simulink model "Simulation_in_Simulink"  (R2021b)
settings: Solver=FixedStepAuto  StartTime=0.0  StopTime=10  FixedStep=0.02  RelTol=1e-3
(part 2 of 5)

== matlab function Simulation_in_Simulink/C*theta_dot ==
  data: theta input; C_theta_dot output; theta_dot input
function C_theta_dot = fcn(theta,theta_dot)

t1=theta(1);
t2=theta(2);
t3=theta(3);
t4=theta(4);
t5=theta(5);
t6=theta(6);

td1=theta_dot(1);
td2=theta_dot(2);
td3=theta_dot(3);
td4=theta_dot(4);
td5=theta_dot(5);
td6=theta_dot(6);

a2=0.6129;
a3=0.5716; 
d4=0.16389; 
d5=0.1157; 
d6=0.0922;

c11=td5*((49450651*sin(2*t2 + 2*t3 + 2*t4 - t5))/500000000000 - (1966511423*sin(2*t2 + 2*t3 + 2*t4 - 2*t5))/20000000000000 + (1966511423*sin(2*t2 + 2*t3 + 2*t4 + 2*t5))/20000000000000 - (1966511423*sin(2*t5))/10000000000000 + (49450651*sin(2*t2 + 2*t3 + 2*t4 + t5))/500000000000 + (957929*a2*cos(2*t2 + t3 + t4 - t5))/200000000 + (957929*a3*cos(2*t2 + 2*t3 + t4 + t5))/200000000 - (((817*sin(t6)*(cos(t5)*sin(t1) + cos(t2 + t3 + t4)*cos(t1)*sin(t5)))/2000000 - (37539*sin(t1)*sin(t5))/5000000 + (43*d6*(sin(t1)*sin(t5) - cos(t2 + t3 + t4)*cos(t1)*cos(t5)))/100 + (37539*cos(t2 + t3 + t4)*cos(t1)*cos(t5))/5000000)*(d6*(cos(t5)*sin(t1) + cos(t2 + t3 + t4)*cos(t1)*sin(t5)) - (873*cos(t5)*sin(t1))/50000 - (19*sin(t6)*(sin(t1)*sin(t5) - cos(t2 + t3 + t4)*cos(t1)*cos(t5)))/20000 + d4*sin(t1) - (873*cos(t2 + t3 + t4)*cos(t1)*sin(t5))/50000 + (19*sin(t2 + t3 + t4)*cos(t1)*cos(t6))/20000 + a3*cos(t2 + t3)*cos(t1) + a2*cos(t1)*cos(t2) - d5*sin(t2 + t3 + t4)*cos(t1)))/2 - (((19*sin(t6)*(cos(t5)*sin(t1) + cos(t2 + t3 + t4)*cos(t1)*sin(t5)))/20000 - (873*sin(t1)*sin(t5))/50000 + d6*(sin(t1)*sin(t5) - cos(t2 + t3 + t4)*cos(t1)*cos(t5)) + (873*cos(t2 + t3 + t4)*cos(t1)*cos(t5))/50000)*((43*d6*(cos(t5)*sin(t1) + cos(t2 + t3 + t4)*cos(t1)*sin(t5)))/100 - (37539*cos(t5)*sin(t1))/5000000 - (817*sin(t6)*(sin(t1)*sin(t5) - cos(t2 + t3 + t4)*cos(t1)*cos(t5)))/2000000 + (43*d4*sin(t1))/100 - (37539*cos(t2 + t3 + t4)*cos(t1)*sin(t5))/5000000 + (817*sin(t2 + t3 + t4)*cos(t1)*cos(t6))/2000000 + (43*a3*cos(t2 + t3)*cos(t1))/100 + (43*a2*cos(t1)*cos(t2))/100 - (43*d5*sin(t2 + t3 + t4)*cos(t1))/100))/2 + (957929*a2*cos(t3 + t4 - t5))/200000000 + (((817*sin(t6)*(cos(t1)*cos(t5) - cos(t2 + t3 + t4)*sin(t1)*sin(t5)))/2000000 - (37539*cos(t1)*sin(t5))/5000000 + (43*d6*(cos(t1)*sin(t5) + cos(t2 + t3 + t4)*cos(t5)*sin(t1)))/100 - (37539*cos(t2 + t3 + t4)*cos(t5)*sin(t1))/5000000)*((19*sin(t6)*(cos(t1)*sin(t5) + cos(t2 + t3 + t4)*cos(t5)*sin(t1)))/20000 + (873*cos(t1)*cos(t5))/50000 - d6*(cos(t1)*cos(t5) - cos(t2 + t3 + t4)*sin(t1)*sin(t5)) - d4*cos(t1) - (873*cos(t2 + t3 + t4)*sin(t1)*sin(t5))/50000 + (19*sin(t2 + t3 + t4)*cos(t6)*sin(t1))/20000 + a3*cos(t2 + t3)*sin(t1) + a2*cos(t2)*sin(t1) - d5*sin(t2 + t3 + t4)*sin(t1)))/2 + (((19*sin(t6)*(cos(t1)*cos(t5) - cos(t2 + t3 + t4)*sin(t1)*sin(t5)))/20000 - (873*cos(t1)*sin(t5))/50000 + d6*(cos(t1)*sin(t5) + cos(t2 + t3 + t4)*cos(t5)*sin(t1)) - (873*cos(t2 + t3 + t4)*cos(t5)*sin(t1))/50000)*((817*sin(t6)*(cos(t1)*sin(t5) + cos(t2 + t3 + t4)*cos(t5)*sin(t1)))/2000000 + (37539*cos(t1)*cos(t5))/5000000 - (43*d6*(cos(t1)*cos(t5) - cos(t2 + t3 + t4)*sin(t1)*sin(t5)))/100 - (43*d4*cos(t1))/100 - (37539*cos(t2 + t3 + t4)*sin(t1)*sin(t5))/5000000 + (817*sin(t2 + t3 + t4)*cos(t6)*sin(t1))/2000000 + (43*a3*cos(t2 + t3)*sin(t1))/100 + (43*a2*cos(t2)*sin(t1))/100 - (43*d5*sin(t2 + t3 + t4)*sin(t1))/100))/2 + (957929*a3*cos(t4 + t5))/200000000 + (957929*a3*cos(2*t2 + 2*t3 + t4 - t5))/200000000 - (957929*d5*sin(2*t2 + 2*t3 + 2*t4 + t5))/200000000 - (957929*d4*sin(t5))/50000000 + (957929*a2*cos(2*t2 + t3 + t4 + t5))/200000000 + (957929*a3*cos(t4 - t5))/200000000 + (957929*a2*cos(t3 + t4 + t5))/200000000 - (957929*d5*sin(2*t2 + 2*t3 + 2*t4 - t5))/200000000 + (sin(t2 + t3 + t4)^2*cos(t5)*sin(t5))/2500 - (11*sin(t2 + t3 + t4)*cos(t6)*sin(t5)*(cos(t2 + t3 + t4)*sin(t6) + sin(t2 + t3 + t4)*cos(t5)*cos(t6)))/100000 - (sin(t2 + t3 + t4)*cos(t6)*sin(t5)*((11*cos(t2 + t3 + t4)*sin(t6))/50000 + (11*sin(t2 + t3 + t4)*cos(t5)*cos(t6))/50000))/2 + (3*sin(t2 + t3 + t4)*sin(t5)*sin(t6)*(cos(t2 + t3 + t4)*cos(t6) - sin(t2 + t3 + t4)*cos(t5)*sin(t6)))/25000 + (sin(t2 + t3 + t4)*sin(t5)*sin(t6)*((3*cos(t2 + t3 + t4)*cos(t6))/12500 - (3*sin(t2 + t3 + t4)*cos(t5)*sin(t6))/12500))/2) - td3*((49450651*sin(2*t2 + 2*t3 + 2*t4 - t5))/250000000000 - (1966511423*sin(2*t2 + 2*t3 + 2*t4 - 2*t5))/20000000000000 - (1966511423*sin(2*t2 + 2*t3 + 2*t4 + 2*t5))/20000000000000 - (3534581023*sin(2*t2 + 2*t3 + 2*t4))/10000000000000 + (42783*sin(2*t2 + 2*t3))/62500 - (49450651*sin(2*t2 + 2*t3 + 2*t4 + t5))/250000000000 + (37373*d5*sin(2*t2 + 2*t3 + 2*t4))/2500000 + (957929*a2*cos(2*t2 + t3 + t4 - t5))/200000000 - (957929*a3*cos(2*t2 + 2*t3 + t4 + t5))/100000000 + (210469*a2*cos(2*t2 + t3 + t4))/100000000 + (957929*a2*cos(t3 + t4 - t5))/200000000 + (((43*a3*sin(t2 + t3)*sin(t1))/100 - (37539*sin(t2 + t3 + t4)*sin(t1)*sin(t5))/5000000 - (817*cos(t2 + t3 + t4)*cos(t6)*sin(t1))/2000000 + (43*d5*cos(t2 + t3 + t4)*sin(t1))/100 + (817*sin(t2 + t3 + t4)*cos(t5)*sin(t1)*sin(t6))/2000000 + (43*d6*sin(t2 + t3 + t4)*sin(t1)*sin(t5))/100)*((19*sin(t6)*(cos(t1)*sin(t5) + cos(t2 + t3 + t4)*cos(t5)*sin(t1)))/20000 + (873*cos(t1)*cos(t5))/50000 - d6*(cos(t1)*cos(t5) - cos(t2 + t3 + t4)*sin(t1)*sin(t5)) - d4*cos(t1) - (873*cos(t2 + t3 + t4)*sin(t1)*sin(t5))/50000 + (19*sin(t2 + t3 + t4)*cos(t6)*sin(t1))/20000 + a3*cos(t2 + t3)*sin(t1) + a2*cos(t2)*sin(t1) - d5*sin(t2 + t3 + t4)*sin(t1)))/2 + ((a3*sin(t2 + t3)*sin(t1) - (873*sin(t2 + t3 + t4)*sin(t1)*sin(t5))/50000 - (19*cos(t2 + t3 + t4)*cos(t6)*sin(t1))/20000 + d5*cos(t2 + t3 + t4)*sin(t1) + (19*sin(t2 + t3 + t4)*cos(t5)*sin(t1)*sin(t6))/20000 + d6*sin(t2 + t3 + t4)*sin(t1)*sin(t5))*((817*sin(t6)*(cos(t1)*sin(t5) + cos(t2 + t3 + t4)*cos(t5)*sin(t1)))/2000000 + (37539*cos(t1)*cos(t5))/5000000 - (43*d6*(cos(t1)*cos(t5) - cos(t2 + t3 + t4)*sin(t1)*sin(t5)))/100 - (43*d4*cos(t1))/100 - (37539*cos(t2 + t3 + t4)*sin(t1)*sin(t5))/5000000 + (817*sin(t2 + t3 + t4)*cos(t6)*sin(t1))/2000000 + (43*a3*cos(t2 + t3)*sin(t1))/100 + (43*a2*cos(t2)*sin(t1))/100 - (43*d5*sin(t2 + t3 + t4)*sin(t1))/100))/2 + ((sin(t2 + t3 + t4)*cos(t6) + cos(t2 + t3 + t4)*cos(t5)*sin(t6))*((3*cos(t2 + t3 + t4)*cos(t6))/12500 - (3*sin(t2 + t3 + t4)*cos(t5)*sin(t6))/12500))/2 + ((cos(t2 + t3 + t4)*cos(t6) - sin(t2 + t3 + t4)*cos(t5)*sin(t6))*((3*sin(t2 + t3 + t4)*cos(t6))/12500 + (3*cos(t2 + t3 + t4)*cos(t5)*sin(t6))/12500))/2 + ((cos(t2 + t3 + t4)*sin(t6) + sin(t2 + t3 + t4)*cos(t5)*cos(t6))*((11*sin(t2 + t3 + t4)*sin(t6))/50000 - (11*cos(t2 + t3 + t4)*cos(t5)*cos(t6))/50000))/2 + ((sin(t2 + t3 + t4)*sin(t6) - cos(t2 + t3 + t4)*cos(t5)*cos(t6))*((11*cos(t2 + t3 + t4)*sin(t6))/50000 + (11*sin(t2 + t3 + t4)*cos(t5)*cos(t6))/50000))/2 + (210469*a2*cos(t3 + t4))/100000000 - (1967*d5^2*sin(2*t2 + 2*t3 + 2*t4))/2000 + (957929*a3*cos(2*t2 + 2*t3 + t4 - t5))/100000000 + (957929*d5*sin(2*t2 + 2*t3 + 2*t4 + t5))/100000000 + (1967*a3^2*sin(2*t2 + 2*t3))/1000 + (210469*a3*cos(2*t2 + 2*t3 + t4))/50000000 + (2041*a2*sin(t3))/1250 - (957929*a2*cos(2*t2 + t3 + t4 + t5))/200000000 + (((43*a3*sin(t2 + t3)*cos(t1))/100 - (37539*sin(t2 + t3 + t4)*cos(t1)*sin(t5))/5000000 - (817*cos(t2 + t3 + t4)*cos(t1)*cos(t6))/2000000 + (43*d5*cos(t2 + t3 + t4)*cos(t1))/100 + (817*sin(t2 + t3 + t4)*cos(t1)*cos(t5)*sin(t6))/2000000 + (43*d6*sin(t2 + t3 + t4)*cos(t1)*sin(t5))/100)*(d6*(cos(t5)*sin(t1) + cos(t2 + t3 + t4)*cos(t1)*sin(t5)) - (873*cos(t5)*sin(t1))/50000 - (19*sin(t6)*(sin(t1)*sin(t5) - cos(t2 + t3 + t4)*cos(t1)*cos(t5)))/20000 + d4*sin(t1) - (873*cos(t2 + t3 + t4)*cos(t1)*sin(t5))/50000 + (19*sin(t2 + t3 + t4)*cos(t1)*cos(t6))/20000 + a3*cos(t2 + t3)*cos(t1) + a2*cos(t1)*cos(t2) - d5*sin(t2 + t3 + t4)*cos(t1)))/2 + ((a3*sin(t2 + t3)*cos(t1) - (873*sin(t2 + t3 + t4)*cos(t1)*sin(t5))/50000 - (19*cos(t2 + t3 + t4)*cos(t1)*cos(t6))/20000 + d5*cos(t2 + t3 + t4)*cos(t1) + (19*sin(t2 + t3 + t4)*cos(t1)*cos(t5)*sin(t6))/20000 + d6*sin(t2 + t3 + t4)*cos(t1)*sin(t5))*((43*d6*(cos(t5)*sin(t1) + cos(t2 + t3 + t4)*cos(t1)*sin(t5)))/100 - (37539*cos(t5)*sin(t1))/5000000 - (817*sin(t6)*(sin(t1)*sin(t5) - cos(t2 + t3 + t4)*cos(t1)*cos(t5)))/2000000 + (43*d4*sin(t1))/100 - (37539*cos(t2 + t3 + t4)*cos(t1)*sin(t5))/5000000 + (817*sin(t2 + t3 + t4)*cos(t1)*cos(t6))/2000000 + (43*a3*cos(t2 + t3)*cos(t1))/100 + (43*a2*cos(t1)*cos(t2))/100 - (43*d5*sin(t2 + t3 + t4)*cos(t1))/100))/2 + (2041*a2*sin(2*t2 + t3))/1250 - (957929*a2*cos(t3 + t4 + t5))/200000000 - (957929*d5*sin(2*t2 + 2*t3 + 2*t4 - t5))/100000000 + (1967*a3*d5*cos(2*t2 + 2*t3 + t4))/1000 + (1967*a2*a3*sin(t3))/1000 + (1967*a2*a3*sin(2*t2 + t3))/1000 + (1967*a2*d5*cos(2*t2 + t3 + t4))/2000 + (1967*a2*d5*cos(t3 + t4))/2000 - (cos(t2 + t3 + t4)*sin(t2 + t3 + t4)*sin(t5)^2)/2500) - td4*((49450651*sin(2*t2 + 2*t3 + 2*t4 - t5))/250000000000 - (1966511423*sin(2*t2 + 2*t3 + 2*t4 - 2*t5))/20000000000000 - (1966511423*sin(2*t2 + 2*t3 + 2*t4 + 2*t5))/20000000000000 - (3534581023*sin(2*t2 + 2*t3 + 2*t4))/10000000000000 - (49450651*sin(2*t2 + 2*t3 + 2*t4 + t5))/250000000000 + (37373*d5*sin(2*t2 + 2*t3 + 2*t4))/2500000 + (957929*a2*cos(2*t2 + t3 + t4 - t5))/200000000 - (957929*a3*cos(2*t2 + 2*t3 + t4 + t5))/200000000 + (210469*a2*cos(2*t2 + t3 + t4))/100000000 + (957929*a2*cos(t3 + t4 - t5))/200000000 + ((sin(t2 + t3 + t4)*cos(t6) + cos(t2 + t3 + t4)*cos(t5)*sin(t6))*((3*cos(t2 + t3 + t4)*cos(t6))/12500 - (3*sin(t2 + t3 + t4)*cos(t5)*sin(t6))/12500))/2 + ((cos(t2 + t3 + t4)*cos(t6) - sin(t2 + t3 + t4)*cos(t5)*sin(t6))*((3*sin(t2 + t3 + t4)*cos(t6))/12500 + (3*cos(t2 + t3 + t4)*cos(t5)*sin(t6))/12500))/2 + ((cos(t2 + t3 + t4)*sin(t6) + sin(t2 + t3 + t4)*cos(t5)*cos(t6))*((11*sin(t2 + t3 + t4)*sin(t6))/50000 - (11*cos(t2 + t3 + t4)*cos(t5)*cos(t6))/50000))/2 + ((sin(t2 + t3 + t4)*sin(t6) - cos(t2 + t3 + t4)*cos(t5)*cos(t6))*((11*cos(t2 + t3 + t4)*sin(t6))/50000 + (11*sin(t2 + t3 + t4)*cos(t5)*cos(t6))/50000))/2 + (((43*d5*cos(t2 + t3 + t4)*cos(t1))/100 - (37539*sin(t2 + t3 + t4)*cos(t1)*sin(t5))/5000000 - (817*cos(t2 + t3 + t4)*cos(t1)*cos(t6))/2000000 + (817*sin(t2 + t3 + t4)*cos(t1)*cos(t5)*sin(t6))/2000000 + (43*d6*sin(t2 + t3 + t4)*cos(t1)*sin(t5))/100)*(d6*(cos(t5)*sin(t1) + cos(t2 + t3 + t4)*cos(t1)*sin(t5)) - (873*cos(t5)*sin(t1))/50000 - (19*sin(t6)*(sin(t1)*sin(t5) - cos(t2 + t3 + t4)*cos(t1)*cos(t5)))/20000 + d4*sin(t1) - (873*cos(t2 + t3 + t4)*cos(t1)*sin(t5))/50000 + (19*sin(t2 + t3 + t4)*cos(t1)*cos(t6))/20000 + a3*cos(t2 + t3)*cos(t1) + a2*cos(t1)*cos(t2) - d5*sin(t2 + t3 + t4)*cos(t1)))/2 + ((d5*cos(t2 + t3 + t4)*cos(t1) - (873*sin(t2 + t3 + t4)*cos(t1)*sin(t5))/50000 - (19*cos(t2 + t3 + t4)*cos(t1)*cos(t6))/20000 + (19*sin(t2 + t3 + t4)*cos(t1)*cos(t5)*sin(t6))/20000 + d6*sin(t2 + t3 + t4)*cos(t1)*sin(t5))*((43*d6*(cos(t5)*sin(t1) + cos(t2 + t3 + t4)*cos(t1)*sin(t5)))/100 - (37539*cos(t5)*sin(t1))/5000000 - (817*sin(t6)*(sin(t1)*sin(t5) - cos(t2 + t3 + t4)*cos(t1)*cos(t5)))/2000000 + (43*d4*sin(t1))/100 - (37539*cos(t2 + t3 + t4)*cos(t1)*sin(t5))/5000000 + (817*sin(t2 + t3 + t4)*cos(t1)*cos(t6))/2000000 + (43*a3*cos(t2 + t3)*cos(t1))/100 + (43*a2*cos(t1)*cos(t2))/100 - (43*d5*sin(t2 + t3 + t4)*cos(t1))/100))/2 + (210469*a2*cos(t3 + t4))/100000000 - (957929*a3*cos(t4 + t5))/200000000 - (1967*d5^2*sin(2*t2 + 2*t3 + 2*t4))/2000 + (957929*a3*cos(2*t2 + 2*t3 + t4 - t5))/200000000 + (957929*d5*sin(2*t2 + 2*t3 + 2*t4 + t5))/100000000 + (210469*a3*cos(t4))/100000000 + (210469*a3*cos(2*t2 + 2*t3 + t4))/100000000 - (957929*a2*cos(2*t2 + t3 + t4 + t5))/200000000 + (957929*a3*cos(t4 - t5))/200000000 - (957929*a2*cos(t3 + t4 + t5))/200000000 - (957929*d5*sin(2*t2 + 2*t3 + 2*t4 - t5))/100000000 + (((43*d5*cos(t2 + t3 + t4)*sin(t1))/100 - (37539*sin(t2 + t3 + t4)*sin(t1)*sin(t5))/5000000 - (817*cos(t2 + t3 + t4)*cos(t6)*sin(t1))/2000000 + (817*sin(t2 + t3 + t4)*cos(t5)*sin(t1)*sin(t6))/2000000 + (43*d6*sin(t2 + t3 + t4)*sin(t1)*sin(t5))/100)*((19*sin(t6)*(cos(t1)*sin(t5) + cos(t2 + t3 + t4)*cos(t5)*sin(t1)))/20000 + (873*cos(t1)*cos(t5))/50000 - d6*(cos(t1)*cos(t5) - cos(t2 + t3 + t4)*sin(t1)*sin(t5)) - d4*cos(t1) - (873*cos(t2 + t3 + t4)*sin(t1)*sin(t5))/50000 + (19*sin(t2 + t3 + t4)*cos(t6)*sin(t1))/20000 + a3*cos(t2 + t3)*sin(t1) + a2*cos(t2)*sin(t1) - d5*sin(t2 + t3 + t4)*sin(t1)))/2 + ((d5*cos(t2 + t3 + t4)*sin(t1) - (873*sin(t2 + t3 + t4)*sin(t1)*sin(t5))/50000 - (19*cos(t2 + t3 + t4)*cos(t6)*sin(t1))/20000 + (19*sin(t2 + t3 + t4)*cos(t5)*sin(t1)*sin(t6))/20000 + d6*sin(t2 + t3 + t4)*sin(t1)*sin(t5))*((817*sin(t6)*(cos(t1)*sin(t5) + cos(t2 + t3 + t4)*cos(t5)*sin(t1)))/2000000 + (37539*cos(t1)*cos(t5))/5000000 - (43*d6*(cos(t1)*cos(t5) - cos(t2 + t3 + t4)*sin(t1)*sin(t5)))/100 - (43*d4*cos(t1))/100 - (37539*cos(t2 + t3 + t4)*sin(t1)*sin(t5))/5000000 + (817*sin(t2 + t3 + t4)*cos(t6)*sin(t1))/2000000 + (43*a3*cos(t2 + t3)*sin(t1))/100 + (43*a2*cos(t2)*sin(t1))/100 - (43*d5*sin(t2 + t3 + t4)*sin(t1))/100))/2 + (1967*a3*d5*cos(2*t2 + 2*t3 + t4))/2000 + (1967*a2*d5*cos(2*t2 + t3 + t4))/2000 + (1967*a2*d5*cos(t3 + t4))/2000 - (cos(t2 + t3 + t4)*sin(t2 + t3 + t4)*sin(t5)^2)/2500 + (1967*a3*d5*cos(t4))/2000) - td6*(((cos(t2 + t3 + t4)*sin(t6) + sin(t2 + t3 + t4)*cos(t5)*cos(t6))*((3*cos(t2 + t3 + t4)*cos(t6))/12500 - (3*sin(t2 + t3 + t4)*cos(t5)*sin(t6))/12500))/2 + ((cos(t2 + t3 + t4)*cos(t6) - sin(t2 + t3 + t4)*cos(t5)*sin(t6))*((3*cos(t2 + t3 + t4)*sin(t6))/12500 + (3*sin(t2 + t3 + t4)*cos(t5)*cos(t6))/12500))/2 - ((cos(t2 + t3 + t4)*sin(t6) + sin(t2 + t3 + t4)*cos(t5)*cos(t6))*((11*cos(t2 + t3 + t4)*cos(t6))/50000 - (11*sin(t2 + t3 + t4)*cos(t5)*sin(t6))/50000))/2 - ((cos(t2 + t3 + t4)*cos(t6) - sin(t2 + t3 + t4)*cos(t5)*sin(t6))*((11*cos(t2 + t3 + t4)*sin(t6))/50000 + (11*sin(t2 + t3 + t4)*cos(t5)*cos(t6))/50000))/2 + (((817*cos(t6)*(sin(t1)*sin(t5) - cos(t2 + t3 + t4)*cos(t1)*cos(t5)))/2000000 + (817*sin(t2 + t3 + t4)*cos(t1)*sin(t6))/2000000)*(d6*(cos(t5)*sin(t1) + cos(t2 + t3 + t4)*cos(t1)*sin(t5)) - (873*cos(t5)*sin(t1))/50000 - (19*sin(t6)*(sin(t1)*sin(t5) - cos(t2 + t3 + t4)*cos(t1)*cos(t5)))/20000 + d4*sin(t1) - (873*cos(t2 + t3 + t4)*cos(t1)*sin(t5))/50000 + (19*sin(t2 + t3 + t4)*cos(t1)*cos(t6))/20000 + a3*cos(t2 + t3)*cos(t1) + a2*cos(t1)*cos(t2) - d5*sin(t2 + t3 + t4)*cos(t1)))/2 + (((19*cos(t6)*(sin(t1)*sin(t5) - cos(t2 + t3 + t4)*cos(t1)*cos(t5)))/20000 + (19*sin(t2 + t3 + t4)*cos(t1)*sin(t6))/20000)*((43*d6*(cos(t5)*sin(t1) + cos(t2 + t3 + t4)*cos(t1)*sin(t5)))/100 - (37539*cos(t5)*sin(t1))/5000000 - (817*sin(t6)*(sin(t1)*sin(t5) - cos(t2 + t3 + t4)*cos(t1)*cos(t5)))/2000000 + (43*d4*sin(t1))/100 - (37539*cos(t2 + t3 + t4)*cos(t1)*sin(t5))/5000000 + (817*sin(t2 + t3 + t4)*cos(t1)*cos(t6))/2000000 + (43*a3*cos(t2 + t3)*cos(t1))/100 + (43*a2*cos(t1)*cos(t2))/100 - (43*d5*sin(t2 + t3 + t4)*cos(t1))/100))/2 - (((817*cos(t6)*(cos(t1)*sin(t5) + cos(t2 + t3 + t4)*cos(t5)*sin(t1)))/2000000 - (817*sin(t2 + t3 + t4)*sin(t1)*sin(t6))/2000000)*((19*sin(t6)*(cos(t1)*sin(t5) + cos(t2 + t3 + t4)*cos(t5)*sin(t1)))/20000 + (873*cos(t1)*cos(t5))/50000 - d6*(cos(t1)*cos(t5) - cos(t2 + t3 + t4)*sin(t1)*sin(t5)) - d4*cos(t1) - (873*cos(t2 + t3 + t4)*sin(t1)*sin(t5))/50000 + (19*sin(t2 + t3 + t4)*cos(t6)*sin(t1))/20000 + a3*cos(t2 + t3)*sin(t1) + a2*cos(t2)*sin(t1) - d5*sin(t2 + t3 + t4)*sin(t1)))/2 - (((19*cos(t6)*(cos(t1)*sin(t5) + cos(t2 + t3 + t4)*cos(t5)*sin(t1)))/20000 - (19*sin(t2 + t3 + t4)*sin(t1)*sin(t6))/20000)*((817*sin(t6)*(cos(t1)*sin(t5) + cos(t2 + t3 + t4)*cos(t5)*sin(t1)))/2000000 + (37539*cos(t1)*cos(t5))/5000000 - (43*d6*(cos(t1)*cos(t5) - cos(t2 + t3 + t4)*sin(t1)*sin(t5)))/100 - (43*d4*cos(t1))/100 - (37539*cos(t2 + t3 + t4)*sin(t1)*sin(t5))/5000000 + (817*sin(t2 + t3 + t4)*cos(t6)*sin(t1))/2000000 + (43*a3*cos(t2 + t3)*sin(t1))/100 + (43*a2*cos(t2)*sin(t1))/100 - (43*d5*sin(t2 + t3 + t4)*sin(t1))/100))/2) - td2*((49450651*sin(2*t2 + 2*t3 + 2*t4 - t5))/250000000000 - (1966511423*sin(2*t2 + 2*t3 + 2*t4 - 2*t5))/20000000000000 - (1966511423*sin(2*t2 + 2*t3 + 2*t4 + 2*t5))/20000000000000 + (53*sin(2*t2))/40 - (3534581023*sin(2*t2 + 2*t3 + 2*t4))/10000000000000 + (42783*sin(2*t2 + 2*t3))/62500 - (49450651*sin(2*t2 + 2*t3 + 2*t4 + t5))/250000000000 + (37373*d5*sin(2*t2 + 2*t3 + 2*t4))/2500000 + (957929*a2*cos(2*t2 + t3 + t4 - t5))/100000000 - (957929*a3*cos(2*t2 + 2*t3 + t4 + t5))/100000000 + (((43*a3*sin(t2 + t3)*cos(t1))/100 - (37539*sin(t2 + t3 + t4)*cos(t1)*sin(t5))/5000000 - (817*cos(t2 + t3 + t4)*cos(t1)*cos(t6))/2000000 + (43*a2*cos(t1)*sin(t2))/100 + (43*d5*cos(t2 + t3 + t4)*cos(t1))/100 + (817*sin(t2 + t3 + t4)*cos(t1)*cos(t5)*sin(t6))/2000000 + (43*d6*sin(t2 + t3 + t4)*cos(t1)*sin(t5))/100)*(d6*(cos(t5)*sin(t1) + cos(t2 + t3 + t4)*cos(t1)*sin(t5)) - (873*cos(t5)*sin(t1))/50000 - (19*sin(t6)*(sin(t1)*sin(t5) - cos(t2 + t3 + t4)*cos(t1)*cos(t5)))/20000 + d4*sin(t1) - (873*cos(t2 + t3 + t4)*cos(t1)*sin(t5))/50000 + (19*sin(t2 + t3 + t4)*cos(t1)*cos(t6))/20000 + a3*cos(t2 + t3)*cos(t1) + a2*cos(t1)*cos(t2) - d5*sin(t2 + t3 + t4)*cos(t1)))/2 + ((a3*sin(t2 + t3)*cos(t1) - (873*sin(t2 + t3 + t4)*cos(t1)*sin(t5))/50000 - (19*cos(t2 + t3 + t4)*cos(t1)*cos(t6))/20000 + a2*cos(t1)*sin(t2) + d5*cos(t2 + t3 + t4)*cos(t1) + (19*sin(t2 + t3 + t4)*cos(t1)*cos(t5)*sin(t6))/20000 + d6*sin(t2 + t3 + t4)*cos(t1)*sin(t5))*((43*d6*(cos(t5)*sin(t1) + cos(t2 + t3 + t4)*cos(t1)*sin(t5)))/100 - (37539*cos(t5)*sin(t1))/5000000 - (817*sin(t6)*(sin(t1)*sin(t5) - cos(t2 + t3 + t4)*cos(t1)*cos(t5)))/2000000 + (43*d4*sin(t1))/100 - (37539*cos(t2 + t3 + t4)*cos(t1)*sin(t5))/5000000 + (817*sin(t2 + t3 + t4)*cos(t1)*cos(t6))/2000000 + (43*a3*cos(t2 + t3)*cos(t1))/100 + (43*a2*cos(t1)*cos(t2))/100 - (43*d5*sin(t2 + t3 + t4)*cos(t1))/100))/2 + (210469*a2*cos(2*t2 + t3 + t4))/50000000 + ((sin(t2 + t3 + t4)*cos(t6) + cos(t2 + t3 + t4)*cos(t5)*sin(t6))*((3*cos(t2 + t3 + t4)*cos(t6))/12500 - (3*sin(t2 + t3 + t4)*cos(t5)*sin(t6))/12500))/2 + ((cos(t2 + t3 + t4)*cos(t6) - sin(t2 + t3 + t4)*cos(t5)*sin(t6))*((3*sin(t2 + t3 + t4)*cos(t6))/12500 + (3*cos(t2 + t3 + t4)*cos(t5)*sin(t6))/12500))/2 + ((cos(t2 + t3 + t4)*sin(t6) + sin(t2 + t3 + t4)*cos(t5)*cos(t6))*((11*sin(t2 + t3 + t4)*sin(t6))/50000 - (11*cos(t2 + t3 + t4)*cos(t5)*cos(t6))/50000))/2 + ((sin(t2 + t3 + t4)*sin(t6) - cos(t2 + t3 + t4)*cos(t5)*cos(t6))*((11*cos(t2 + t3 + t4)*sin(t6))/50000 + (11*sin(t2 + t3 + t4)*cos(t5)*cos(t6))/50000))/2 + (8247*a2^2*sin(2*t2))/1000 - (1967*d5^2*sin(2*t2 + 2*t3 + 2*t4))/2000 + (957929*a3*cos(2*t2 + 2*t3 + t4 - t5))/100000000 + (957929*d5*sin(2*t2 + 2*t3 + 2*t4 + t5))/100000000 + (1967*a3^2*sin(2*t2 + 2*t3))/1000 + (210469*a3*cos(2*t2 + 2*t3 + t4))/50000000 - (957929*a2*cos(2*t2 + t3 + t4 + t5))/100000000 + (((43*a3*sin(t2 + t3)*sin(t1))/100 - (37539*sin(t2 + t3 + t4)*sin(t1)*sin(t5))/5000000 - (817*cos(t2 + t3 + t4)*cos(t6)*sin(t1))/2000000 + (43*a2*sin(t1)*sin(t2))/100 + (43*d5*cos(t2 + t3 + t4)*sin(t1))/100 + (817*sin(t2 + t3 + t4)*cos(t5)*sin(t1)*sin(t6))/2000000 + (43*d6*sin(t2 + t3 + t4)*sin(t1)*sin(t5))/100)*((19*sin(t6)*(cos(t1)*sin(t5) + cos(t2 + t3 + t4)*cos(t5)*sin(t1)))/20000 + (873*cos(t1)*cos(t5))/50000 - d6*(cos(t1)*cos(t5) - cos(t2 + t3 + t4)*sin(t1)*sin(t5)) - d4*cos(t1) - (873*cos(t2 + t3 + t4)*sin(t1)*sin(t5))/50000 + (19*sin(t2 + t3 + t4)*cos(t6)*sin(t1))/20000 + a3*cos(t2 + t3)*sin(t1) + a2*cos(t2)*sin(t1) - d5*sin(t2 + t3 + t4)*sin(t1)))/2 + ((a3*sin(t2 + t3)*sin(t1) - (873*sin(t2 + t3 + t4)*sin(t1)*sin(t5))/50000 - (19*cos(t2 + t3 + t4)*cos(t6)*sin(t1))/20000 + a2*sin(t1)*sin(t2) + d5*cos(t2 + t3 + t4)*sin(t1) + (19*sin(t2 + t3 + t4)*cos(t5)*sin(t1)*sin(t6))/20000 + d6*sin(t2 + t3 + t4)*sin(t1)*sin(t5))*((817*sin(t6)*(cos(t1)*sin(t5) + cos(t2 + t3 + t4)*cos(t5)*sin(t1)))/2000000 + (37539*cos(t1)*cos(t5))/5000000 - (43*d6*(cos(t1)*cos(t5) - cos(t2 + t3 + t4)*sin(t1)*sin(t5)))/100 - (43*d4*cos(t1))/100 - (37539*cos(t2 + t3 + t4)*sin(t1)*sin(t5))/5000000 + (817*sin(t2 + t3 + t4)*cos(t6)*sin(t1))/2000000 + (43*a3*cos(t2 + t3)*sin(t1))/100 + (43*a2*cos(t2)*sin(t1))/100 - (43*d5*sin(t2 + t3 + t4)*sin(t1))/100))/2 + (2041*a2*sin(2*t2 + t3))/625 - (957929*d5*sin(2*t2 + 2*t3 + 2*t4 - t5))/100000000 + (1967*a3*d5*cos(2*t2 + 2*t3 + t4))/1000 + (1967*a2*a3*sin(2*t2 + t3))/500 + (1967*a2*d5*cos(2*t2 + t3 + t4))/1000 - (cos(t2 + t3 + t4)*sin(t2 + t3 + t4)*sin(t5)^2)/2500);

c12=td4*((7474967197*sin(t2 + t3 + t4 - 2*t5))/40000000000000 - (49450651*sin(t2 + t3 + t4 - t5))/250000000000 - (7474967197*sin(t2 + t3 + t4 + 2*t5))/40000000000000 + (713241*sin(t2 + t3 + t4 + t5 + t6))/400000000000 - (49450651*sin(t2 + t3 + t4))/125000000000 + (713241*sin(t2 + t3 + t4 + t5 - t6))/400000000000 + (713241*sin(t2 + t3 + t4 - t5 + t6))/400000000000 - (784477*sin(t2 + t3 + t4 + t5 - 2*t6))/320000000000 + (784477*sin(t2 + t3 + t4 + t5 + 2*t6))/320000000000 + (713241*sin(t2 + t3 + t4 - 2*t5 + t6))/400000000000 + (713241*sin(t2 + t3 + t4 + 2*t5 + t6))/400000000000 - (49450651*sin(t2 + t3 + t4 + t5))/250000000000 + (713241*sin(t2 + t3 + t4 - t5 - t6))/400000000000 + (784477*sin(t2 + t3 + t4 - t5 - 2*t6))/320000000000 - (784477*sin(t2 + t3 + t4 - t5 + 2*t6))/320000000000 - (713241*sin(t2 + t3 + t4 - 2*t5 - t6))/400000000000 - (713241*sin(t2 + t3 + t4 + 2*t5 - t6))/400000000000 - (784477*sin(t2 + t3 + t4 - 2*t5 - 2*t6))/640000000000 - (784477*sin(t2 + t3 + t4 - 2*t5 + 2*t6))/640000000000 + (784477*sin(t2 + t3 + t4 + 2*t5 - 2*t6))/640000000000 + (784477*sin(t2 + t3 + t4 + 2*t5 + 2*t6))/640000000000 + (43*d6^2*sin(t2 + t3 + t4 - 2*t5))/400 - (43*d6^2*sin(t2 + t3 + t4 + 2*t5))/400 + (817*d4*sin(t2 + t3 + t4 + t5 - t6))/8000000 - (817*d4*sin(t2 + t3 + t4 - t5 + t6))/8000000 - (817*d5*sin(t2 + t3 + t4 + t5 - t6))/8000000 - (817*d5*sin(t2 + t3 + t4 - t5 + t6))/8000000 - (817*d6*sin(t2 + t3 + t4 + t5 - t6))/8000000 - (817*d6*sin(t2 + t3 + t4 - t5 + t6))/8000000 - (817*d6*sin(t2 + t3 + t4 - 2*t5 + t6))/8000000 - (817*d6*sin(t2 + t3 + t4 + 2*t5 + t6))/8000000 - (582539*d4*sin(t2 + t3 + t4 + t5))/100000000 - (817*d4*sin(t2 + t3 + t4 + t6))/4000000 + (582539*d5*sin(t2 + t3 + t4 + t5))/100000000 + (817*d4*sin(t2 + t3 + t4 - t5 - t6))/8000000 + (817*d5*sin(t2 + t3 + t4 - t5 - t6))/8000000 - (817*d6*sin(t2 + t3 + t4 - t5 - t6))/8000000 + (817*d6*sin(t2 + t3 + t4 - 2*t5 - t6))/8000000 + (817*d6*sin(t2 + t3 + t4 + 2*t5 - t6))/8000000 + (582539*d4*sin(t2 + t3 + t4 - t5))/100000000 - (817*d4*sin(t2 + t3 + t4 - t6))/4000000 + (582539*d5*sin(t2 + t3 + t4 - t5))/100000000 - (37539*d6*sin(t2 + t3 + t4 - 2*t5))/10000000 + (37539*d6*sin(t2 + t3 + t4 + 2*t5))/10000000 - (817*d4*sin(t2 + t3 + t4 + t5 + t6))/8000000 + (817*d5*sin(t2 + t3 + t4 + t5 + t6))/8000000 - (817*d6*sin(t2 + t3 + t4 + t5 + t6))/8000000 + (210469*d4*sin(t2 + t3 + t4))/50000000 + (43*d4*d6*sin(t2 + t3 + t4 - t5))/200 + (43*d5*d6*sin(t2 + t3 + t4 - t5))/200 + (2397*d4*d5*sin(t2 + t3 + t4))/1000 - (43*d4*d6*sin(t2 + t3 + t4 + t5))/200 + (43*d5*d6*sin(t2 + t3 + t4 + t5))/200) - td1*((49450651*sin(2*t2 + 2*t3 + 2*t4 - t5))/250000000000 - (1966511423*sin(2*t2 + 2*t3 + 2*t4 - 2*t5))/20000000000000 - (1966511423*sin(2*t2 + 2*t3 + 2*t4 + 2*t5))/20000000000000 + (53*sin(2*t2))/40 - (3534581023*sin(2*t2 + 2*t3 + 2*t4))/10000000000000 + (42783*sin(2*t2 + 2*t3))/62500 - (49450651*sin(2*t2 + 2*t3 + 2*t4 + t5))/250000000000 + (37373*d5*sin(2*t2 + 2*t3 + 2*t4))/2500000 + (957929*a2*cos(2*t2 + t3 + t4 - t5))/100000000 - (957929*a3*cos(2*t2 + 2*t3 + t4 + t5))/100000000 + (((43*a3*sin(t2 + t3)*cos(t1))/100 - (37539*sin(t2 + t3 + t4)*cos(t1)*sin(t5))/5000000 - (817*cos(t2 + t3 + t4)*cos(t1)*cos(t6))/2000000 + (43*a2*cos(t1)*sin(t2))/100 + (43*d5*cos(t2 + t3 + t4)*cos(t1))/100 + (817*sin(t2 + t3 + t4)*cos(t1)*cos(t5)*sin(t6))/2000000 + (43*d6*sin(t2 + t3 + t4)*cos(t1)*sin(t5))/100)*(d6*(cos(t5)*sin(t1) + cos(t2 + t3 + t4)*cos(t1)*sin(t5)) - (873*cos(t5)*sin(t1))/50000 - (19*sin(t6)*(sin(t1)*sin(t5) - cos(t2 + t3 + t4)*cos(t1)*cos(t5)))/20000 + d4*sin(t1) - (873*cos(t2 + t3 + t4)*cos(t1)*sin(t5))/50000 + (19*sin(t2 + t3 + t4)*cos(t1)*cos(t6))/20000 + a3*cos(t2 + t3)*cos(t1) + a2*cos(t1)*cos(t2) - d5*sin(t2 + t3 + t4)*cos(t1)))/2 + ((a3*sin(t2 + t3)*cos(t1) - (873*sin(t2 + t3 + t4)*cos(t1)*sin(t5))/50000 - (19*cos(t2 + t3 + t4)*cos(t1)*cos(t6))/20000 + a2*cos(t1)*sin(t2) + d5*cos(t2 + t3 + t4)*cos(t1) + (19*sin(t2 + t3 + t4)*cos(t1)*cos(t5)*sin(t6))/20000 + d6*sin(t2 + t3 + t4)*cos(t1)*sin(t5))*((43*d6*(cos(t5)*sin(t1) + cos(t2 + t3 + t4)*cos(t1)*sin(t5)))/100 - (37539*cos(t5)*sin(t1))/5000000 - (817*sin(t6)*(sin(t1)*sin(t5) - cos(t2 + t3 + t4)*cos(t1)*cos(t5)))/2000000 + (43*d4*sin(t1))/100 - (37539*cos(t2 + t3 + t4)*cos(t1)*sin(t5))/5000000 + (817*sin(t2 + t3 + t4)*cos(t1)*cos(t6))/2000000 + (43*a3*cos(t2 + t3)*cos(t1))/100 + (43*a2*cos(t1)*cos(t2))/100 - (43*d5*sin(t2 + t3 + t4)*cos(t1))/100))/2 + (210469*a2*cos(2*t2 + t3 + t4))/50000000 + ((sin(t2 + t3 + t4)*cos(t6) + cos(t2 + t3 + t4)*cos(t5)*sin(t6))*((3*cos(t2 + t3 + t4)*cos(t6))/12500 - (3*sin(t2 + t3 + t4)*cos(t5)*sin(t6))/12500))/2 + ((cos(t2 + t3 + t4)*cos(t6) - sin(t2 + t3 + t4)*cos(t5)*sin(t6))*((3*sin(t2 + t3 + t4)*cos(t6))/12500 + (3*cos(t2 + t3 + t4)*cos(t5)*sin(t6))/12500))/2 + ((cos(t2 + t3 + t4)*sin(t6) + sin(t2 + t3 + t4)*cos(t5)*cos(t6))*((11*sin(t2 + t3 + t4)*sin(t6))/50000 - (11*cos(t2 + t3 + t4)*cos(t5)*cos(t6))/50000))/2 + ((sin(t2 + t3 + t4)*sin(t6) - cos(t2 + t3 + t4)*cos(t5)*cos(t6))*((11*cos(t2 + t3 + t4)*sin(t6))/50000 + (11*sin(t2 + t3 + t4)*cos(t5)*cos(t6))/50000))/2 + (8247*a2^2*sin(2*t2))/1000 - (1967*d5^2*sin(2*t2 + 2*t3 + 2*t4))/2000 + (957929*a3*cos(2*t2 + 2*t3 + t4 - t5))/100000000 + (957929*d5*sin(2*t2 + 2*t3 + 2*t4 + t5))/100000000 + (1967*a3^2*sin(2*t2 + 2*t3))/1000 + (210469*a3*cos(2*t2 + 2*t3 + t4))/50000000 - (957929*a2*cos(2*t2 + t3 + t4 + t5))/100000000 + (((43*a3*sin(t2 + t3)*sin(t1))/100 - (37539*sin(t2 + t3 + t4)*sin(t1)*sin(t5))/5000000 - (817*cos(t2 + t3 + t4)*cos(t6)*sin(t1))/2000000 + (43*a2*sin(t1)*sin(t2))/100 + (43*d5*cos(t2 + t3 + t4)*sin(t1))/100 + (817*sin(t2 + t3 + t4)*cos(t5)*sin(t1)*sin(t6))/2000000 + (43*d6*sin(t2 + t3 + t4)*sin(t1)*sin(t5))/100)*((19*sin(t6)*(cos(t1)*sin(t5) + cos(t2 + t3 + t4)*cos(t5)*sin(t1)))/20000 + (873*cos(t1)*cos(t5))/50000 - d6*(cos(t1)*cos(t5) - cos(t2 + t3 + t4)*sin(t1)*sin(t5)) - d4*cos(t1) - (873*cos(t2 + t3 + t4)*sin(t1)*sin(t5))/50000 + (19*sin(t2 + t3 + t4)*cos(t6)*sin(t1))/20000 + a3*cos(t2 + t3)*sin(t1) + a2*cos(t2)*sin(t1) - d5*sin(t2 + t3 + t4)*sin(t1)))/2 + ((a3*sin(t2 + t3)*sin(t1) - (873*sin(t2 + t3 + t4)*sin(t1)*sin(t5))/50000 - (19*cos(t2 + t3 + t4)*cos(t6)*sin(t1))/20000 + a2*sin(t1)*sin(t2) + d5*cos(t2 + t3 + t4)*sin(t1) + (19*sin(t2 + t3 + t4)*cos(t5)*sin(t1)*sin(t6))/20000 + d6*sin(t2 + t3 + t4)*sin(t1)*sin(t5))*((817*sin(t6)*(cos(t1)*sin(t5) + cos(t2 + t3 + t4)*cos(t5)*sin(t1)))/2000000 + (37539*cos(t1)*cos(t5))/5000000 - (43*d6*(cos(t1)*cos(t5) - cos(t2 + t3 + t4)*sin(t1)*sin(t5)))/100 - (43*d4*cos(t1))/100 - (37539*cos(t2 + t3 + t4)*sin(t1)*sin(t5))/5000000 + (817*sin(t2 + t3 + t4)*cos(t6)*sin(t1))/2000000 + (43*a3*cos(t2 + t3)*sin(t1))/100 + (43*a2*cos(t2)*sin(t1))/100 - (43*d5*sin(t2 + t3 + t4)*sin(t1))/100))/2 + (2041*a2*sin(2*t2 + t3))/625 - (957929*d5*sin(2*t2 + 2*t3 + 2*t4 - t5))/100000000 + (1967*a3*d5*cos(2*t2 + 2*t3 + t4))/1000 + (1967*a2*a3*sin(2*t2 + t3))/500 + (1967*a2*d5*cos(2*t2 + t3 + t4))/1000 - (cos(t2 + t3 + t4)*sin(t2 + t3 + t4)*sin(t5)^2)/2500) - td2*((49450651*sin(t2 + t3 + t4 - t5))/250000000000 - (7474967197*sin(t2 + t3 + t4 - 2*t5))/40000000000000 + (7474967197*sin(t2 + t3 + t4 + 2*t5))/40000000000000 - (713241*sin(t2 + t3 + t4 + t5 + t6))/400000000000 + (49450651*sin(t2 + t3 + t4))/125000000000 - (713241*sin(t2 + t3 + t4 + t5 - t6))/400000000000 - (713241*sin(t2 + t3 + t4 - t5 + t6))/400000000000 + (784477*sin(t2 + t3 + t4 + t5 - 2*t6))/320000000000 - (784477*sin(t2 + t3 + t4 + t5 + 2*t6))/320000000000 - (713241*sin(t2 + t3 + t4 - 2*t5 + t6))/400000000000 - (713241*sin(t2 + t3 + t4 + 2*t5 + t6))/400000000000 + (49450651*sin(t2 + t3 + t4 + t5))/250000000000 + (2041*cos(t2 + t3))/12500 - (713241*sin(t2 + t3 + t4 - t5 - t6))/400000000000 - (784477*sin(t2 + t3 + t4 - t5 - 2*t6))/320000000000 + (784477*sin(t2 + t3 + t4 - t5 + 2*t6))/320000000000 + (713241*sin(t2 + t3 + t4 - 2*t5 - t6))/400000000000 + (713241*sin(t2 + t3 + t4 + 2*t5 - t6))/400000000000 + (784477*sin(t2 + t3 + t4 - 2*t5 - 2*t6))/640000000000 + (784477*sin(t2 + t3 + t4 - 2*t5 + 2*t6))/640000000000 - (784477*sin(t2 + t3 + t4 + 2*t5 - 2*t6))/640000000000 - (784477*sin(t2 + t3 + t4 + 2*t5 + 2*t6))/640000000000 + (1237*cos(t2))/1250 + (817*a3*cos(t2 + t3 - t5 - t6))/8000000 - (43*d6^2*sin(t2 + t3 + t4 - 2*t5))/400 + (43*d6^2*sin(t2 + t3 + t4 + 2*t5))/400 - (817*d4*sin(t2 + t3 + t4 + t5 - t6))/8000000 + (817*d4*sin(t2 + t3 + t4 - t5 + t6))/8000000 + (817*d5*sin(t2 + t3 + t4 + t5 - t6))/8000000 + (817*d5*sin(t2 + t3 + t4 - t5 + t6))/8000000 + (817*d6*sin(t2 + t3 + t4 + t5 - t6))/8000000 + (817*d6*sin(t2 + t3 + t4 - t5 + t6))/8000000 + (817*d6*sin(t2 + t3 + t4 - 2*t5 + t6))/8000000 + (817*d6*sin(t2 + t3 + t4 + 2*t5 + t6))/8000000 + (582539*a3*cos(t2 + t3 - t5))/100000000 - (817*a2*cos(t2 + t5 - t6))/8000000 - (817*a2*cos(t2 - t5 + t6))/8000000 + (817*a2*cos(t5 - t2 + t6))/8000000 + (817*a3*cos(t2 + t3 + t5 + t6))/8000000 + (582539*d4*sin(t2 + t3 + t4 + t5))/100000000 + (817*d4*sin(t2 + t3 + t4 + t6))/4000000 - (582539*d5*sin(t2 + t3 + t4 + t5))/100000000 - (37373*a3*cos(t2 + t3))/2500000 + (582539*a2*cos(t2 + t5))/100000000 + (1532627*a2*cos(t2))/2500000 - (817*d4*sin(t2 + t3 + t4 - t5 - t6))/8000000 - (817*d5*sin(t2 + t3 + t4 - t5 - t6))/8000000 + (817*d6*sin(t2 + t3 + t4 - t5 - t6))/8000000 - (817*d6*sin(t2 + t3 + t4 - 2*t5 - t6))/8000000 - (817*d6*sin(t2 + t3 + t4 + 2*t5 - t6))/8000000 - (817*a3*cos(t2 + t3 + t5 - t6))/8000000 - (817*a3*cos(t2 + t3 - t5 + t6))/8000000 - (582539*d4*sin(t2 + t3 + t4 - t5))/100000000 + (817*d4*sin(t2 + t3 + t4 - t6))/4000000 - (582539*d5*sin(t2 + t3 + t4 - t5))/100000000 + (37539*d6*sin(t2 + t3 + t4 - 2*t5))/10000000 - (37539*d6*sin(t2 + t3 + t4 + 2*t5))/10000000 + (582539*a2*cos(t2 - t5))/100000000 + (817*d4*sin(t2 + t3 + t4 + t5 + t6))/8000000 - (817*d5*sin(t2 + t3 + t4 + t5 + t6))/8000000 + (817*d6*sin(t2 + t3 + t4 + t5 + t6))/8000000 + (582539*a3*cos(t2 + t3 + t5))/100000000 + (817*a2*cos(t2 + t5 + t6))/8000000 - (210469*d4*sin(t2 + t3 + t4))/50000000 - (43*d4*d6*sin(t2 + t3 + t4 - t5))/200 - (43*d5*d6*sin(t2 + t3 + t4 - t5))/200 + (43*a2*d6*cos(t2 - t5))/200 + (43*a3*d6*cos(t2 + t3 + t5))/200 - (2397*d4*d5*sin(t2 + t3 + t4))/1000 + (43*a3*d6*cos(t2 + t3 - t5))/200 + (43*d4*d6*sin(t2 + t3 + t4 + t5))/200 - (43*d5*d6*sin(t2 + t3 + t4 + t5))/200 + (1091*a3*d4*cos(t2 + t3))/250 + (43*a2*d6*cos(t2 + t5))/200 + (1091*a2*d4*cos(t2))/250) - td6*((713241*sin(t2 + t3 + t4 + t5 - t6))/800000000000 - (713241*sin(t2 + t3 + t4 + t5 + t6))/800000000000 - (713241*sin(t2 + t3 + t4 - t5 + t6))/800000000000 - (784477*sin(t2 + t3 + t4 + t5 - 2*t6))/320000000000 - (784477*sin(t2 + t3 + t4 + t5 + 2*t6))/320000000000 - (713241*sin(t2 + t3 + t4 - 2*t5 + t6))/800000000000 - (713241*sin(t2 + t3 + t4 + 2*t5 + t6))/800000000000 + (713241*sin(t2 + t3 + t4 - t5 - t6))/800000000000 + (784477*sin(t2 + t3 + t4 - t5 - 2*t6))/320000000000 + (784477*sin(t2 + t3 + t4 - t5 + 2*t6))/320000000000 - (713241*sin(t2 + t3 + t4 - 2*t5 - t6))/800000000000 - (713241*sin(t2 + t3 + t4 + 2*t5 - t6))/800000000000 - (784477*sin(t2 + t3 + t4 - 2*t5 - 2*t6))/640000000000 + (784477*sin(t2 + t3 + t4 - 2*t5 + 2*t6))/640000000000 + (784477*sin(t2 + t3 + t4 + 2*t5 - 2*t6))/640000000000 - (784477*sin(t2 + t3 + t4 + 2*t5 + 2*t6))/640000000000 - (817*a3*cos(t2 + t3 - t5 - t6))/16000000 + (817*d4*sin(t2 + t3 + t4 + t5 - t6))/16000000 + (817*d4*sin(t2 + t3 + t4 - t5 + t6))/16000000 - (817*d5*sin(t2 + t3 + t4 + t5 - t6))/16000000 + (817*d5*sin(t2 + t3 + t4 - t5 + t6))/16000000 - (817*d6*sin(t2 + t3 + t4 + t5 - t6))/16000000 + (817*d6*sin(t2 + t3 + t4 - t5 + t6))/16000000 + (817*d6*sin(t2 + t3 + t4 - 2*t5 + t6))/16000000 + (817*d6*sin(t2 + t3 + t4 + 2*t5 + t6))/16000000 + (817*a2*cos(t2 + t5 - t6))/16000000 - (817*a2*cos(t2 - t5 + t6))/16000000 - (817*a2*cos(t5 - t2 + t6))/16000000 + (817*a3*cos(t2 + t3 + t5 + t6))/16000000 + (817*d4*sin(t2 + t3 + t4 + t6))/8000000 + (817*d4*sin(t2 + t3 + t4 - t5 - t6))/16000000 + (817*d5*sin(t2 + t3 + t4 - t5 - t6))/16000000 - (817*d6*sin(t2 + t3 + t4 - t5 - t6))/16000000 + (817*d6*sin(t2 + t3 + t4 - 2*t5 - t6))/16000000 + (817*d6*sin(t2 + t3 + t4 + 2*t5 - t6))/16000000 + (817*a3*cos(t2 + t3 + t5 - t6))/16000000 - (817*a3*cos(t2 + t3 - t5 + t6))/16000000 - (817*d4*sin(t2 + t3 + t4 - t6))/8000000 + (817*d4*sin(t2 + t3 + t4 + t5 + t6))/16000000 - (817*d5*sin(t2 + t3 + t4 + t5 + t6))/16000000 + (817*d6*sin(t2 + t3 + t4 + t5 + t6))/16000000 + (817*a2*cos(t2 + t5 + t6))/16000000 + (817*a2*cos(t6)*sin(t2)*sin(t5))/4000000 - (16015523*cos(t2)*cos(t3)*cos(t4)*sin(t5))/80000000000 - (713241*cos(t2)*cos(t3)*cos(t6)*sin(t4))/200000000000 - (713241*cos(t2)*cos(t4)*cos(t6)*sin(t3))/200000000000 - (713241*cos(t3)*cos(t4)*cos(t6)*sin(t2))/200000000000 + (16015523*cos(t2)*sin(t3)*sin(t4)*sin(t5))/80000000000 + (16015523*cos(t3)*sin(t2)*sin(t4)*sin(t5))/80000000000 + (16015523*cos(t4)*sin(t2)*sin(t3)*sin(t5))/80000000000 + (713241*cos(t6)*sin(t2)*sin(t3)*sin(t4))/200000000000 + (817*d4*cos(t2)*cos(t3)*cos(t4)*sin(t6))/4000000 + (817*d6*cos(t2)*cos(t3)*cos(t6)*sin(t4))/4000000 + (817*d6*cos(t2)*cos(t4)*cos(t6)*sin(t3))/4000000 + (817*d6*cos(t3)*cos(t4)*cos(t6)*sin(t2))/4000000 + (817*a3*cos(t2)*cos(t6)*sin(t3)*sin(t5))/4000000 + (817*a3*cos(t3)*cos(t6)*sin(t2)*sin(t5))/4000000 - (817*d4*cos(t2)*sin(t3)*sin(t4)*sin(t6))/4000000 - (817*d4*cos(t3)*sin(t2)*sin(t4)*sin(t6))/4000000 - (817*d4*cos(t4)*sin(t2)*sin(t3)*sin(t6))/4000000 - (817*d6*cos(t6)*sin(t2)*sin(t3)*sin(t4))/4000000 - (713241*cos(t2)*cos(t3)*cos(t4)*cos(t5)*sin(t6))/200000000000 + (713241*cos(t2)*cos(t5)*sin(t3)*sin(t4)*sin(t6))/200000000000 + (713241*cos(t3)*cos(t5)*sin(t2)*sin(t4)*sin(t6))/200000000000 + (713241*cos(t4)*cos(t5)*sin(t2)*sin(t3)*sin(t6))/200000000000 + (817*d4*cos(t2)*cos(t3)*cos(t5)*cos(t6)*sin(t4))/4000000 + (817*d4*cos(t2)*cos(t4)*cos(t5)*cos(t6)*sin(t3))/4000000 + (817*d4*cos(t3)*cos(t4)*cos(t5)*cos(t6)*sin(t2))/4000000 + (817*d5*cos(t2)*cos(t3)*cos(t4)*cos(t6)*sin(t5))/4000000 + (817*d6*cos(t2)*cos(t3)*cos(t4)*cos(t5)*sin(t6))/4000000 - (817*d4*cos(t5)*cos(t6)*sin(t2)*sin(t3)*sin(t4))/4000000 - (817*d5*cos(t2)*cos(t6)*sin(t3)*sin(t4)*sin(t5))/4000000 - (817*d5*cos(t3)*cos(t6)*sin(t2)*sin(t4)*sin(t5))/4000000 - (817*d5*cos(t4)*cos(t6)*sin(t2)*sin(t3)*sin(t5))/4000000 - (817*d6*cos(t2)*cos(t5)*sin(t3)*sin(t4)*sin(t6))/4000000 - (817*d6*cos(t3)*cos(t5)*sin(t2)*sin(t4)*sin(t6))/4000000 - (817*d6*cos(t4)*cos(t5)*sin(t2)*sin(t3)*sin(t6))/4000000) - td3*((49450651*sin(t2 + t3 + t4 - t5))/250000000000 - (7474967197*sin(t2 + t3 + t4 - 2*t5))/40000000000000 + (7474967197*sin(t2 + t3 + t4 + 2*t5))/40000000000000 - (713241*sin(t2 + t3 + t4 + t5 + t6))/400000000000 + (49450651*sin(t2 + t3 + t4))/125000000000 - (713241*sin(t2 + t3 + t4 + t5 - t6))/400000000000 - (713241*sin(t2 + t3 + t4 - t5 + t6))/400000000000 + (784477*sin(t2 + t3 + t4 + t5 - 2*t6))/320000000000 - (784477*sin(t2 + t3 + t4 + t5 + 2*t6))/320000000000 - (713241*sin(t2 + t3 + t4 - 2*t5 + t6))/400000000000 - (713241*sin(t2 + t3 + t4 + 2*t5 + t6))/400000000000 + (49450651*sin(t2 + t3 + t4 + t5))/250000000000 + (2041*cos(t2 + t3))/12500 - (713241*sin(t2 + t3 + t4 - t5 - t6))/400000000000 - (784477*sin(t2 + t3 + t4 - t5 - 2*t6))/320000000000 + (784477*sin(t2 + t3 + t4 - t5 + 2*t6))/320000000000 + (713241*sin(t2 + t3 + t4 - 2*t5 - t6))/400000000000 + (713241*sin(t2 + t3 + t4 + 2*t5 - t6))/400000000000 + (784477*sin(t2 + t3 + t4 - 2*t5 - 2*t6))/640000000000 + (784477*sin(t2 + t3 + t4 - 2*t5 + 2*t6))/640000000000 - (784477*sin(t2 + t3 + t4 + 2*t5 - 2*t6))/640000000000 - (784477*sin(t2 + t3 + t4 + 2*t5 + 2*t6))/640000000000 + (817*a3*cos(t2 + t3 - t5 - t6))/8000000 - (43*d6^2*sin(t2 + t3 + t4 - 2*t5))/400 + (43*d6^2*sin(t2 + t3 + t4 + 2*t5))/400 - (817*d4*sin(t2 + t3 + t4 + t5 - t6))/8000000 + (817*d4*sin(t2 + t3 + t4 - t5 + t6))/8000000 + (817*d5*sin(t2 + t3 + t4 + t5 - t6))/8000000 + (817*d5*sin(t2 + t3 + t4 - t5 + t6))/8000000 + (817*d6*sin(t2 + t3 + t4 + t5 - t6))/8000000 + (817*d6*sin(t2 + t3 + t4 - t5 + t6))/8000000 + (817*d6*sin(t2 + t3 + t4 - 2*t5 + t6))/8000000 + (817*d6*sin(t2 + t3 + t4 + 2*t5 + t6))/8000000 + (582539*a3*cos(t2 + t3 - t5))/100000000 + (817*a3*cos(t2 + t3 + t5 + t6))/8000000 + (582539*d4*sin(t2 + t3 + t4 + t5))/100000000 + (817*d4*sin(t2 + t3 + t4 + t6))/4000000 - (582539*d5*sin(t2 + t3 + t4 + t5))/100000000 - (37373*a3*cos(t2 + t3))/2500000 - (817*d4*sin(t2 + t3 + t4 - t5 - t6))/8000000 - (817*d5*sin(t2 + t3 + t4 - t5 - t6))/8000000 + (817*d6*sin(t2 + t3 + t4 - t5 - t6))/8000000 - (817*d6*sin(t2 + t3 + t4 - 2*t5 - t6))/8000000 - (817*d6*sin(t2 + t3 + t4 + 2*t5 - t6))/8000000 - (817*a3*cos(t2 + t3 + t5 - t6))/8000000 - (817*a3*cos(t2 + t3 - t5 + t6))/8000000 - (582539*d4*sin(t2 + t3 + t4 - t5))/100000000 + (817*d4*sin(t2 + t3 + t4 - t6))/4000000 - (582539*d5*sin(t2 + t3 + t4 - t5))/100000000 + (37539*d6*sin(t2 + t3 + t4 - 2*t5))/10000000 - (37539*d6*sin(t2 + t3 + t4 + 2*t5))/10000000 + (817*d4*sin(t2 + t3 + t4 + t5 + t6))/8000000 - (817*d5*sin(t2 + t3 + t4 + t5 + t6))/8000000 + (817*d6*sin(t2 + t3 + t4 + t5 + t6))/8000000 + (582539*a3*cos(t2 + t3 + t5))/100000000 - (210469*d4*sin(t2 + t3 + t4))/50000000 - (43*d4*d6*sin(t2 + t3 + t4 - t5))/200 - (43*d5*d6*sin(t2 + t3 + t4 - t5))/200 + (43*a3*d6*cos(t2 + t3 + t5))/200 - (2397*d4*d5*sin(t2 + t3 + t4))/1000 + (43*a3*d6*cos(t2 + t3 - t5))/200 + (43*d4*d6*sin(t2 + t3 + t4 + t5))/200 - (43*d5*d6*sin(t2 + t3 + t4 + t5))/200 + (1091*a3*d4*cos(t2 + t3))/250) - td5*((7474967197*sin(t2 + t3 + t4 - 2*t5))/40000000000000 + (7474967197*sin(t2 + t3 + t4 + 2*t5))/40000000000000 + (784477*sin(t2 + t3 + t4 - 2*t6))/320000000000 + (784477*sin(t2 + t3 + t4 + 2*t6))/320000000000 + (33478847947*sin(t2 + t3 + t4))/20000000000000 + (713241*sin(t2 + t3 + t4 - 2*t5 + t6))/400000000000 - (713241*sin(t2 + t3 + t4 + 2*t5 + t6))/400000000000 - (713241*sin(t2 + t3 + t4 - 2*t5 - t6))/400000000000 + (713241*sin(t2 + t3 + t4 + 2*t5 - t6))/400000000000 - (784477*sin(t2 + t3 + t4 - 2*t5 - 2*t6))/640000000000 - (784477*sin(t2 + t3 + t4 - 2*t5 + 2*t6))/640000000000 - (784477*sin(t2 + t3 + t4 + 2*t5 - 2*t6))/640000000000 - (784477*sin(t2 + t3 + t4 + 2*t5 + 2*t6))/640000000000 + (43*d6^2*sin(t2 + t3 + t4 - 2*t5))/400 + (43*d6^2*sin(t2 + t3 + t4 + 2*t5))/400 - (817*d4*sin(t2 + t3 + t4 + t5 - t6))/8000000 - (817*d4*sin(t2 + t3 + t4 - t5 + t6))/8000000 - (817*d6*sin(t2 + t3 + t4 - 2*t5 + t6))/8000000 + (817*d6*sin(t2 + t3 + t4 + 2*t5 + t6))/8000000 + (43*d6^2*sin(t2 + t3 + t4))/200 + (582539*d4*sin(t2 + t3 + t4 + t5))/100000000 + (817*d4*sin(t2 + t3 + t4 - t5 - t6))/8000000 + (817*d6*sin(t2 + t3 + t4 - 2*t5 - t6))/8000000 - (817*d6*sin(t2 + t3 + t4 + 2*t5 - t6))/8000000 + (582539*d4*sin(t2 + t3 + t4 - t5))/100000000 - (37539*d6*sin(t2 + t3 + t4 - 2*t5))/10000000 - (37539*d6*sin(t2 + t3 + t4 + 2*t5))/10000000 + (817*d4*sin(t2 + t3 + t4 + t5 + t6))/8000000 - (37539*d6*sin(t2 + t3 + t4))/5000000 + (43*d4*d6*sin(t2 + t3 + t4 - t5))/200 + (43*d4*d6*sin(t2 + t3 + t4 + t5))/200);

c13=td4*((7474967197*sin(t2 + t3 + t4 - 2*t5))/40000000000000 - (49450651*sin(t2 + t3 + t4 - t5))/250000000000 - (7474967197*sin(t2 + t3 + t4 + 2*t5))/40000000000000 + (713241*sin(t2 + t3 + t4 + t5 + t6))/400000000000 - (49450651*sin(t2 + t3 + t4))/125000000000 + (713241*sin(t2 + t3 + t4 + t5 - t6))/400000000000 + (713241*sin(t2 + t3 + t4 - t5 + t6))/400000000000 - (784477*sin(t2 + t3 + t4 + t5 - 2*t6))/320000000000 + (784477*sin(t2 + t3 + t4 + t5 + 2*t6))/320000000000 + (713241*sin(t2 + t3 + t4 - 2*t5 + t6))/400000000000 + (713241*sin(t2 + t3 + t4 + 2*t5 + t6))/400000000000 - (49450651*sin(t2 + t3 + t4 + t5))/250000000000 + (713241*sin(t2 + t3 + t4 - t5 - t6))/400000000000 + (784477*sin(t2 + t3 + t4 - t5 - 2*t6))/320000000000 - (784477*sin(t2 + t3 + t4 - t5 + 2*t6))/320000000000 - (713241*sin(t2 + t3 + t4 - 2*t5 - t6))/400000000000 - (713241*sin(t2 + t3 + t4 + 2*t5 - t6))/400000000000 - (784477*sin(t2 + t3 + t4 - 2*t5 - 2*t6))/640000000000 - (784477*sin(t2 + t3 + t4 - 2*t5 + 2*t6))/640000000000 + (784477*sin(t2 + t3 + t4 + 2*t5 - 2*t6))/640000000000 + (784477*sin(t2 + t3 + t4 + 2*t5 + 2*t6))/640000000000 + (43*d6^2*sin(t2 + t3 + t4 - 2*t5))/400 - (43*d6^2*sin(t2 + t3 + t4 + 2*t5))/400 + (817*d4*sin(t2 + t3 + t4 + t5 - t6))/8000000 - (817*d4*sin(t2 + t3 + t4 - t5 + t6))/8000000 - (817*d5*sin(t2 + t3 + t4 + t5 - t6))/8000000 - (817*d5*sin(t2 + t3 + t4 - t5 + t6))/8000000 - (817*d6*sin(t2 + t3 + t4 + t5 - t6))/8000000 - (817*d6*sin(t2 + t3 + t4 - t5 + t6))/8000000 - (817*d6*sin(t2 + t3 + t4 - 2*t5 + t6))/8000000 - (817*d6*sin(t2 + t3 + t4 + 2*t5 + t6))/8000000 - (582539*d4*sin(t2 + t3 + t4 + t5))/100000000 - (817*d4*sin(t2 + t3 + t4 + t6))/4000000 + (582539*d5*sin(t2 + t3 + t4 + t5))/100000000 + (817*d4*sin(t2 + t3 + t4 - t5 - t6))/8000000 + (817*d5*sin(t2 + t3 + t4 - t5 - t6))/8000000 - (817*d6*sin(t2 + t3 + t4 - t5 - t6))/8000000 + (817*d6*sin(t2 + t3 + t4 - 2*t5 - t6))/8000000 + (817*d6*sin(t2 + t3 + t4 + 2*t5 - t6))/8000000 + (582539*d4*sin(t2 + t3 + t4 - t5))/100000000 - (817*d4*sin(t2 + t3 + t4 - t6))/4000000 + (582539*d5*sin(t2 + t3 + t4 - t5))/100000000 - (37539*d6*sin(t2 + t3 + t4 - 2*t5))/10000000 + (37539*d6*sin(t2 + t3 + t4 + 2*t5))/10000000 - (817*d4*sin(t2 + t3 + t4 + t5 + t6))/8000000 + (817*d5*sin(t2 + t3 + t4 + t5 + t6))/8000000 - (817*d6*sin(t2 + t3 + t4 + t5 + t6))/8000000 + (210469*d4*sin(t2 + t3 + t4))/50000000 + (43*d4*d6*sin(t2 + t3 + t4 - t5))/200 + (43*d5*d6*sin(t2 + t3 + t4 - t5))/200 + (2397*d4*d5*sin(t2 + t3 + t4))/1000 - (43*d4*d6*sin(t2 + t3 + t4 + t5))/200 + (43*d5*d6*sin(t2 + t3 + t4 + t5))/200) - td3*((49450651*sin(t2 + t3 + t4 - t5))/250000000000 - (7474967197*sin(t2 + t3 + t4 - 2*t5))/40000000000000 + (7474967197*sin(t2 + t3 + t4 + 2*t5))/40000000000000 - (713241*sin(t2 + t3 + t4 + t5 + t6))/400000000000 + (49450651*sin(t2 + t3 + t4))/125000000000 - (713241*sin(t2 + t3 + t4 + t5 - t6))/400000000000 - (713241*sin(t2 + t3 + t4 - t5 + t6))/400000000000 + (784477*sin(t2 + t3 + t4 + t5 - 2*t6))/320000000000 - (784477*sin(t2 + t3 + t4 + t5 + 2*t6))/320000000000 - (713241*sin(t2 + t3 + t4 - 2*t5 + t6))/400000000000 - (713241*sin(t2 + t3 + t4 + 2*t5 + t6))/400000000000 + (49450651*sin(t2 + t3 + t4 + t5))/250000000000 + (2041*cos(t2 + t3))/12500 - (713241*sin(t2 + t3 + t4 - t5 - t6))/400000000000 - (784477*sin(t2 + t3 + t4 - t5 - 2*t6))/320000000000 + (784477*sin(t2 + t3 + t4 - t5 + 2*t6))/320000000000 + (713241*sin(t2 + t3 + t4 - 2*t5 - t6))/400000000000 + (713241*sin(t2 + t3 + t4 + 2*t5 - t6))/400000000000 + (784477*sin(t2 + t3 + t4 - 2*t5 - 2*t6))/640000000000 + (784477*sin(t2 + t3 + t4 - 2*t5 + 2*t6))/640000000000 - (784477*sin(t2 + t3 + t4 + 2*t5 - 2*t6))/640000000000 - (784477*sin(t2 + t3 + t4 + 2*t5 + 2*t6))/640000000000 + (817*a3*cos(t2 + t3 - t5 - t6))/8000000 - (43*d6^2*sin(t2 + t3 + t4 - 2*t5))/400 + (43*d6^2*sin(t2 + t3 + t4 + 2*t5))/400 - (817*d4*sin(t2 + t3 + t4 + t5 - t6))/8000000 + (817*d4*sin(t2 + t3 + t4 - t5 + t6))/8000000 + (817*d5*sin(t2 + t3 + t4 + t5 - t6))/8000000 + (817*d5*sin(t2 + t3 + t4 - t5 + t6))/8000000 + (817*d6*sin(t2 + t3 + t4 + t5 - t6))/8000000 + (817*d6*sin(t2 + t3 + t4 - t5 + t6))/8000000 + (817*d6*sin(t2 + t3 + t4 - 2*t5 + t6))/8000000 + (817*d6*sin(t2 + t3 + t4 + 2*t5 + t6))/8000000 + (582539*a3*cos(t2 + t3 - t5))/100000000 + (817*a3*cos(t2 + t3 + t5 + t6))/8000000 + (582539*d4*sin(t2 + t3 + t4 + t5))/100000000 + (817*d4*sin(t2 + t3 + t4 + t6))/4000000 - (582539*d5*sin(t2 + t3 + t4 + t5))/100000000 - (37373*a3*cos(t2 + t3))/2500000 - (817*d4*sin(t2 + t3 + t4 - t5 - t6))/8000000 - (817*d5*sin(t2 + t3 + t4 - t5 - t6))/8000000 + (817*d6*sin(t2 + t3 + t4 - t5 - t6))/8000000 - (817*d6*sin(t2 + t3 + t4 - 2*t5 - t6))/8000000 - (817*d6*sin(t2 + t3 + t4 + 2*t5 - t6))/8000000 - (817*a3*cos(t2 + t3 + t5 - t6))/8000000 - (817*a3*cos(t2 + t3 - t5 + t6))/8000000 - (582539*d4*sin(t2 + t3 + t4 - t5))/100000000 + (817*d4*sin(t2 + t3 + t4 - t6))/4000000 - (582539*d5*sin(t2 + t3 + t4 - t5))/100000000 + (37539*d6*sin(t2 + t3 + t4 - 2*t5))/10000000 - (37539*d6*sin(t2 + t3 + t4 + 2*t5))/10000000 + (817*d4*sin(t2 + t3 + t4 + t5 + t6))/8000000 - (817*d5*sin(t2 + t3 + t4 + t5 + t6))/8000000 + (817*d6*sin(t2 + t3 + t4 + t5 + t6))/8000000 + (582539*a3*cos(t2 + t3 + t5))/100000000 - (210469*d4*sin(t2 + t3 + t4))/50000000 - (43*d4*d6*sin(t2 + t3 + t4 - t5))/200 - (43*d5*d6*sin(t2 + t3 + t4 - t5))/200 + (43*a3*d6*cos(t2 + t3 + t5))/200 - (2397*d4*d5*sin(t2 + t3 + t4))/1000 + (43*a3*d6*cos(t2 + t3 - t5))/200 + (43*d4*d6*sin(t2 + t3 + t4 + t5))/200 - (43*d5*d6*sin(t2 + t3 + t4 + t5))/200 + (1091*a3*d4*cos(t2 + t3))/250) - td1*((49450651*sin(2*t2 + 2*t3 + 2*t4 - t5))/250000000000 - (1966511423*sin(2*t2 + 2*t3 + 2*t4 - 2*t5))/20000000000000 - (1966511423*sin(2*t2 + 2*t3 + 2*t4 + 2*t5))/20000000000000 - (3534581023*sin(2*t2 + 2*t3 + 2*t4))/10000000000000 + (42783*sin(2*t2 + 2*t3))/62500 - (49450651*sin(2*t2 + 2*t3 + 2*t4 + t5))/250000000000 + (37373*d5*sin(2*t2 + 2*t3 + 2*t4))/2500000 + (957929*a2*cos(2*t2 + t3 + t4 - t5))/200000000 - (957929*a3*cos(2*t2 + 2*t3 + t4 + t5))/100000000 + (210469*a2*cos(2*t2 + t3 + t4))/100000000 + (957929*a2*cos(t3 + t4 - t5))/200000000 + (((43*a3*sin(t2 + t3)*sin(t1))/100 - (37539*sin(t2 + t3 + t4)*sin(t1)*sin(t5))/5000000 - (817*cos(t2 + t3 + t4)*cos(t6)*sin(t1))/2000000 + (43*d5*cos(t2 + t3 + t4)*sin(t1))/100 + (817*sin(t2 + t3 + t4)*cos(t5)*sin(t1)*sin(t6))/2000000 + (43*d6*sin(t2 + t3 + t4)*sin(t1)*sin(t5))/100)*((19*sin(t6)*(cos(t1)*sin(t5) + cos(t2 + t3 + t4)*cos(t5)*sin(t1)))/20000 + (873*cos(t1)*cos(t5))/50000 - d6*(cos(t1)*cos(t5) - cos(t2 + t3 + t4)*sin(t1)*sin(t5)) - d4*cos(t1) - (873*cos(t2 + t3 + t4)*sin(t1)*sin(t5))/50000 + (19*sin(t2 + t3 + t4)*cos(t6)*sin(t1))/20000 + a3*cos(t2 + t3)*sin(t1) + a2*cos(t2)*sin(t1) - d5*sin(t2 + t3 + t4)*sin(t1)))/2 + ((a3*sin(t2 + t3)*sin(t1) - (873*sin(t2 + t3 + t4)*sin(t1)*sin(t5))/50000 - (19*cos(t2 + t3 + t4)*cos(t6)*sin(t1))/20000 + d5*cos(t2 + t3 + t4)*sin(t1) + (19*sin(t2 + t3 + t4)*cos(t5)*sin(t1)*sin(t6))/20000 + d6*sin(t2 + t3 + t4)*sin(t1)*sin(t5))*((817*sin(t6)*(cos(t1)*sin(t5) + cos(t2 + t3 + t4)*cos(t5)*sin(t1)))/2000000 + (37539*cos(t1)*cos(t5))/5000000 - (43*d6*(cos(t1)*cos(t5) - cos(t2 + t3 + t4)*sin(t1)*sin(t5)))/100 - (43*d4*cos(t1))/100 - (37539*cos(t2 + t3 + t4)*sin(t1)*sin(t5))/5000000 + (817*sin(t2 + t3 + t4)*cos(t6)*sin(t1))/2000000 + (43*a3*cos(t2 + t3)*sin(t1))/100 + (43*a2*cos(t2)*sin(t1))/100 - (43*d5*sin(t2 + t3 + t4)*sin(t1))/100))/2 + ((sin(t2 + t3 + t4)*cos(t6) + cos(t2 + t3 + t4)*cos(t5)*sin(t6))*((3*cos(t2 + t3 + t4)*cos(t6))/12500 - (3*sin(t2 + t3 + t4)*cos(t5)*sin(t6))/12500))/2 + ((cos(t2 + t3 + t4)*cos(t6) - sin(t2 + t3 + t4)*cos(t5)*sin(t6))*((3*sin(t2 + t3 + t4)*cos(t6))/12500 + (3*cos(t2 + t3 + t4)*cos(t5)*sin(t6))/12500))/2 + ((cos(t2 + t3 + t4)*sin(t6) + sin(t2 + t3 + t4)*cos(t5)*cos(t6))*((11*sin(t2 + t3 + t4)*sin(t6))/50000 - (11*cos(t2 + t3 + t4)*cos(t5)*cos(t6))/50000))/2 + ((sin(t2 + t3 + t4)*sin(t6) - cos(t2 + t3 + t4)*cos(t5)*cos(t6))*((11*cos(t2 + t3 + t4)*sin(t6))/50000 + (11*sin(t2 + t3 + t4)*cos(t5)*cos(t6))/50000))/2 + (210469*a2*cos(t3 + t4))/100000000 - (1967*d5^2*sin(2*t2 + 2*t3 + 2*t4))/2000 + (957929*a3*cos(2*t2 + 2*t3 + t4 - t5))/100000000 + (957929*d5*sin(2*t2 + 2*t3 + 2*t4 + t5))/100000000 + (1967*a3^2*sin(2*t2 + 2*t3))/1000 + (210469*a3*cos(2*t2 + 2*t3 + t4))/50000000 + (2041*a2*sin(t3))/1250 - (957929*a2*cos(2*t2 + t3 + t4 + t5))/200000000 + (((43*a3*sin(t2 + t3)*cos(t1))/100 - (37539*sin(t2 + t3 + t4)*cos(t1)*sin(t5))/5000000 - (817*cos(t2 + t3 + t4)*cos(t1)*cos(t6))/2000000 + (43*d5*cos(t2 + t3 + t4)*cos(t1))/100 + (817*sin(t2 + t3 + t4)*cos(t1)*cos(t5)*sin(t6))/2000000 + (43*d6*sin(t2 + t3 + t4)*cos(t1)*sin(t5))/100)*(d6*(cos(t5)*sin(t1) + cos(t2 + t3 + t4)*cos(t1)*sin(t5)) - (873*cos(t5)*sin(t1))/50000 - (19*sin(t6)*(sin(t1)*sin(t5) - cos(t2 + t3 + t4)*cos(t1)*cos(t5)))/20000 + d4*sin(t1) - (873*cos(t2 + t3 + t4)*cos(t1)*sin(t5))/50000 + (19*sin(t2 + t3 + t4)*cos(t1)*cos(t6))/20000 + a3*cos(t2 + t3)*cos(t1) + a2*cos(t1)*cos(t2) - d5*sin(t2 + t3 + t4)*cos(t1)))/2 + ((a3*sin(t2 + t3)*cos(t1) - (873*sin(t2 + t3 + t4)*cos(t1)*sin(t5))/50000 - (19*cos(t2 + t3 + t4)*cos(t1)*cos(t6))/20000 + d5*cos(t2 + t3 + t4)*cos(t1) + (19*sin(t2 + t3 + t4)*cos(t1)*cos(t5)*sin(t6))/20000 + d6*sin(t2 + t3 + t4)*cos(t1)*sin(t5))*((43*d6*(cos(t5)*sin(t1) + cos(t2 + t3 + t4)*cos(t1)*sin(t5)))/100 - (37539*cos(t5)*sin(t1))/5000000 - (817*sin(t6)*(sin(t1)*sin(t5) - cos(t2 + t3 + t4)*cos(t1)*cos(t5)))/2000000 + (43*d4*sin(t1))/100 - (37539*cos(t2 + t3 + t4)*cos(t1)*sin(t5))/5000000 + (817*sin(t2 + t3 + t4)*cos(t1)*cos(t6))/2000000 + (43*a3*cos(t2 + t3)*cos(t1))/100 + (43*a2*cos(t1)*cos(t2))/100 - (43*d5*sin(t2 + t3 + t4)*cos(t1))/100))/2 + (2041*a2*sin(2*t2 + t3))/1250 - (957929*a2*cos(t3 + t4 + t5))/200000000 - (957929*d5*sin(2*t2 + 2*t3 + 2*t4 - t5))/100000000 + (1967*a3*d5*cos(2*t2 + 2*t3 + t4))/1000 + (1967*a2*a3*sin(t3))/1000 + (1967*a2*a3*sin(2*t2 + t3))/1000 + (1967*a2*d5*cos(2*t2 + t3 + t4))/2000 + (1967*a2*d5*cos(t3 + t4))/2000 - (cos(t2 + t3 + t4)*sin(t2 + t3 + t4)*sin(t5)^2)/2500) - td6*((713241*sin(t2 + t3 + t4 + t5 - t6))/800000000000 - (713241*sin(t2 + t3 + t4 + t5 + t6))/800000000000 - (713241*sin(t2 + t3 + t4 - t5 + t6))/800000000000 - (784477*sin(t2 + t3 + t4 + t5 - 2*t6))/320000000000 - (784477*sin(t2 + t3 + t4 + t5 + 2*t6))/320000000000 - (713241*sin(t2 + t3 + t4 - 2*t5 + t6))/800000000000 - (713241*sin(t2 + t3 + t4 + 2*t5 + t6))/800000000000 + (713241*sin(t2 + t3 + t4 - t5 - t6))/800000000000 + (784477*sin(t2 + t3 + t4 - t5 - 2*t6))/320000000000 + (784477*sin(t2 + t3 + t4 - t5 + 2*t6))/320000000000 - (713241*sin(t2 + t3 + t4 - 2*t5 - t6))/800000000000 - (713241*sin(t2 + t3 + t4 + 2*t5 - t6))/800000000000 - (784477*sin(t2 + t3 + t4 - 2*t5 - 2*t6))/640000000000 + (784477*sin(t2 + t3 + t4 - 2*t5 + 2*t6))/640000000000 + (784477*sin(t2 + t3 + t4 + 2*t5 - 2*t6))/640000000000 - (784477*sin(t2 + t3 + t4 + 2*t5 + 2*t6))/640000000000 - (817*a3*cos(t2 + t3 - t5 - t6))/16000000 + (817*d4*sin(t2 + t3 + t4 + t5 - t6))/16000000 + (817*d4*sin(t2 + t3 + t4 - t5 + t6))/16000000 - (817*d5*sin(t2 + t3 + t4 + t5 - t6))/16000000 + (817*d5*sin(t2 + t3 + t4 - t5 + t6))/16000000 - (817*d6*sin(t2 + t3 + t4 + t5 - t6))/16000000 + (817*d6*sin(t2 + t3 + t4 - t5 + t6))/16000000 + (817*d6*sin(t2 + t3 + t4 - 2*t5 + t6))/16000000 + (817*d6*sin(t2 + t3 + t4 + 2*t5 + t6))/16000000 + (817*a3*cos(t2 + t3 + t5 + t6))/16000000 + (817*d4*sin(t2 + t3 + t4 + t6))/8000000 + (817*d4*sin(t2 + t3 + t4 - t5 - t6))/16000000 + (817*d5*sin(t2 + t3 + t4 - t5 - t6))/16000000 - (817*d6*sin(t2 + t3 + t4 - t5 - t6))/16000000 + (817*d6*sin(t2 + t3 + t4 - 2*t5 - t6))/16000000 + (817*d6*sin(t2 + t3 + t4 + 2*t5 - t6))/16000000 + (817*a3*cos(t2 + t3 + t5 - t6))/16000000 - (817*a3*cos(t2 + t3 - t5 + t6))/16000000 - (817*d4*sin(t2 + t3 + t4 - t6))/8000000 + (817*d4*sin(t2 + t3 + t4 + t5 + t6))/16000000 - (817*d5*sin(t2 + t3 + t4 + t5 + t6))/16000000 + (817*d6*sin(t2 + t3 + t4 + t5 + t6))/16000000 - (16015523*cos(t2)*cos(t3)*cos(t4)*sin(t5))/80000000000 - (713241*cos(t2)*cos(t3)*cos(t6)*sin(t4))/200000000000 - (713241*cos(t2)*cos(t4)*cos(t6)*sin(t3))/200000000000 - (713241*cos(t3)*cos(t4)*cos(t6)*sin(t2))/200000000000 + (16015523*cos(t2)*sin(t3)*sin(t4)*sin(t5))/80000000000 + (16015523*cos(t3)*sin(t2)*sin(t4)*sin(t5))/80000000000 + (16015523*cos(t4)*sin(t2)*sin(t3)*sin(t5))/80000000000 + (713241*cos(t6)*sin(t2)*sin(t3)*sin(t4))/200000000000 + (817*d4*cos(t2)*cos(t3)*cos(t4)*sin(t6))/4000000 + (817*d6*cos(t2)*cos(t3)*cos(t6)*sin(t4))/4000000 + (817*d6*cos(t2)*cos(t4)*cos(t6)*sin(t3))/4000000 + (817*d6*cos(t3)*cos(t4)*cos(t6)*sin(t2))/4000000 + (817*a3*cos(t2)*cos(t6)*sin(t3)*sin(t5))/4000000 + (817*a3*cos(t3)*cos(t6)*sin(t2)*sin(t5))/4000000 - (817*d4*cos(t2)*sin(t3)*sin(t4)*sin(t6))/4000000 - (817*d4*cos(t3)*sin(t2)*sin(t4)*sin(t6))/4000000 - (817*d4*cos(t4)*sin(t2)*sin(t3)*sin(t6))/4000000 - (817*d6*cos(t6)*sin(t2)*sin(t3)*sin(t4))/4000000 - (713241*cos(t2)*cos(t3)*cos(t4)*cos(t5)*sin(t6))/200000000000 + (713241*cos(t2)*cos(t5)*sin(t3)*sin(t4)*sin(t6))/200000000000 + (713241*cos(t3)*cos(t5)*sin(t2)*sin(t4)*sin(t6))/200000000000 + (713241*cos(t4)*cos(t5)*sin(t2)*sin(t3)*sin(t6))/200000000000 + (817*d4*cos(t2)*cos(t3)*cos(t5)*cos(t6)*sin(t4))/4000000 + (817*d4*cos(t2)*cos(t4)*cos(t5)*cos(t6)*sin(t3))/4000000 + (817*d4*cos(t3)*cos(t4)*cos(t5)*cos(t6)*sin(t2))/4000000 + (817*d5*cos(t2)*cos(t3)*cos(t4)*cos(t6)*sin(t5))/4000000 + (817*d6*cos(t2)*cos(t3)*cos(t4)*cos(t5)*sin(t6))/4000000 - (817*d4*cos(t5)*cos(t6)*sin(t2)*sin(t3)*sin(t4))/4000000 - (817*d5*cos(t2)*cos(t6)*sin(t3)*sin(t4)*sin(t5))/4000000 - (817*d5*cos(t3)*cos(t6)*sin(t2)*sin(t4)*sin(t5))/4000000 - (817*d5*cos(t4)*cos(t6)*sin(t2)*sin(t3)*sin(t5))/4000000 - (817*d6*cos(t2)*cos(t5)*sin(t3)*sin(t4)*sin(t6))/4000000 - (817*d6*cos(t3)*cos(t5)*sin(t2)*sin(t4)*sin(t6))/4000000 - (817*d6*cos(t4)*cos(t5)*sin(t2)*sin(t3)*sin(t6))/4000000) - td2*((49450651*sin(t2 + t3 + t4 - t5))/250000000000 - (7474967197*sin(t2 + t3 + t4 - 2*t5))/40000000000000 + (7474967197*sin(t2 + t3 + t4 + 2*t5))/40000000000000 - (713241*sin(t2 + t3 + t4 + t5 + t6))/400000000000 + (49450651*sin(t2 + t3 + t4))/125000000000 - (713241*sin(t2 + t3 + t4 + t5 - t6))/400000000000 - (713241*sin(t2 + t3 + t4 - t5 + t6))/400000000000 + (784477*sin(t2 + t3 + t4 + t5 - 2*t6))/320000000000 - (784477*sin(t2 + t3 + t4 + t5 + 2*t6))/320000000000 - (713241*sin(t2 + t3 + t4 - 2*t5 + t6))/400000000000 - (713241*sin(t2 + t3 + t4 + 2*t5 + t6))/400000000000 + (49450651*sin(t2 + t3 + t4 + t5))/250000000000 + (2041*cos(t2 + t3))/12500 - (713241*sin(t2 + t3 + t4 - t5 - t6))/400000000000 - (784477*sin(t2 + t3 + t4 - t5 - 2*t6))/320000000000 + (784477*sin(t2 + t3 + t4 - t5 + 2*t6))/320000000000 + (713241*sin(t2 + t3 + t4 - 2*t5 - t6))/400000000000 + (713241*sin(t2 + t3 + t4 + 2*t5 - t6))/400000000000 + (784477*sin(t2 + t3 + t4 - 2*t5 - 2*t6))/640000000000 + (784477*sin(t2 + t3 + t4 - 2*t5 + 2*t6))/640000000000 - (784477*sin(t2 + t3 + t4 + 2*t5 - 2*t6))/640000000000 - (784477*sin(t2 + t3 + t4 + 2*t5 + 2*t6))/640000000000 + (817*a3*cos(t2 + t3 - t5 - t6))/8000000 - (43*d6^2*sin(t2 + t3 + t4 - 2*t5))/400 + (43*d6^2*sin(t2 + t3 + t4 + 2*t5))/400 - (817*d4*sin(t2 + t3 + t4 + t5 - t6))/8000000 + (817*d4*sin(t2 + t3 + t4 - t5 + t6))/8000000 + (817*d5*sin(t2 + t3 + t4 + t5 - t6))/8000000 + (817*d5*sin(t2 + t3 + t4 - t5 + t6))/8000000 + (817*d6*sin(t2 + t3 + t4 + t5 - t6))/8000000 + (817*d6*sin(t2 + t3 + t4 - t5 + t6))/8000000 + (817*d6*sin(t2 + t3 + t4 - 2*t5 + t6))/8000000 + (817*d6*sin(t2 + t3 + t4 + 2*t5 + t6))/8000000 + (582539*a3*cos(t2 + t3 - t5))/100000000 + (817*a3*cos(t2 + t3 + t5 + t6))/8000000 + (582539*d4*sin(t2 + t3 + t4 + t5))/100000000 + (817*d4*sin(t2 + t3 + t4 + t6))/4000000 - (582539*d5*sin(t2 + t3 + t4 + t5))/100000000 - (37373*a3*cos(t2 + t3))/2500000 - (817*d4*sin(t2 + t3 + t4 - t5 - t6))/8000000 - (817*d5*sin(t2 + t3 + t4 - t5 - t6))/8000000 + (817*d6*sin(t2 + t3 + t4 - t5 - t6))/8000000 - (817*d6*sin(t2 + t3 + t4 - 2*t5 - t6))/8000000 - (817*d6*sin(t2 + t3 + t4 + 2*t5 - t6))/8000000 - (817*a3*cos(t2 + t3 + t5 - t6))/8000000 - (817*a3*cos(t2 + t3 - t5 + t6))/8000000 - (582539*d4*sin(t2 + t3 + t4 - t5))/100000000 + (817*d4*sin(t2 + t3 + t4 - t6))/4000000 - (582539*d5*sin(t2 + t3 + t4 - t5))/100000000 + (37539*d6*sin(t2 + t3 + t4 - 2*t5))/10000000 - (37539*d6*sin(t2 + t3 + t4 + 2*t5))/10000000 + (817*d4*sin(t2 + t3 + t4 + t5 + t6))/8000000 - (817*d5*sin(t2 + t3 + t4 + t5 + t6))/8000000 + (817*d6*sin(t2 + t3 + t4 + t5 + t6))/8000000 + (582539*a3*cos(t2 + t3 + t5))/100000000 - (210469*d4*sin(t2 + t3 + t4))/50000000 - (43*d4*d6*sin(t2 + t3 + t4 - t5))/200 - (43*d5*d6*sin(t2 + t3 + t4 - t5))/200 + (43*a3*d6*cos(t2 + t3 + t5))/200 - (2397*d4*d5*sin(t2 + t3 + t4))/1000 + (43*a3*d6*cos(t2 + t3 - t5))/200 + (43*d4*d6*sin(t2 + t3 + t4 + t5))/200 - (43*d5*d6*sin(t2 + t3 + t4 + t5))/200 + (1091*a3*d4*cos(t2 + t3))/250) - td5*((7474967197*sin(t2 + t3 + t4 - 2*t5))/40000000000000 + (7474967197*sin(t2 + t3 + t4 + 2*t5))/40000000000000 + (784477*sin(t2 + t3 + t4 - 2*t6))/320000000000 + (784477*sin(t2 + t3 + t4 + 2*t6))/320000000000 + (33478847947*sin(t2 + t3 + t4))/20000000000000 + (713241*sin(t2 + t3 + t4 - 2*t5 + t6))/400000000000 - (713241*sin(t2 + t3 + t4 + 2*t5 + t6))/400000000000 - (713241*sin(t2 + t3 + t4 - 2*t5 - t6))/400000000000 + (713241*sin(t2 + t3 + t4 + 2*t5 - t6))/400000000000 - (784477*sin(t2 + t3 + t4 - 2*t5 - 2*t6))/640000000000 - (784477*sin(t2 + t3 + t4 - 2*t5 + 2*t6))/640000000000 - (784477*sin(t2 + t3 + t4 + 2*t5 - 2*t6))/640000000000 - (784477*sin(t2 + t3 + t4 + 2*t5 + 2*t6))/640000000000 + (43*d6^2*sin(t2 + t3 + t4 - 2*t5))/400 + (43*d6^2*sin(t2 + t3 + t4 + 2*t5))/400 - (817*d4*sin(t2 + t3 + t4 + t5 - t6))/8000000 - (817*d4*sin(t2 + t3 + t4 - t5 + t6))/8000000 - (817*d6*sin(t2 + t3 + t4 - 2*t5 + t6))/8000000 + (817*d6*sin(t2 + t3 + t4 + 2*t5 + t6))/8000000 + (43*d6^2*sin(t2 + t3 + t4))/200 + (582539*d4*sin(t2 + t3 + t4 + t5))/100000000 + (817*d4*sin(t2 + t3 + t4 - t5 - t6))/8000000 + (817*d6*sin(t2 + t3 + t4 - 2*t5 - t6))/8000000 - (817*d6*sin(t2 + t3 + t4 + 2*t5 - t6))/8000000 + (582539*d4*sin(t2 + t3 + t4 - t5))/100000000 - (37539*d6*sin(t2 + t3 + t4 - 2*t5))/10000000 - (37539*d6*sin(t2 + t3 + t4 + 2*t5))/10000000 + (817*d4*sin(t2 + t3 + t4 + t5 + t6))/8000000 - (37539*d6*sin(t2 + t3 + t4))/5000000 + (43*d4*d6*sin(t2 + t3 + t4 - t5))/200 + (43*d4*d6*sin(t2 + t3 + t4 + t5))/200);

c14=td2*((7474967197*sin(t2 + t3 + t4 - 2*t5))/40000000000000 - (49450651*sin(t2 + t3 + t4 - t5))/250000000000 - (7474967197*sin(t2 + t3 + t4 + 2*t5))/40000000000000 + (713241*sin(t2 + t3 + t4 + t5 + t6))/400000000000 - (49450651*sin(t2 + t3 + t4))/125000000000 + (713241*sin(t2 + t3 + t4 + t5 - t6))/400000000000 + (713241*sin(t2 + t3 + t4 - t5 + t6))/400000000000 - (784477*sin(t2 + t3 + t4 + t5 - 2*t6))/320000000000 + (784477*sin(t2 + t3 + t4 + t5 + 2*t6))/320000000000 + (713241*sin(t2 + t3 + t4 - 2*t5 + t6))/400000000000 + (713241*sin(t2 + t3 + t4 + 2*t5 + t6))/400000000000 - (49450651*sin(t2 + t3 + t4 + t5))/250000000000 + (713241*sin(t2 + t3 + t4 - t5 - t6))/400000000000 + (784477*sin(t2 + t3 + t4 - t5 - 2*t6))/320000000000 - (784477*sin(t2 + t3 + t4 - t5 + 2*t6))/320000000000 - (713241*sin(t2 + t3 + t4 - 2*t5 - t6))/400000000000 - (713241*sin(t2 + t3 + t4 + 2*t5 - t6))/400000000000 - (784477*sin(t2 + t3 + t4 - 2*t5 - 2*t6))/640000000000 - (784477*sin(t2 + t3 + t4 - 2*t5 + 2*t6))/640000000000 + (784477*sin(t2 + t3 + t4 + 2*t5 - 2*t6))/640000000000 + (784477*sin(t2 + t3 + t4 + 2*t5 + 2*t6))/640000000000 + (43*d6^2*sin(t2 + t3 + t4 - 2*t5))/400 - (43*d6^2*sin(t2 + t3 + t4 + 2*t5))/400 + (817*d4*sin(t2 + t3 + t4 + t5 - t6))/8000000 - (817*d4*sin(t2 + t3 + t4 - t5 + t6))/8000000 - (817*d5*sin(t2 + t3 + t4 + t5 - t6))/8000000 - (817*d5*sin(t2 + t3 + t4 - t5 + t6))/8000000 - (817*d6*sin(t2 + t3 + t4 + t5 - t6))/8000000 - (817*d6*sin(t2 + t3 + t4 - t5 + t6))/8000000 - (817*d6*sin(t2 + t3 + t4 - 2*t5 + t6))/8000000 - (817*d6*sin(t2 + t3 + t4 + 2*t5 + t6))/8000000 - (582539*d4*sin(t2 + t3 + t4 + t5))/100000000 - (817*d4*sin(t2 + t3 + t4 + t6))/4000000 + (582539*d5*sin(t2 + t3 + t4 + t5))/100000000 + (817*d4*sin(t2 + t3 + t4 - t5 - t6))/8000000 + (817*d5*sin(t2 + t3 + t4 - t5 - t6))/8000000 - (817*d6*sin(t2 + t3 + t4 - t5 - t6))/8000000 + (817*d6*sin(t2 + t3 + t4 - 2*t5 - t6))/8000000 + (817*d6*sin(t2 + t3 + t4 + 2*t5 - t6))/8000000 + (582539*d4*sin(t2 + t3 + t4 - t5))/100000000 - (817*d4*sin(t2 + t3 + t4 - t6))/4000000 + (582539*d5*sin(t2 + t3 + t4 - t5))/100000000 - (37539*d6*sin(t2 + t3 + t4 - 2*t5))/10000000 + (37539*d6*sin(t2 + t3 + t4 + 2*t5))/10000000 - (817*d4*sin(t2 + t3 + t4 + t5 + t6))/8000000 + (817*d5*sin(t2 + t3 + t4 + t5 + t6))/8000000 - (817*d6*sin(t2 + t3 + t4 + t5 + t6))/8000000 + (210469*d4*sin(t2 + t3 + t4))/50000000 + (43*d4*d6*sin(t2 + t3 + t4 - t5))/200 + (43*d5*d6*sin(t2 + t3 + t4 - t5))/200 + (2397*d4*d5*sin(t2 + t3 + t4))/1000 - (43*d4*d6*sin(t2 + t3 + t4 + t5))/200 + (43*d5*d6*sin(t2 + t3 + t4 + t5))/200) - td1*((49450651*sin(2*t2 + 2*t3 + 2*t4 - t5))/250000000000 - (1966511423*sin(2*t2 + 2*t3 + 2*t4 - 2*t5))/20000000000000 - (1966511423*sin(2*t2 + 2*t3 + 2*t4 + 2*t5))/20000000000000 - (3534581023*sin(2*t2 + 2*t3 + 2*t4))/10000000000000 - (49450651*sin(2*t2 + 2*t3 + 2*t4 + t5))/250000000000 + (37373*d5*sin(2*t2 + 2*t3 + 2*t4))/2500000 + (957929*a2*cos(2*t2 + t3 + t4 - t5))/200000000 - (957929*a3*cos(2*t2 + 2*t3 + t4 + t5))/200000000 + (210469*a2*cos(2*t2 + t3 + t4))/100000000 + (957929*a2*cos(t3 + t4 - t5))/200000000 + ((sin(t2 + t3 + t4)*cos(t6) + cos(t2 + t3 + t4)*cos(t5)*sin(t6))*((3*cos(t2 + t3 + t4)*cos(t6))/12500 - (3*sin(t2 + t3 + t4)*cos(t5)*sin(t6))/12500))/2 + ((cos(t2 + t3 + t4)*cos(t6) - sin(t2 + t3 + t4)*cos(t5)*sin(t6))*((3*sin(t2 + t3 + t4)*cos(t6))/12500 + (3*cos(t2 + t3 + t4)*cos(t5)*sin(t6))/12500))/2 + ((cos(t2 + t3 + t4)*sin(t6) + sin(t2 + t3 + t4)*cos(t5)*cos(t6))*((11*sin(t2 + t3 + t4)*sin(t6))/50000 - (11*cos(t2 + t3 + t4)*cos(t5)*cos(t6))/50000))/2 + ((sin(t2 + t3 + t4)*sin(t6) - cos(t2 + t3 + t4)*cos(t5)*cos(t6))*((11*cos(t2 + t3 + t4)*sin(t6))/50000 + (11*sin(t2 + t3 + t4)*cos(t5)*cos(t6))/50000))/2 + (((43*d5*cos(t2 + t3 + t4)*cos(t1))/100 - (37539*sin(t2 + t3 + t4)*cos(t1)*sin(t5))/5000000 - (817*cos(t2 + t3 + t4)*cos(t1)*cos(t6))/2000000 + (817*sin(t2 + t3 + t4)*cos(t1)*cos(t5)*sin(t6))/2000000 + (43*d6*sin(t2 + t3 + t4)*cos(t1)*sin(t5))/100)*(d6*(cos(t5)*sin(t1) + cos(t2 + t3 + t4)*cos(t1)*sin(t5)) - (873*cos(t5)*sin(t1))/50000 - (19*sin(t6)*(sin(t1)*sin(t5) - cos(t2 + t3 + t4)*cos(t1)*cos(t5)))/20000 + d4*sin(t1) - (873*cos(t2 + t3 + t4)*cos(t1)*sin(t5))/50000 + (19*sin(t2 + t3 + t4)*cos(t1)*cos(t6))/20000 + a3*cos(t2 + t3)*cos(t1) + a2*cos(t1)*cos(t2) - d5*sin(t2 + t3 + t4)*cos(t1)))/2 + ((d5*cos(t2 + t3 + t4)*cos(t1) - (873*sin(t2 + t3 + t4)*cos(t1)*sin(t5))/50000 - (19*cos(t2 + t3 + t4)*cos(t1)*cos(t6))/20000 + (19*sin(t2 + t3 + t4)*cos(t1)*cos(t5)*sin(t6))/20000 + d6*sin(t2 + t3 + t4)*cos(t1)*sin(t5))*((43*d6*(cos(t5)*sin(t1) + cos(t2 + t3 + t4)*cos(t1)*sin(t5)))/100 - (37539*cos(t5)*sin(t1))/5000000 - (817*sin(t6)*(sin(t1)*sin(t5) - cos(t2 + t3 + t4)*cos(t1)*cos(t5)))/2000000 + (43*d4*sin(t1))/100 - (37539*cos(t2 + t3 + t4)*cos(t1)*sin(t5))/5000000 + (817*sin(t2 + t3 + t4)*cos(t1)*cos(t6))/2000000 + (43*a3*cos(t2 + t3)*cos(t1))/100 + (43*a2*cos(t1)*cos(t2))/100 - (43*d5*sin(t2 + t3 + t4)*cos(t1))/100))/2 + (210469*a2*cos(t3 + t4))/100000000 - (957929*a3*cos(t4 + t5))/200000000 - (1967*d5^2*sin(2*t2 + 2*t3 + 2*t4))/2000 + (957929*a3*cos(2*t2 + 2*t3 + t4 - t5))/200000000 + (957929*d5*sin(2*t2 + 2*t3 + 2*t4 + t5))/100000000 + (210469*a3*cos(t4))/100000000 + (210469*a3*cos(2*t2 + 2*t3 + t4))/100000000 - (957929*a2*cos(2*t2 + t3 + t4 + t5))/200000000 + (957929*a3*cos(t4 - t5))/200000000 - (957929*a2*cos(t3 + t4 + t5))/200000000 - (957929*d5*sin(2*t2 + 2*t3 + 2*t4 - t5))/100000000 + (((43*d5*cos(t2 + t3 + t4)*sin(t1))/100 - (37539*sin(t2 + t3 + t4)*sin(t1)*sin(t5))/5000000 - (817*cos(t2 + t3 + t4)*cos(t6)*sin(t1))/2000000 + (817*sin(t2 + t3 + t4)*cos(t5)*sin(t1)*sin(t6))/2000000 + (43*d6*sin(t2 + t3 + t4)*sin(t1)*sin(t5))/100)*((19*sin(t6)*(cos(t1)*sin(t5) + cos(t2 + t3 + t4)*cos(t5)*sin(t1)))/20000 + (873*cos(t1)*cos(t5))/50000 - d6*(cos(t1)*cos(t5) - cos(t2 + t3 + t4)*sin(t1)*sin(t5)) - d4*cos(t1) - (873*cos(t2 + t3 + t4)*sin(t1)*sin(t5))/50000 + (19*sin(t2 + t3 + t4)*cos(t6)*sin(t1))/20000 + a3*cos(t2 + t3)*sin(t1) + a2*cos(t2)*sin(t1) - d5*sin(t2 + t3 + t4)*sin(t1)))/2 + ((d5*cos(t2 + t3 + t4)*sin(t1) - (873*sin(t2 + t3 + t4)*sin(t1)*sin(t5))/50000 - (19*cos(t2 + t3 + t4)*cos(t6)*sin(t1))/20000 + (19*sin(t2 + t3 + t4)*cos(t5)*sin(t1)*sin(t6))/20000 + d6*sin(t2 + t3 + t4)*sin(t1)*sin(t5))*((817*sin(t6)*(cos(t1)*sin(t5) + cos(t2 + t3 + t4)*cos(t5)*sin(t1)))/2000000 + (37539*cos(t1)*cos(t5))/5000000 - (43*d6*(cos(t1)*cos(t5) - cos(t2 + t3 + t4)*sin(t1)*sin(t5)))/100 - (43*d4*cos(t1))/100 - (37539*cos(t2 + t3 + t4)*sin(t1)*sin(t5))/5000000 + (817*sin(t2 + t3 + t4)*cos(t6)*sin(t1))/2000000 + (43*a3*cos(t2 + t3)*sin(t1))/100 + (43*a2*cos(t2)*sin(t1))/100 - (43*d5*sin(t2 + t3 + t4)*sin(t1))/100))/2 + (1967*a3*d5*cos(2*t2 + 2*t3 + t4))/2000 + (1967*a2*d5*cos(2*t2 + t3 + t4))/2000 + (1967*a2*d5*cos(t3 + t4))/2000 - (cos(t2 + t3 + t4)*sin(t2 + t3 + t4)*sin(t5)^2)/2500 + (1967*a3*d5*cos(t4))/2000) - td6*((713241*sin(t2 + t3 + t4 + t5 - t6))/800000000000 - (713241*sin(t2 + t3 + t4 + t5 + t6))/800000000000 - (713241*sin(t2 + t3 + t4 - t5 + t6))/800000000000 - (784477*sin(t2 + t3 + t4 + t5 - 2*t6))/320000000000 - (784477*sin(t2 + t3 + t4 + t5 + 2*t6))/320000000000 - (713241*sin(t2 + t3 + t4 - 2*t5 + t6))/800000000000 - (713241*sin(t2 + t3 + t4 + 2*t5 + t6))/800000000000 + (713241*sin(t2 + t3 + t4 - t5 - t6))/800000000000 + (784477*sin(t2 + t3 + t4 - t5 - 2*t6))/320000000000 + (784477*sin(t2 + t3 + t4 - t5 + 2*t6))/320000000000 - (713241*sin(t2 + t3 + t4 - 2*t5 - t6))/800000000000 - (713241*sin(t2 + t3 + t4 + 2*t5 - t6))/800000000000 - (784477*sin(t2 + t3 + t4 - 2*t5 - 2*t6))/640000000000 + (784477*sin(t2 + t3 + t4 - 2*t5 + 2*t6))/640000000000 + (784477*sin(t2 + t3 + t4 + 2*t5 - 2*t6))/640000000000 - (784477*sin(t2 + t3 + t4 + 2*t5 + 2*t6))/640000000000 + (817*d4*sin(t2 + t3 + t4 + t5 - t6))/16000000 + (817*d4*sin(t2 + t3 + t4 - t5 + t6))/16000000 - (817*d5*sin(t2 + t3 + t4 + t5 - t6))/16000000 + (817*d5*sin(t2 + t3 + t4 - t5 + t6))/16000000 - (817*d6*sin(t2 + t3 + t4 + t5 - t6))/16000000 + (817*d6*sin(t2 + t3 + t4 - t5 + t6))/16000000 + (817*d6*sin(t2 + t3 + t4 - 2*t5 + t6))/16000000 + (817*d6*sin(t2 + t3 + t4 + 2*t5 + t6))/16000000 + (817*d4*sin(t2 + t3 + t4 + t6))/8000000 + (817*d4*sin(t2 + t3 + t4 - t5 - t6))/16000000 + (817*d5*sin(t2 + t3 + t4 - t5 - t6))/16000000 - (817*d6*sin(t2 + t3 + t4 - t5 - t6))/16000000 + (817*d6*sin(t2 + t3 + t4 - 2*t5 - t6))/16000000 + (817*d6*sin(t2 + t3 + t4 + 2*t5 - t6))/16000000 - (817*d4*sin(t2 + t3 + t4 - t6))/8000000 + (817*d4*sin(t2 + t3 + t4 + t5 + t6))/16000000 - (817*d5*sin(t2 + t3 + t4 + t5 + t6))/16000000 + (817*d6*sin(t2 + t3 + t4 + t5 + t6))/16000000 - (16015523*cos(t2)*cos(t3)*cos(t4)*sin(t5))/80000000000 - (713241*cos(t2)*cos(t3)*cos(t6)*sin(t4))/200000000000 - (713241*cos(t2)*cos(t4)*cos(t6)*sin(t3))/200000000000 - (713241*cos(t3)*cos(t4)*cos(t6)*sin(t2))/200000000000 + (16015523*cos(t2)*sin(t3)*sin(t4)*sin(t5))/80000000000 + (16015523*cos(t3)*sin(t2)*sin(t4)*sin(t5))/80000000000 + (16015523*cos(t4)*sin(t2)*sin(t3)*sin(t5))/80000000000 + (713241*cos(t6)*sin(t2)*sin(t3)*sin(t4))/200000000000 + (817*d4*cos(t2)*cos(t3)*cos(t4)*sin(t6))/4000000 + (817*d6*cos(t2)*cos(t3)*cos(t6)*sin(t4))/4000000 + (817*d6*cos(t2)*cos(t4)*cos(t6)*sin(t3))/4000000 + (817*d6*cos(t3)*cos(t4)*cos(t6)*sin(t2))/4000000 - (817*d4*cos(t2)*sin(t3)*sin(t4)*sin(t6))/4000000 - (817*d4*cos(t3)*sin(t2)*sin(t4)*sin(t6))/4000000 - (817*d4*cos(t4)*sin(t2)*sin(t3)*sin(t6))/4000000 - (817*d6*cos(t6)*sin(t2)*sin(t3)*sin(t4))/4000000 - (713241*cos(t2)*cos(t3)*cos(t4)*cos(t5)*sin(t6))/200000000000 + (713241*cos(t2)*cos(t5)*sin(t3)*sin(t4)*sin(t6))/200000000000 + (713241*cos(t3)*cos(t5)*sin(t2)*sin(t4)*sin(t6))/200000000000 + (713241*cos(t4)*cos(t5)*sin(t2)*sin(t3)*sin(t6))/200000000000 + (817*d4*cos(t2)*cos(t3)*cos(t5)*cos(t6)*sin(t4))/4000000 + (817*d4*cos(t2)*cos(t4)*cos(t5)*cos(t6)*sin(t3))/4000000 + (817*d4*cos(t3)*cos(t4)*cos(t5)*cos(t6)*sin(t2))/4000000 + (817*d5*cos(t2)*cos(t3)*cos(t4)*cos(t6)*sin(t5))/4000000 + (817*d6*cos(t2)*cos(t3)*cos(t4)*cos(t5)*sin(t6))/4000000 - (817*d4*cos(t5)*cos(t6)*sin(t2)*sin(t3)*sin(t4))/4000000 - (817*d5*cos(t2)*cos(t6)*sin(t3)*sin(t4)*sin(t5))/4000000 - (817*d5*cos(t3)*cos(t6)*sin(t2)*sin(t4)*sin(t5))/4000000 - (817*d5*cos(t4)*cos(t6)*sin(t2)*sin(t3)*sin(t5))/4000000 - (817*d6*cos(t2)*cos(t5)*sin(t3)*sin(t4)*sin(t6))/4000000 - (817*d6*cos(t3)*cos(t5)*sin(t2)*sin(t4)*sin(t6))/4000000 - (817*d6*cos(t4)*cos(t5)*sin(t2)*sin(t3)*sin(t6))/4000000) + td3*((7474967197*sin(t2 + t3 + t4 - 2*t5))/40000000000000 - (49450651*sin(t2 + t3 + t4 - t5))/250000000000 - (7474967197*sin(t2 + t3 + t4 + 2*t5))/40000000000000 + (713241*sin(t2 + t3 + t4 + t5 + t6))/400000000000 - (49450651*sin(t2 + t3 + t4))/125000000000 + (713241*sin(t2 + t3 + t4 + t5 - t6))/400000000000 + (713241*sin(t2 + t3 + t4 - t5 + t6))/400000000000 - (784477*sin(t2 + t3 + t4 + t5 - 2*t6))/320000000000 + (784477*sin(t2 + t3 + t4 + t5 + 2*t6))/320000000000 + (713241*sin(t2 + t3 + t4 - 2*t5 + t6))/400000000000 + (713241*sin(t2 + t3 + t4 + 2*t5 + t6))/400000000000 - (49450651*sin(t2 + t3 + t4 + t5))/250000000000 + (713241*sin(t2 + t3 + t4 - t5 - t6))/400000000000 + (784477*sin(t2 + t3 + t4 - t5 - 2*t6))/320000000000 - (784477*sin(t2 + t3 + t4 - t5 + 2*t6))/320000000000 - (713241*sin(t2 + t3 + t4 - 2*t5 - t6))/400000000000 - (713241*sin(t2 + t3 + t4 + 2*t5 - t6))/400000000000 - (784477*sin(t2 + t3 + t4 - 2*t5 - 2*t6))/640000000000 - (784477*sin(t2 + t3 + t4 - 2*t5 + 2*t6))/640000000000 + (784477*sin(t2 + t3 + t4 + 2*t5 - 2*t6))/640000000000 + (784477*sin(t2 + t3 + t4 + 2*t5 + 2*t6))/640000000000 + (43*d6^2*sin(t2 + t3 + t4 - 2*t5))/400 - (43*d6^2*sin(t2 + t3 + t4 + 2*t5))/400 + (817*d4*sin(t2 + t3 + t4 + t5 - t6))/8000000 - (817*d4*sin(t2 + t3 + t4 - t5 + t6))/8000000 - (817*d5*sin(t2 + t3 + t4 + t5 - t6))/8000000 - (817*d5*sin(t2 + t3 + t4 - t5 + t6))/8000000 - (817*d6*sin(t2 + t3 + t4 + t5 - t6))/8000000 - (817*d6*sin(t2 + t3 + t4 - t5 + t6))/8000000 - (817*d6*sin(t2 + t3 + t4 - 2*t5 + t6))/8000000 - (817*d6*sin(t2 + t3 + t4 + 2*t5 + t6))/8000000 - (582539*d4*sin(t2 + t3 + t4 + t5))/100000000 - (817*d4*sin(t2 + t3 + t4 + t6))/4000000 + (582539*d5*sin(t2 + t3 + t4 + t5))/100000000 + (817*d4*sin(t2 + t3 + t4 - t5 - t6))/8000000 + (817*d5*sin(t2 + t3 + t4 - t5 - t6))/8000000 - (817*d6*sin(t2 + t3 + t4 - t5 - t6))/8000000 + (817*d6*sin(t2 + t3 + t4 - 2*t5 - t6))/8000000 + (817*d6*sin(t2 + t3 + t4 + 2*t5 - t6))/8000000 + (582539*d4*sin(t2 + t3 + t4 - t5))/100000000 - (817*d4*sin(t2 + t3 + t4 - t6))/4000000 + (582539*d5*sin(t2 + t3 + t4 - t5))/100000000 - (37539*d6*sin(t2 + t3 + t4 - 2*t5))/10000000 + (37539*d6*sin(t2 + t3 + t4 + 2*t5))/10000000 - (817*d4*sin(t2 + t3 + t4 + t5 + t6))/8000000 + (817*d5*sin(t2 + t3 + t4 + t5 + t6))/8000000 - (817*d6*sin(t2 + t3 + t4 + t5 + t6))/8000000 + (210469*d4*sin(t2 + t3 + t4))/50000000 + (43*d4*d6*sin(t2 + t3 + t4 - t5))/200 + (43*d5*d6*sin(t2 + t3 + t4 - t5))/200 + (2397*d4*d5*sin(t2 + t3 + t4))/1000 - (43*d4*d6*sin(t2 + t3 + t4 + t5))/200 + (43*d5*d6*sin(t2 + t3 + t4 + t5))/200) + td4*((7474967197*sin(t2 + t3 + t4 - 2*t5))/40000000000000 - (49450651*sin(t2 + t3 + t4 - t5))/250000000000 - (7474967197*sin(t2 + t3 + t4 + 2*t5))/40000000000000 + (713241*sin(t2 + t3 + t4 + t5 + t6))/400000000000 - (49450651*sin(t2 + t3 + t4))/125000000000 + (713241*sin(t2 + t3 + t4 + t5 - t6))/400000000000 + (713241*sin(t2 + t3 + t4 - t5 + t6))/400000000000 - (784477*sin(t2 + t3 + t4 + t5 - 2*t6))/320000000000 + (784477*sin(t2 + t3 + t4 + t5 + 2*t6))/320000000000 + (713241*sin(t2 + t3 + t4 - 2*t5 + t6))/400000000000 + (713241*sin(t2 + t3 + t4 + 2*t5 + t6))/400000000000 - (49450651*sin(t2 + t3 + t4 + t5))/250000000000 + (713241*sin(t2 + t3 + t4 - t5 - t6))/400000000000 + (784477*sin(t2 + t3 + t4 - t5 - 2*t6))/320000000000 - (784477*sin(t2 + t3 + t4 - t5 + 2*t6))/320000000000 - (713241*sin(t2 + t3 + t4 - 2*t5 - t6))/400000000000 - (713241*sin(t2 + t3 + t4 + 2*t5 - t6))/400000000000 - (784477*sin(t2 + t3 + t4 - 2*t5 - 2*t6))/640000000000 - (784477*sin(t2 + t3 + t4 - 2*t5 + 2*t6))/640000000000 + (784477*sin(t2 + t3 + t4 + 2*t5 - 2*t6))/640000000000 + (784477*sin(t2 + t3 + t4 + 2*t5 + 2*t6))/640000000000 + (43*d6^2*sin(t2 + t3 + t4 - 2*t5))/400 - (43*d6^2*sin(t2 + t3 + t4 + 2*t5))/400 + (817*d4*sin(t2 + t3 + t4 + t5 - t6))/8000000 - (817*d4*sin(t2 + t3 + t4 - t5 + t6))/8000000 - (817*d5*sin(t2 + t3 + t4 + t5 - t6))/8000000 - (817*d5*sin(t2 + t3 + t4 - t5 + t6))/8000000 - (817*d6*sin(t2 + t3 + t4 + t5 - t6))/8000000 - (817*d6*sin(t2 + t3 + t4 - t5 + t6))/8000000 - (817*d6*sin(t2 + t3 + t4 - 2*t5 + t6))/8000000 - (817*d6*sin(t2 + t3 + t4 + 2*t5 + t6))/8000000 - (582539*d4*sin(t2 + t3 + t4 + t5))/100000000 - (817*d4*sin(t2 + t3 + t4 + t6))/4000000 + (582539*d5*sin(t2 + t3 + t4 + t5))/100000000 + (817*d4*sin(t2 + t3 + t4 - t5 - t6))/8000000 + (817*d5*sin(t2 + t3 + t4 - t5 - t6))/8000000 - (817*d6*sin(t2 + t3 + t4 - t5 - t6))/8000000 + (817*d6*sin(t2 + t3 + t4 - 2*t5 - t6))/8000000 + (817*d6*sin(t2 + t3 + t4 + 2*t5 - t6))/8000000 + (582539*d4*sin(t2 + t3 + t4 - t5))/100000000 - (817*d4*sin(t2 + t3 + t4 - t6))/4000000 + (582539*d5*sin(t2 + t3 + t4 - t5))/100000000 - (37539*d6*sin(t2 + t3 + t4 - 2*t5))/10000000 + (37539*d6*sin(t2 + t3 + t4 + 2*t5))/10000000 - (817*d4*sin(t2 + t3 + t4 + t5 + t6))/8000000 + (817*d5*sin(t2 + t3 + t4 + t5 + t6))/8000000 - (817*d6*sin(t2 + t3 + t4 + t5 + t6))/8000000 + (210469*d4*sin(t2 + t3 + t4))/50000000 + (43*d4*d6*sin(t2 + t3 + t4 - t5))/200 + (43*d5*d6*sin(t2 + t3 + t4 - t5))/200 + (2397*d4*d5*sin(t2 + t3 + t4))/1000 - (43*d4*d6*sin(t2 + t3 + t4 + t5))/200 + (43*d5*d6*sin(t2 + t3 + t4 + t5))/200) - td5*((7474967197*sin(t2 + t3 + t4 - 2*t5))/40000000000000 + (7474967197*sin(t2 + t3 + t4 + 2*t5))/40000000000000 + (784477*sin(t2 + t3 + t4 - 2*t6))/320000000000 + (784477*sin(t2 + t3 + t4 + 2*t6))/320000000000 + (33478847947*sin(t2 + t3 + t4))/20000000000000 + (713241*sin(t2 + t3 + t4 - 2*t5 + t6))/400000000000 - (713241*sin(t2 + t3 + t4 + 2*t5 + t6))/400000000000 - (713241*sin(t2 + t3 + t4 - 2*t5 - t6))/400000000000 + (713241*sin(t2 + t3 + t4 + 2*t5 - t6))/400000000000 - (784477*sin(t2 + t3 + t4 - 2*t5 - 2*t6))/640000000000 - (784477*sin(t2 + t3 + t4 - 2*t5 + 2*t6))/640000000000 - (784477*sin(t2 + t3 + t4 + 2*t5 - 2*t6))/640000000000 - (784477*sin(t2 + t3 + t4 + 2*t5 + 2*t6))/640000000000 + (43*d6^2*sin(t2 + t3 + t4 - 2*t5))/400 + (43*d6^2*sin(t2 + t3 + t4 + 2*t5))/400 - (817*d4*sin(t2 + t3 + t4 + t5 - t6))/8000000 - (817*d4*sin(t2 + t3 + t4 - t5 + t6))/8000000 - (817*d6*sin(t2 + t3 + t4 - 2*t5 + t6))/8000000 + (817*d6*sin(t2 + t3 + t4 + 2*t5 + t6))/8000000 + (43*d6^2*sin(t2 + t3 + t4))/200 + (582539*d4*sin(t2 + t3 + t4 + t5))/100000000 + (817*d4*sin(t2 + t3 + t4 - t5 - t6))/8000000 + (817*d6*sin(t2 + t3 + t4 - 2*t5 - t6))/8000000 - (817*d6*sin(t2 + t3 + t4 + 2*t5 - t6))/8000000 + (582539*d4*sin(t2 + t3 + t4 - t5))/100000000 - (37539*d6*sin(t2 + t3 + t4 - 2*t5))/10000000 - (37539*d6*sin(t2 + t3 + t4 + 2*t5))/10000000 + (817*d4*sin(t2 + t3 + t4 + t5 + t6))/8000000 - (37539*d6*sin(t2 + t3 + t4))/5000000 + (43*d4*d6*sin(t2 + t3 + t4 - t5))/200 + (43*d4*d6*sin(t2 + t3 + t4 + t5))/200);

c15=td6*((784477*sin(t2 + t3 + t4 - 2*t6))/160000000000 - (784477*sin(t2 + t3 + t4 + 2*t6))/160000000000 - (713241*sin(t2 + t3 + t4 + t5 + t6))/800000000000 + (713241*sin(t2 + t3 + t4 + t5 - t6))/800000000000 + (713241*sin(t2 + t3 + t4 - t5 + t6))/800000000000 - (784477*sin(t2 + t3 + t4 + t5 - 2*t6))/320000000000 - (784477*sin(t2 + t3 + t4 + t5 + 2*t6))/320000000000 - (713241*sin(t2 + t3 + t4 - t5 - t6))/800000000000 - (784477*sin(t2 + t3 + t4 - t5 - 2*t6))/320000000000 - (784477*sin(t2 + t3 + t4 - t5 + 2*t6))/320000000000 + (817*a3*cos(t2 + t3 - t5 - t6))/16000000 - (817*d4*sin(t2 + t3 + t4 + t5 - t6))/16000000 + (817*d4*sin(t2 + t3 + t4 - t5 + t6))/16000000 - (817*d5*sin(t2 + t3 + t4 + t5 - t6))/16000000 - (817*d5*sin(t2 + t3 + t4 - t5 + t6))/16000000 - (817*d6*sin(t2 + t3 + t4 + t5 - t6))/16000000 - (817*d6*sin(t2 + t3 + t4 - t5 + t6))/16000000 + (817*a2*cos(t2 + t5 - t6))/16000000 + (817*a2*cos(t2 - t5 + t6))/16000000 + (817*a2*cos(t5 - t2 + t6))/16000000 + (817*a3*cos(t2 + t3 + t5 + t6))/16000000 + (817*d4*sin(t2 + t3 + t4 - t5 - t6))/16000000 - (817*d5*sin(t2 + t3 + t4 - t5 - t6))/16000000 + (817*d6*sin(t2 + t3 + t4 - t5 - t6))/16000000 + (817*a3*cos(t2 + t3 + t5 - t6))/16000000 + (817*a3*cos(t2 + t3 - t5 + t6))/16000000 - (817*d4*sin(t2 + t3 + t4 + t5 + t6))/16000000 - (817*d5*sin(t2 + t3 + t4 + t5 + t6))/16000000 + (817*d6*sin(t2 + t3 + t4 + t5 + t6))/16000000 + (817*a2*cos(t2 + t5 + t6))/16000000 + (817*a2*cos(t2)*cos(t5)*cos(t6))/4000000 + (16015523*cos(t2)*cos(t3)*cos(t5)*sin(t4))/80000000000 + (16015523*cos(t2)*cos(t4)*cos(t5)*sin(t3))/80000000000 + (16015523*cos(t3)*cos(t4)*cos(t5)*sin(t2))/80000000000 - (16015523*cos(t5)*sin(t2)*sin(t3)*sin(t4))/80000000000 + (817*a3*cos(t2)*cos(t3)*cos(t5)*cos(t6))/4000000 - (817*a3*cos(t5)*cos(t6)*sin(t2)*sin(t3))/4000000 - (713241*cos(t2)*cos(t3)*sin(t4)*sin(t5)*sin(t6))/200000000000 - (713241*cos(t2)*cos(t4)*sin(t3)*sin(t5)*sin(t6))/200000000000 - (713241*cos(t3)*cos(t4)*sin(t2)*sin(t5)*sin(t6))/200000000000 + (713241*sin(t2)*sin(t3)*sin(t4)*sin(t5)*sin(t6))/200000000000 - (817*d4*cos(t2)*cos(t3)*cos(t4)*cos(t6)*sin(t5))/4000000 - (817*d5*cos(t2)*cos(t3)*cos(t5)*cos(t6)*sin(t4))/4000000 - (817*d5*cos(t2)*cos(t4)*cos(t5)*cos(t6)*sin(t3))/4000000 - (817*d5*cos(t3)*cos(t4)*cos(t5)*cos(t6)*sin(t2))/4000000 + (817*d4*cos(t2)*cos(t6)*sin(t3)*sin(t4)*sin(t5))/4000000 + (817*d4*cos(t3)*cos(t6)*sin(t2)*sin(t4)*sin(t5))/4000000 + (817*d4*cos(t4)*cos(t6)*sin(t2)*sin(t3)*sin(t5))/4000000 + (817*d5*cos(t5)*cos(t6)*sin(t2)*sin(t3)*sin(t4))/4000000 + (817*d6*cos(t2)*cos(t3)*sin(t4)*sin(t5)*sin(t6))/4000000 + (817*d6*cos(t2)*cos(t4)*sin(t3)*sin(t5)*sin(t6))/4000000 + (817*d6*cos(t3)*cos(t4)*sin(t2)*sin(t5)*sin(t6))/4000000 - (817*d6*sin(t2)*sin(t3)*sin(t4)*sin(t5)*sin(t6))/4000000) + td1*((49450651*sin(2*t2 + 2*t3 + 2*t4 - t5))/500000000000 - (1966511423*sin(2*t2 + 2*t3 + 2*t4 - 2*t5))/20000000000000 + (1966511423*sin(2*t2 + 2*t3 + 2*t4 + 2*t5))/20000000000000 - (1966511423*sin(2*t5))/10000000000000 + (49450651*sin(2*t2 + 2*t3 + 2*t4 + t5))/500000000000 + (957929*a2*cos(2*t2 + t3 + t4 - t5))/200000000 + (957929*a3*cos(2*t2 + 2*t3 + t4 + t5))/200000000 - (((817*sin(t6)*(cos(t5)*sin(t1) + cos(t2 + t3 + t4)*cos(t1)*sin(t5)))/2000000 - (37539*sin(t1)*sin(t5))/5000000 + (43*d6*(sin(t1)*sin(t5) - cos(t2 + t3 + t4)*cos(t1)*cos(t5)))/100 + (37539*cos(t2 + t3 + t4)*cos(t1)*cos(t5))/5000000)*(d6*(cos(t5)*sin(t1) + cos(t2 + t3 + t4)*cos(t1)*sin(t5)) - (873*cos(t5)*sin(t1))/50000 - (19*sin(t6)*(sin(t1)*sin(t5) - cos(t2 + t3 + t4)*cos(t1)*cos(t5)))/20000 + d4*sin(t1) - (873*cos(t2 + t3 + t4)*cos(t1)*sin(t5))/50000 + (19*sin(t2 + t3 + t4)*cos(t1)*cos(t6))/20000 + a3*cos(t2 + t3)*cos(t1) + a2*cos(t1)*cos(t2) - d5*sin(t2 + t3 + t4)*cos(t1)))/2 - (((19*sin(t6)*(cos(t5)*sin(t1) + cos(t2 + t3 + t4)*cos(t1)*sin(t5)))/20000 - (873*sin(t1)*sin(t5))/50000 + d6*(sin(t1)*sin(t5) - cos(t2 + t3 + t4)*cos(t1)*cos(t5)) + (873*cos(t2 + t3 + t4)*cos(t1)*cos(t5))/50000)*((43*d6*(cos(t5)*sin(t1) + cos(t2 + t3 + t4)*cos(t1)*sin(t5)))/100 - (37539*cos(t5)*sin(t1))/5000000 - (817*sin(t6)*(sin(t1)*sin(t5) - cos(t2 + t3 + t4)*cos(t1)*cos(t5)))/2000000 + (43*d4*sin(t1))/100 - (37539*cos(t2 + t3 + t4)*cos(t1)*sin(t5))/5000000 + (817*sin(t2 + t3 + t4)*cos(t1)*cos(t6))/2000000 + (43*a3*cos(t2 + t3)*cos(t1))/100 + (43*a2*cos(t1)*cos(t2))/100 - (43*d5*sin(t2 + t3 + t4)*cos(t1))/100))/2 + (957929*a2*cos(t3 + t4 - t5))/200000000 + (((817*sin(t6)*(cos(t1)*cos(t5) - cos(t2 + t3 + t4)*sin(t1)*sin(t5)))/2000000 - (37539*cos(t1)*sin(t5))/5000000 + (43*d6*(cos(t1)*sin(t5) + cos(t2 + t3 + t4)*cos(t5)*sin(t1)))/100 - (37539*cos(t2 + t3 + t4)*cos(t5)*sin(t1))/5000000)*((19*sin(t6)*(cos(t1)*sin(t5) + cos(t2 + t3 + t4)*cos(t5)*sin(t1)))/20000 + (873*cos(t1)*cos(t5))/50000 - d6*(cos(t1)*cos(t5) - cos(t2 + t3 + t4)*sin(t1)*sin(t5)) - d4*cos(t1) - (873*cos(t2 + t3 + t4)*sin(t1)*sin(t5))/50000 + (19*sin(t2 + t3 + t4)*cos(t6)*sin(t1))/20000 + a3*cos(t2 + t3)*sin(t1) + a2*cos(t2)*sin(t1) - d5*sin(t2 + t3 + t4)*sin(t1)))/2 + (((19*sin(t6)*(cos(t1)*cos(t5) - cos(t2 + t3 + t4)*sin(t1)*sin(t5)))/20000 - (873*cos(t1)*sin(t5))/50000 + d6*(cos(t1)*sin(t5) + cos(t2 + t3 + t4)*cos(t5)*sin(t1)) - (873*cos(t2 + t3 + t4)*cos(t5)*sin(t1))/50000)*((817*sin(t6)*(cos(t1)*sin(t5) + cos(t2 + t3 + t4)*cos(t5)*sin(t1)))/2000000 + (37539*cos(t1)*cos(t5))/5000000 - (43*d6*(cos(t1)*cos(t5) - cos(t2 + t3 + t4)*sin(t1)*sin(t5)))/100 - (43*d4*cos(t1))/100 - (37539*cos(t2 + t3 + t4)*sin(t1)*sin(t5))/5000000 + (817*sin(t2 + t3 + t4)*cos(t6)*sin(t1))/2000000 + (43*a3*cos(t2 + t3)*sin(t1))/100 + (43*a2*cos(t2)*sin(t1))/100 - (43*d5*sin(t2 + t3 + t4)*sin(t1))/100))/2 + (957929*a3*cos(t4 + t5))/200000000 + (957929*a3*cos(2*t2 + 2*t3 + t4 - t5))/200000000 - (957929*d5*sin(2*t2 + 2*t3 + 2*t4 + t5))/200000000 - (957929*d4*sin(t5))/50000000 + (957929*a2*cos(2*t2 + t3 + t4 + t5))/200000000 + (957929*a3*cos(t4 - t5))/200000000 + (957929*a2*cos(t3 + t4 + t5))/200000000 - (957929*d5*sin(2*t2 + 2*t3 + 2*t4 - t5))/200000000 + (sin(t2 + t3 + t4)^2*cos(t5)*sin(t5))/2500 - (11*sin(t2 + t3 + t4)*cos(t6)*sin(t5)*(cos(t2 + t3 + t4)*sin(t6) + sin(t2 + t3 + t4)*cos(t5)*cos(t6)))/100000 - (sin(t2 + t3 + t4)*cos(t6)*sin(t5)*((11*cos(t2 + t3 + t4)*sin(t6))/50000 + (11*sin(t2 + t3 + t4)*cos(t5)*cos(t6))/50000))/2 + (3*sin(t2 + t3 + t4)*sin(t5)*sin(t6)*(cos(t2 + t3 + t4)*cos(t6) - sin(t2 + t3 + t4)*cos(t5)*sin(t6)))/25000 + (sin(t2 + t3 + t4)*sin(t5)*sin(t6)*((3*cos(t2 + t3 + t4)*cos(t6))/12500 - (3*sin(t2 + t3 + t4)*cos(t5)*sin(t6))/12500))/2) + td5*((49450651*sin(t2 + t3 + t4 - t5))/250000000000 - (713241*sin(t2 + t3 + t4 + t5 + t6))/400000000000 - (713241*sin(t2 + t3 + t4 + t5 - t6))/400000000000 - (713241*sin(t2 + t3 + t4 - t5 + t6))/400000000000 + (784477*sin(t2 + t3 + t4 + t5 - 2*t6))/320000000000 - (784477*sin(t2 + t3 + t4 + t5 + 2*t6))/320000000000 + (49450651*sin(t2 + t3 + t4 + t5))/250000000000 - (713241*sin(t2 + t3 + t4 - t5 - t6))/400000000000 - (784477*sin(t2 + t3 + t4 - t5 - 2*t6))/320000000000 + (784477*sin(t2 + t3 + t4 - t5 + 2*t6))/320000000000 + (817*a3*cos(t2 + t3 - t5 - t6))/8000000 + (817*d4*sin(t2 + t3 + t4 + t5 - t6))/8000000 - (817*d4*sin(t2 + t3 + t4 - t5 + t6))/8000000 + (817*d5*sin(t2 + t3 + t4 + t5 - t6))/8000000 + (817*d5*sin(t2 + t3 + t4 - t5 + t6))/8000000 + (817*d6*sin(t2 + t3 + t4 + t5 - t6))/8000000 + (817*d6*sin(t2 + t3 + t4 - t5 + t6))/8000000 + (582539*a3*cos(t2 + t3 - t5))/100000000 - (817*a2*cos(t2 + t5 - t6))/8000000 - (817*a2*cos(t2 - t5 + t6))/8000000 + (817*a2*cos(t5 - t2 + t6))/8000000 + (817*a3*cos(t2 + t3 + t5 + t6))/8000000 - (582539*d4*sin(t2 + t3 + t4 + t5))/100000000 - (582539*d5*sin(t2 + t3 + t4 + t5))/100000000 + (582539*a2*cos(t2 + t5))/100000000 + (817*d4*sin(t2 + t3 + t4 - t5 - t6))/8000000 - (817*d5*sin(t2 + t3 + t4 - t5 - t6))/8000000 + (817*d6*sin(t2 + t3 + t4 - t5 - t6))/8000000 - (817*a3*cos(t2 + t3 + t5 - t6))/8000000 - (817*a3*cos(t2 + t3 - t5 + t6))/8000000 + (582539*d4*sin(t2 + t3 + t4 - t5))/100000000 - (582539*d5*sin(t2 + t3 + t4 - t5))/100000000 + (582539*a2*cos(t2 - t5))/100000000 - (817*d4*sin(t2 + t3 + t4 + t5 + t6))/8000000 - (817*d5*sin(t2 + t3 + t4 + t5 + t6))/8000000 + (817*d6*sin(t2 + t3 + t4 + t5 + t6))/8000000 + (582539*a3*cos(t2 + t3 + t5))/100000000 + (817*a2*cos(t2 + t5 + t6))/8000000 + (43*d4*d6*sin(t2 + t3 + t4 - t5))/200 - (43*d5*d6*sin(t2 + t3 + t4 - t5))/200 + (43*a2*d6*cos(t2 - t5))/200 + (43*a3*d6*cos(t2 + t3 + t5))/200 + (43*a3*d6*cos(t2 + t3 - t5))/200 - (43*d4*d6*sin(t2 + t3 + t4 + t5))/200 - (43*d5*d6*sin(t2 + t3 + t4 + t5))/200 + (43*a2*d6*cos(t2 + t5))/200) - td2*((7474967197*sin(t2 + t3 + t4 - 2*t5))/40000000000000 + (7474967197*sin(t2 + t3 + t4 + 2*t5))/40000000000000 + (784477*sin(t2 + t3 + t4 - 2*t6))/320000000000 + (784477*sin(t2 + t3 + t4 + 2*t6))/320000000000 + (33478847947*sin(t2 + t3 + t4))/20000000000000 + (713241*sin(t2 + t3 + t4 - 2*t5 + t6))/400000000000 - (713241*sin(t2 + t3 + t4 + 2*t5 + t6))/400000000000 - (713241*sin(t2 + t3 + t4 - 2*t5 - t6))/400000000000 + (713241*sin(t2 + t3 + t4 + 2*t5 - t6))/400000000000 - (784477*sin(t2 + t3 + t4 - 2*t5 - 2*t6))/640000000000 - (784477*sin(t2 + t3 + t4 - 2*t5 + 2*t6))/640000000000 - (784477*sin(t2 + t3 + t4 + 2*t5 - 2*t6))/640000000000 - (784477*sin(t2 + t3 + t4 + 2*t5 + 2*t6))/640000000000 + (43*d6^2*sin(t2 + t3 + t4 - 2*t5))/400 + (43*d6^2*sin(t2 + t3 + t4 + 2*t5))/400 - (817*d4*sin(t2 + t3 + t4 + t5 - t6))/8000000 - (817*d4*sin(t2 + t3 + t4 - t5 + t6))/8000000 - (817*d6*sin(t2 + t3 + t4 - 2*t5 + t6))/8000000 + (817*d6*sin(t2 + t3 + t4 + 2*t5 + t6))/8000000 + (43*d6^2*sin(t2 + t3 + t4))/200 + (582539*d4*sin(t2 + t3 + t4 + t5))/100000000 + (817*d4*sin(t2 + t3 + t4 - t5 - t6))/8000000 + (817*d6*sin(t2 + t3 + t4 - 2*t5 - t6))/8000000 - (817*d6*sin(t2 + t3 + t4 + 2*t5 - t6))/8000000 + (582539*d4*sin(t2 + t3 + t4 - t5))/100000000 - (37539*d6*sin(t2 + t3 + t4 - 2*t5))/10000000 - (37539*d6*sin(t2 + t3 + t4 + 2*t5))/10000000 + (817*d4*sin(t2 + t3 + t4 + t5 + t6))/8000000 - (37539*d6*sin(t2 + t3 + t4))/5000000 + (43*d4*d6*sin(t2 + t3 + t4 - t5))/200 + (43*d4*d6*sin(t2 + t3 + t4 + t5))/200) - td3*((7474967197*sin(t2 + t3 + t4 - 2*t5))/40000000000000 + (7474967197*sin(t2 + t3 + t4 + 2*t5))/40000000000000 + (784477*sin(t2 + t3 + t4 - 2*t6))/320000000000 + (784477*sin(t2 + t3 + t4 + 2*t6))/320000000000 + (33478847947*sin(t2 + t3 + t4))/20000000000000 + (713241*sin(t2 + t3 + t4 - 2*t5 + t6))/400000000000 - (713241*sin(t2 + t3 + t4 + 2*t5 + t6))/400000000000 - (713241*sin(t2 + t3 + t4 - 2*t5 - t6))/400000000000 + (713241*sin(t2 + t3 + t4 + 2*t5 - t6))/400000000000 - (784477*sin(t2 + t3 + t4 - 2*t5 - 2*t6))/640000000000 - (784477*sin(t2 + t3 + t4 - 2*t5 + 2*t6))/640000000000 - (784477*sin(t2 + t3 + t4 + 2*t5 - 2*t6))/640000000000 - (784477*sin(t2 + t3 + t4 + 2*t5 + 2*t6))/640000000000 + (43*d6^2*sin(t2 + t3 + t4 - 2*t5))/400 + (43*d6^2*sin(t2 + t3 + t4 + 2*t5))/400 - (817*d4*sin(t2 + t3 + t4 + t5 - t6))/8000000 - (817*d4*sin(t2 + t3 + t4 - t5 + t6))/8000000 - (817*d6*sin(t2 + t3 + t4 - 2*t5 + t6))/8000000 + (817*d6*sin(t2 + t3 + t4 + 2*t5 + t6))/8000000 + (43*d6^2*sin(t2 + t3 + t4))/200 + (582539*d4*sin(t2 + t3 + t4 + t5))/100000000 + (817*d4*sin(t2 + t3 + t4 - t5 - t6))/8000000 + (817*d6*sin(t2 + t3 + t4 - 2*t5 - t6))/8000000 - (817*d6*sin(t2 + t3 + t4 + 2*t5 - t6))/8000000 + (582539*d4*sin(t2 + t3 + t4 - t5))/100000000 - (37539*d6*sin(t2 + t3 + t4 - 2*t5))/10000000 - (37539*d6*sin(t2 + t3 + t4 + 2*t5))/10000000 + (817*d4*sin(t2 + t3 + t4 + t5 + t6))/8000000 - (37539*d6*sin(t2 + t3 + t4))/5000000 + (43*d4*d6*sin(t2 + t3 + t4 - t5))/200 + (43*d4*d6*sin(t2 + t3 + t4 + t5))/200) - td4*((7474967197*sin(t2 + t3 + t4 - 2*t5))/40000000000000 + (7474967197*sin(t2 + t3 + t4 + 2*t5))/40000000000000 + (784477*sin(t2 + t3 + t4 - 2*t6))/320000000000 + (784477*sin(t2 + t3 + t4 + 2*t6))/320000000000 + (33478847947*sin(t2 + t3 + t4))/20000000000000 + (713241*sin(t2 + t3 + t4 - 2*t5 + t6))/400000000000 - (713241*sin(t2 + t3 + t4 + 2*t5 + t6))/400000000000 - (713241*sin(t2 + t3 + t4 - 2*t5 - t6))/400000000000 + (713241*sin(t2 + t3 + t4 + 2*t5 - t6))/400000000000 - (784477*sin(t2 + t3 + t4 - 2*t5 - 2*t6))/640000000000 - (784477*sin(t2 + t3 + t4 - 2*t5 + 2*t6))/640000000000 - (784477*sin(t2 + t3 + t4 + 2*t5 - 2*t6))/640000000000 - (784477*sin(t2 + t3 + t4 + 2*t5 + 2*t6))/640000000000 + (43*d6^2*sin(t2 + t3 + t4 - 2*t5))/400 + (43*d6^2*sin(t2 + t3 + t4 + 2*t5))/400 - (817*d4*sin(t2 + t3 + t4 + t5 - t6))/8000000 - (817*d4*sin(t2 + t3 + t4 - t5 + t6))/8000000 - (817*d6*sin(t2 + t3 + t4 - 2*t5 + t6))/8000000 + (817*d6*sin(t2 + t3 + t4 + 2*t5 + t6))/8000000 + (43*d6^2*sin(t2 + t3 + t4))/200 + (582539*d4*sin(t2 + t3 + t4 + t5))/100000000 + (817*d4*sin(t2 + t3 + t4 - t5 - t6))/8000000 + (817*d6*sin(t2 + t3 + t4 - 2*t5 - t6))/8000000 - (817*d6*sin(t2 + t3 + t4 + 2*t5 - t6))/8000000 + (582539*d4*sin(t2 + t3 + t4 - t5))/100000000 - (37539*d6*sin(t2 + t3 + t4 - 2*t5))/10000000 - (37539*d6*sin(t2 + t3 + t4 + 2*t5))/10000000 + (817*d4*sin(t2 + t3 + t4 + t5 + t6))/8000000 - (37539*d6*sin(t2 + t3 + t4))/5000000 + (43*d4*d6*sin(t2 + t3 + t4 - t5))/200 + (43*d4*d6*sin(t2 + t3 + t4 + t5))/200);

c16=td6*((713241*cos(t2)*cos(t3)*cos(t4)*sin(t6))/100000000000 - (817*a2*cos(t2)*sin(t5)*sin(t6))/2000000 - (713241*cos(t2)*sin(t3)*sin(t4)*sin(t6))/100000000000 - (713241*cos(t3)*sin(t2)*sin(t4)*sin(t6))/100000000000 - (713241*cos(t4)*sin(t2)*sin(t3)*sin(t6))/100000000000 - (817*d4*cos(t2)*cos(t3)*cos(t6)*sin(t4))/2000000 - (817*d4*cos(t2)*cos(t4)*cos(t6)*sin(t3))/2000000 - (817*d4*cos(t3)*cos(t4)*cos(t6)*sin(t2))/2000000 - (817*d6*cos(t2)*cos(t3)*cos(t4)*sin(t6))/2000000 - (817*a3*cos(t2)*cos(t3)*sin(t5)*sin(t6))/2000000 + (817*d4*cos(t6)*sin(t2)*sin(t3)*sin(t4))/2000000 + (817*d6*cos(t2)*sin(t3)*sin(t4)*sin(t6))/2000000 + (817*d6*cos(t3)*sin(t2)*sin(t4)*sin(t6))/2000000 + (817*d6*cos(t4)*sin(t2)*sin(t3)*sin(t6))/2000000 + (817*a3*sin(t2)*sin(t3)*sin(t5)*sin(t6))/2000000 + (713241*cos(t2)*cos(t3)*cos(t5)*cos(t6)*sin(t4))/100000000000 + (713241*cos(t2)*cos(t4)*cos(t5)*cos(t6)*sin(t3))/100000000000 + (713241*cos(t3)*cos(t4)*cos(t5)*cos(t6)*sin(t2))/100000000000 - (713241*cos(t5)*cos(t6)*sin(t2)*sin(t3)*sin(t4))/100000000000 - (817*d4*cos(t2)*cos(t3)*cos(t4)*cos(t5)*sin(t6))/2000000 - (817*d6*cos(t2)*cos(t3)*cos(t5)*cos(t6)*sin(t4))/2000000 - (817*d6*cos(t2)*cos(t4)*cos(t5)*cos(t6)*sin(t3))/2000000 - (817*d6*cos(t3)*cos(t4)*cos(t5)*cos(t6)*sin(t2))/2000000 + (817*d4*cos(t2)*cos(t5)*sin(t3)*sin(t4)*sin(t6))/2000000 + (817*d4*cos(t3)*cos(t5)*sin(t2)*sin(t4)*sin(t6))/2000000 + (817*d4*cos(t4)*cos(t5)*sin(t2)*sin(t3)*sin(t6))/2000000 + (817*d5*cos(t2)*cos(t3)*sin(t4)*sin(t5)*sin(t6))/2000000 + (817*d5*cos(t2)*cos(t4)*sin(t3)*sin(t5)*sin(t6))/2000000 + (817*d5*cos(t3)*cos(t4)*sin(t2)*sin(t5)*sin(t6))/2000000 + (817*d6*cos(t5)*cos(t6)*sin(t2)*sin(t3)*sin(t4))/2000000 - (817*d5*sin(t2)*sin(t3)*sin(t4)*sin(t5)*sin(t6))/2000000) - td4*((713241*sin(t2 + t3 + t4 + t5 - t6))/800000000000 - (713241*sin(t2 + t3 + t4 + t5 + t6))/800000000000 - (713241*sin(t2 + t3 + t4 - t5 + t6))/800000000000 - (784477*sin(t2 + t3 + t4 + t5 - 2*t6))/320000000000 - (784477*sin(t2 + t3 + t4 + t5 + 2*t6))/320000000000 - (713241*sin(t2 + t3 + t4 - 2*t5 + t6))/800000000000 - (713241*sin(t2 + t3 + t4 + 2*t5 + t6))/800000000000 + (713241*sin(t2 + t3 + t4 - t5 - t6))/800000000000 + (784477*sin(t2 + t3 + t4 - t5 - 2*t6))/320000000000 + (784477*sin(t2 + t3 + t4 - t5 + 2*t6))/320000000000 - (713241*sin(t2 + t3 + t4 - 2*t5 - t6))/800000000000 - (713241*sin(t2 + t3 + t4 + 2*t5 - t6))/800000000000 - (784477*sin(t2 + t3 + t4 - 2*t5 - 2*t6))/640000000000 + (784477*sin(t2 + t3 + t4 - 2*t5 + 2*t6))/640000000000 + (784477*sin(t2 + t3 + t4 + 2*t5 - 2*t6))/640000000000 - (784477*sin(t2 + t3 + t4 + 2*t5 + 2*t6))/640000000000 + (817*d4*sin(t2 + t3 + t4 + t5 - t6))/16000000 + (817*d4*sin(t2 + t3 + t4 - t5 + t6))/16000000 - (817*d5*sin(t2 + t3 + t4 + t5 - t6))/16000000 + (817*d5*sin(t2 + t3 + t4 - t5 + t6))/16000000 - (817*d6*sin(t2 + t3 + t4 + t5 - t6))/16000000 + (817*d6*sin(t2 + t3 + t4 - t5 + t6))/16000000 + (817*d6*sin(t2 + t3 + t4 - 2*t5 + t6))/16000000 + (817*d6*sin(t2 + t3 + t4 + 2*t5 + t6))/16000000 + (817*d4*sin(t2 + t3 + t4 + t6))/8000000 + (817*d4*sin(t2 + t3 + t4 - t5 - t6))/16000000 + (817*d5*sin(t2 + t3 + t4 - t5 - t6))/16000000 - (817*d6*sin(t2 + t3 + t4 - t5 - t6))/16000000 + (817*d6*sin(t2 + t3 + t4 - 2*t5 - t6))/16000000 + (817*d6*sin(t2 + t3 + t4 + 2*t5 - t6))/16000000 - (817*d4*sin(t2 + t3 + t4 - t6))/8000000 + (817*d4*sin(t2 + t3 + t4 + t5 + t6))/16000000 - (817*d5*sin(t2 + t3 + t4 + t5 + t6))/16000000 + (817*d6*sin(t2 + t3 + t4 + t5 + t6))/16000000 - (16015523*cos(t2)*cos(t3)*cos(t4)*sin(t5))/80000000000 - (713241*cos(t2)*cos(t3)*cos(t6)*sin(t4))/200000000000 - (713241*cos(t2)*cos(t4)*cos(t6)*sin(t3))/200000000000 - (713241*cos(t3)*cos(t4)*cos(t6)*sin(t2))/200000000000 + (16015523*cos(t2)*sin(t3)*sin(t4)*sin(t5))/80000000000 + (16015523*cos(t3)*sin(t2)*sin(t4)*sin(t5))/80000000000 + (16015523*cos(t4)*sin(t2)*sin(t3)*sin(t5))/80000000000 + (713241*cos(t6)*sin(t2)*sin(t3)*sin(t4))/200000000000 + (817*d4*cos(t2)*cos(t3)*cos(t4)*sin(t6))/4000000 + (817*d6*cos(t2)*cos(t3)*cos(t6)*sin(t4))/4000000 + (817*d6*cos(t2)*cos(t4)*cos(t6)*sin(t3))/4000000 + (817*d6*cos(t3)*cos(t4)*cos(t6)*sin(t2))/4000000 - (817*d4*cos(t2)*sin(t3)*sin(t4)*sin(t6))/4000000 - (817*d4*cos(t3)*sin(t2)*sin(t4)*sin(t6))/4000000 - (817*d4*cos(t4)*sin(t2)*sin(t3)*sin(t6))/4000000 - (817*d6*cos(t6)*sin(t2)*sin(t3)*sin(t4))/4000000 - (713241*cos(t2)*cos(t3)*cos(t4)*cos(t5)*sin(t6))/200000000000 + (713241*cos(t2)*cos(t5)*sin(t3)*sin(t4)*sin(t6))/200000000000 + (713241*cos(t3)*cos(t5)*sin(t2)*sin(t4)*sin(t6))/200000000000 + (713241*cos(t4)*cos(t5)*sin(t2)*sin(t3)*sin(t6))/200000000000 + (817*d4*cos(t2)*cos(t3)*cos(t5)*cos(t6)*sin(t4))/4000000 + (817*d4*cos(t2)*cos(t4)*cos(t5)*cos(t6)*sin(t3))/4000000 + (817*d4*cos(t3)*cos(t4)*cos(t5)*cos(t6)*sin(t2))/4000000 + (817*d5*cos(t2)*cos(t3)*cos(t4)*cos(t6)*sin(t5))/4000000 + (817*d6*cos(t2)*cos(t3)*cos(t4)*cos(t5)*sin(t6))/4000000 - (817*d4*cos(t5)*cos(t6)*sin(t2)*sin(t3)*sin(t4))/4000000 - (817*d5*cos(t2)*cos(t6)*sin(t3)*sin(t4)*sin(t5))/4000000 - (817*d5*cos(t3)*cos(t6)*sin(t2)*sin(t4)*sin(t5))/4000000 - (817*d5*cos(t4)*cos(t6)*sin(t2)*sin(t3)*sin(t5))/4000000 - (817*d6*cos(t2)*cos(t5)*sin(t3)*sin(t4)*sin(t6))/4000000 - (817*d6*cos(t3)*cos(t5)*sin(t2)*sin(t4)*sin(t6))/4000000 - (817*d6*cos(t4)*cos(t5)*sin(t2)*sin(t3)*sin(t6))/4000000) + td5*((784477*sin(t2 + t3 + t4 - 2*t6))/160000000000 - (784477*sin(t2 + t3 + t4 + 2*t6))/160000000000 - (713241*sin(t2 + t3 + t4 + t5 + t6))/800000000000 + (713241*sin(t2 + t3 + t4 + t5 - t6))/800000000000 + (713241*sin(t2 + t3 + t4 - t5 + t6))/800000000000 - (784477*sin(t2 + t3 + t4 + t5 - 2*t6))/320000000000 - (784477*sin(t2 + t3 + t4 + t5 + 2*t6))/320000000000 - (713241*sin(t2 + t3 + t4 - t5 - t6))/800000000000 - (784477*sin(t2 + t3 + t4 - t5 - 2*t6))/320000000000 - (784477*sin(t2 + t3 + t4 - t5 + 2*t6))/320000000000 + (817*a3*cos(t2 + t3 - t5 - t6))/16000000 - (817*d4*sin(t2 + t3 + t4 + t5 - t6))/16000000 + (817*d4*sin(t2 + t3 + t4 - t5 + t6))/16000000 - (817*d5*sin(t2 + t3 + t4 + t5 - t6))/16000000 - (817*d5*sin(t2 + t3 + t4 - t5 + t6))/16000000 - (817*d6*sin(t2 + t3 + t4 + t5 - t6))/16000000 - (817*d6*sin(t2 + t3 + t4 - t5 + t6))/16000000 + (817*a2*cos(t2 + t5 - t6))/16000000 + (817*a2*cos(t2 - t5 + t6))/16000000 + (817*a2*cos(t5 - t2 + t6))/16000000 + (817*a3*cos(t2 + t3 + t5 + t6))/16000000 + (817*d4*sin(t2 + t3 + t4 - t5 - t6))/16000000 - (817*d5*sin(t2 + t3 + t4 - t5 - t6))/16000000 + (817*d6*sin(t2 + t3 + t4 - t5 - t6))/16000000 + (817*a3*cos(t2 + t3 + t5 - t6))/16000000 + (817*a3*cos(t2 + t3 - t5 + t6))/16000000 - (817*d4*sin(t2 + t3 + t4 + t5 + t6))/16000000 - (817*d5*sin(t2 + t3 + t4 + t5 + t6))/16000000 + (817*d6*sin(t2 + t3 + t4 + t5 + t6))/16000000 + (817*a2*cos(t2 + t5 + t6))/16000000 + (817*a2*cos(t2)*cos(t5)*cos(t6))/4000000 + (16015523*cos(t2)*cos(t3)*cos(t5)*sin(t4))/80000000000 + (16015523*cos(t2)*cos(t4)*cos(t5)*sin(t3))/80000000000 + (16015523*cos(t3)*cos(t4)*cos(t5)*sin(t2))/80000000000 - (16015523*cos(t5)*sin(t2)*sin(t3)*sin(t4))/80000000000 + (817*a3*cos(t2)*cos(t3)*cos(t5)*cos(t6))/4000000 - (817*a3*cos(t5)*cos(t6)*sin(t2)*sin(t3))/4000000 - (713241*cos(t2)*cos(t3)*sin(t4)*sin(t5)*sin(t6))/200000000000 - (713241*cos(t2)*cos(t4)*sin(t3)*sin(t5)*sin(t6))/200000000000 - (713241*cos(t3)*cos(t4)*sin(t2)*sin(t5)*sin(t6))/200000000000 + (713241*sin(t2)*sin(t3)*sin(t4)*sin(t5)*sin(t6))/200000000000 - (817*d4*cos(t2)*cos(t3)*cos(t4)*cos(t6)*sin(t5))/4000000 - (817*d5*cos(t2)*cos(t3)*cos(t5)*cos(t6)*sin(t4))/4000000 - (817*d5*cos(t2)*cos(t4)*cos(t5)*cos(t6)*sin(t3))/4000000 - (817*d5*cos(t3)*cos(t4)*cos(t5)*cos(t6)*sin(t2))/4000000 + (817*d4*cos(t2)*cos(t6)*sin(t3)*sin(t4)*sin(t5))/4000000 + (817*d4*cos(t3)*cos(t6)*sin(t2)*sin(t4)*sin(t5))/4000000 + (817*d4*cos(t4)*cos(t6)*sin(t2)*sin(t3)*sin(t5))/4000000 + (817*d5*cos(t5)*cos(t6)*sin(t2)*sin(t3)*sin(t4))/4000000 + (817*d6*cos(t2)*cos(t3)*sin(t4)*sin(t5)*sin(t6))/4000000 + (817*d6*cos(t2)*cos(t4)*sin(t3)*sin(t5)*sin(t6))/4000000 + (817*d6*cos(t3)*cos(t4)*sin(t2)*sin(t5)*sin(t6))/4000000 - (817*d6*sin(t2)*sin(t3)*sin(t4)*sin(t5)*sin(t6))/4000000) - td1*(((cos(t2 + t3 + t4)*sin(t6) + sin(t2 + t3 + t4)*cos(t5)*cos(t6))*((3*cos(t2 + t3 + t4)*cos(t6))/12500 - (3*sin(t2 + t3 + t4)*cos(t5)*sin(t6))/12500))/2 + ((cos(t2 + t3 + t4)*cos(t6) - sin(t2 + t3 + t4)*cos(t5)*sin(t6))*((3*cos(t2 + t3 + t4)*sin(t6))/12500 + (3*sin(t2 + t3 + t4)*cos(t5)*cos(t6))/12500))/2 - ((cos(t2 + t3 + t4)*sin(t6) + sin(t2 + t3 + t4)*cos(t5)*cos(t6))*((11*cos(t2 + t3 + t4)*cos(t6))/50000 - (11*sin(t2 + t3 + t4)*cos(t5)*sin(t6))/50000))/2 - ((cos(t2 + t3 + t4)*cos(t6) - sin(t2 + t3 + t4)*cos(t5)*sin(t6))*((11*cos(t2 + t3 + t4)*sin(t6))/50000 + (11*sin(t2 + t3 + t4)*cos(t5)*cos(t6))/50000))/2 + (((817*cos(t6)*(sin(t1)*sin(t5) - cos(t2 + t3 + t4)*cos(t1)*cos(t5)))/2000000 + (817*sin(t2 + t3 + t4)*cos(t1)*sin(t6))/2000000)*(d6*(cos(t5)*sin(t1) + cos(t2 + t3 + t4)*cos(t1)*sin(t5)) - (873*cos(t5)*sin(t1))/50000 - (19*sin(t6)*(sin(t1)*sin(t5) - cos(t2 + t3 + t4)*cos(t1)*cos(t5)))/20000 + d4*sin(t1) - (873*cos(t2 + t3 + t4)*cos(t1)*sin(t5))/50000 + (19*sin(t2 + t3 + t4)*cos(t1)*cos(t6))/20000 + a3*cos(t2 + t3)*cos(t1) + a2*cos(t1)*cos(t2) - d5*sin(t2 + t3 + t4)*cos(t1)))/2 + (((19*cos(t6)*(sin(t1)*sin(t5) - cos(t2 + t3 + t4)*cos(t1)*cos(t5)))/20000 + (19*sin(t2 + t3 + t4)*cos(t1)*sin(t6))/20000)*((43*d6*(cos(t5)*sin(t1) + cos(t2 + t3 + t4)*cos(t1)*sin(t5)))/100 - (37539*cos(t5)*sin(t1))/5000000 - (817*sin(t6)*(sin(t1)*sin(t5) - cos(t2 + t3 + t4)*cos(t1)*cos(t5)))/2000000 + (43*d4*sin(t1))/100 - (37539*cos(t2 + t3 + t4)*cos(t1)*sin(t5))/5000000 + (817*sin(t2 + t3 + t4)*cos(t1)*cos(t6))/2000000 + (43*a3*cos(t2 + t3)*cos(t1))/100 + (43*a2*cos(t1)*cos(t2))/100 - (43*d5*sin(t2 + t3 + t4)*cos(t1))/100))/2 - (((817*cos(t6)*(cos(t1)*sin(t5) + cos(t2 + t3 + t4)*cos(t5)*sin(t1)))/2000000 - (817*sin(t2 + t3 + t4)*sin(t1)*sin(t6))/2000000)*((19*sin(t6)*(cos(t1)*sin(t5) + cos(t2 + t3 + t4)*cos(t5)*sin(t1)))/20000 + (873*cos(t1)*cos(t5))/50000 - d6*(cos(t1)*cos(t5) - cos(t2 + t3 + t4)*sin(t1)*sin(t5)) - d4*cos(t1) - (873*cos(t2 + t3 + t4)*sin(t1)*sin(t5))/50000 + (19*sin(t2 + t3 + t4)*cos(t6)*sin(t1))/20000 + a3*cos(t2 + t3)*sin(t1) + a2*cos(t2)*sin(t1) - d5*sin(t2 + t3 + t4)*sin(t1)))/2 - (((19*cos(t6)*(cos(t1)*sin(t5) + cos(t2 + t3 + t4)*cos(t5)*sin(t1)))/20000 - (19*sin(t2 + t3 + t4)*sin(t1)*sin(t6))/20000)*((817*sin(t6)*(cos(t1)*sin(t5) + cos(t2 + t3 + t4)*cos(t5)*sin(t1)))/2000000 + (37539*cos(t1)*cos(t5))/5000000 - (43*d6*(cos(t1)*cos(t5) - cos(t2 + t3 + t4)*sin(t1)*sin(t5)))/100 - (43*d4*cos(t1))/100 - (37539*cos(t2 + t3 + t4)*sin(t1)*sin(t5))/5000000 + (817*sin(t2 + t3 + t4)*cos(t6)*sin(t1))/2000000 + (43*a3*cos(t2 + t3)*sin(t1))/100 + (43*a2*cos(t2)*sin(t1))/100 - (43*d5*sin(t2 + t3 + t4)*sin(t1))/100))/2) - td3*((713241*sin(t2 + t3 + t4 + t5 - t6))/800000000000 - (713241*sin(t2 + t3 + t4 + t5 + t6))/800000000000 - (713241*sin(t2 + t3 + t4 - t5 + t6))/800000000000 - (784477*sin(t2 + t3 + t4 + t5 - 2*t6))/320000000000 - (784477*sin(t2 + t3 + t4 + t5 + 2*t6))/320000000000 - (713241*sin(t2 + t3 + t4 - 2*t5 + t6))/800000000000 - (713241*sin(t2 + t3 + t4 + 2*t5 + t6))/800000000000 + (713241*sin(t2 + t3 + t4 - t5 - t6))/800000000000 + (784477*sin(t2 + t3 + t4 - t5 - 2*t6))/320000000000 + (784477*sin(t2 + t3 + t4 - t5 + 2*t6))/320000000000 - (713241*sin(t2 + t3 + t4 - 2*t5 - t6))/800000000000 - (713241*sin(t2 + t3 + t4 + 2*t5 - t6))/800000000000 - (784477*sin(t2 + t3 + t4 - 2*t5 - 2*t6))/640000000000 + (784477*sin(t2 + t3 + t4 - 2*t5 + 2*t6))/640000000000 + (784477*sin(t2 + t3 + t4 + 2*t5 - 2*t6))/640000000000 - (784477*sin(t2 + t3 + t4 + 2*t5 + 2*t6))/640000000000 - (817*a3*cos(t2 + t3 - t5 - t6))/16000000 + (817*d4*sin(t2 + t3 + t4 + t5 - t6))/16000000 + (817*d4*sin(t2 + t3 + t4 - t5 + t6))/16000000 - (817*d5*sin(t2 + t3 + t4 + t5 - t6))/16000000 + (817*d5*sin(t2 + t3 + t4 - t5 + t6))/16000000 - (817*d6*sin(t2 + t3 + t4 + t5 - t6))/16000000 + (817*d6*sin(t2 + t3 + t4 - t5 + t6))/16000000 + (817*d6*sin(t2 + t3 + t4 - 2*t5 + t6))/16000000 + (817*d6*sin(t2 + t3 + t4 + 2*t5 + t6))/16000000 + (817*a3*cos(t2 + t3 + t5 + t6))/16000000 + (817*d4*sin(t2 + t3 + t4 + t6))/8000000 + (817*d4*sin(t2 + t3 + t4 - t5 - t6))/16000000 + (817*d5*sin(t2 + t3 + t4 - t5 - t6))/16000000 - (817*d6*sin(t2 + t3 + t4 - t5 - t6))/16000000 + (817*d6*sin(t2 + t3 + t4 - 2*t5 - t6))/16000000 + (817*d6*sin(t2 + t3 + t4 + 2*t5 - t6))/16000000 + (817*a3*cos(t2 + t3 + t5 - t6))/16000000 - (817*a3*cos(t2 + t3 - t5 + t6))/16000000 - (817*d4*sin(t2 + t3 + t4 - t6))/8000000 + (817*d4*sin(t2 + t3 + t4 + t5 + t6))/16000000 - (817*d5*sin(t2 + t3 + t4 + t5 + t6))/16000000 + (817*d6*sin(t2 + t3 + t4 + t5 + t6))/16000000 - (16015523*cos(t2)*cos(t3)*cos(t4)*sin(t5))/80000000000 - (713241*cos(t2)*cos(t3)*cos(t6)*sin(t4))/200000000000 - (713241*cos(t2)*cos(t4)*cos(t6)*sin(t3))/200000000000 - (713241*cos(t3)*cos(t4)*cos(t6)*sin(t2))/200000000000 + (16015523*cos(t2)*sin(t3)*sin(t4)*sin(t5))/80000000000 + (16015523*cos(t3)*sin(t2)*sin(t4)*sin(t5))/80000000000 + (16015523*cos(t4)*sin(t2)*sin(t3)*sin(t5))/80000000000 + (713241*cos(t6)*sin(t2)*sin(t3)*sin(t4))/200000000000 + (817*d4*cos(t2)*cos(t3)*cos(t4)*sin(t6))/4000000 + (817*d6*cos(t2)*cos(t3)*cos(t6)*sin(t4))/4000000 + (817*d6*cos(t2)*cos(t4)*cos(t6)*sin(t3))/4000000 + (817*d6*cos(t3)*cos(t4)*cos(t6)*sin(t2))/4000000 + (817*a3*cos(t2)*cos(t6)*sin(t3)*sin(t5))/4000000 + (817*a3*cos(t3)*cos(t6)*sin(t2)*sin(t5))/4000000 - (817*d4*cos(t2)*sin(t3)*sin(t4)*sin(t6))/4000000 - (817*d4*cos(t3)*sin(t2)*sin(t4)*sin(t6))/4000000 - (817*d4*cos(t4)*sin(t2)*sin(t3)*sin(t6))/4000000 - (817*d6*cos(t6)*sin(t2)*sin(t3)*sin(t4))/4000000 - (713241*cos(t2)*cos(t3)*cos(t4)*cos(t5)*sin(t6))/200000000000 + (713241*cos(t2)*cos(t5)*sin(t3)*sin(t4)*sin(t6))/200000000000 + (713241*cos(t3)*cos(t5)*sin(t2)*sin(t4)*sin(t6))/200000000000 + (713241*cos(t4)*cos(t5)*sin(t2)*sin(t3)*sin(t6))/200000000000 + (817*d4*cos(t2)*cos(t3)*cos(t5)*cos(t6)*sin(t4))/4000000 + (817*d4*cos(t2)*cos(t4)*cos(t5)*cos(t6)*sin(t3))/4000000 + (817*d4*cos(t3)*cos(t4)*cos(t5)*cos(t6)*sin(t2))/4000000 + (817*d5*cos(t2)*cos(t3)*cos(t4)*cos(t6)*sin(t5))/4000000 + (817*d6*cos(t2)*cos(t3)*cos(t4)*cos(t5)*sin(t6))/4000000 - (817*d4*cos(t5)*cos(t6)*sin(t2)*sin(t3)*sin(t4))/4000000 - (817*d5*cos(t2)*cos(t6)*sin(t3)*sin(t4)*sin(t5))/4000000 - (817*d5*cos(t3)*cos(t6)*sin(t2)*sin(t4)*sin(t5))/4000000 - (817*d5*cos(t4)*cos(t6)*sin(t2)*sin(t3)*sin(t5))/4000000 - (817*d6*cos(t2)*cos(t5)*sin(t3)*sin(t4)*sin(t6))/4000000 - (817*d6*cos(t3)*cos(t5)*sin(t2)*sin(t4)*sin(t6))/4000000 - (817*d6*cos(t4)*cos(t5)*sin(t2)*sin(t3)*sin(t6))/4000000) - td2*((713241*sin(t2 + t3 + t4 + t5 - t6))/800000000000 - (713241*sin(t2 + t3 + t4 + t5 + t6))/800000000000 - (713241*sin(t2 + t3 + t4 - t5 + t6))/800000000000 - (784477*sin(t2 + t3 + t4 + t5 - 2*t6))/320000000000 - (784477*sin(t2 + t3 + t4 + t5 + 2*t6))/320000000000 - (713241*sin(t2 + t3 + t4 - 2*t5 + t6))/800000000000 - (713241*sin(t2 + t3 + t4 + 2*t5 + t6))/800000000000 + (713241*sin(t2 + t3 + t4 - t5 - t6))/800000000000 + (784477*sin(t2 + t3 + t4 - t5 - 2*t6))/320000000000 + (784477*sin(t2 + t3 + t4 - t5 + 2*t6))/320000000000 - (713241*sin(t2 + t3 + t4 - 2*t5 - t6))/800000000000 - (713241*sin(t2 + t3 + t4 + 2*t5 - t6))/800000000000 - (784477*sin(t2 + t3 + t4 - 2*t5 - 2*t6))/640000000000 + (784477*sin(t2 + t3 + t4 - 2*t5 + 2*t6))/640000000000 + (784477*sin(t2 + t3 + t4 + 2*t5 - 2*t6))/640000000000 - (784477*sin(t2 + t3 + t4 + 2*t5 + 2*t6))/640000000000 - (817*a3*cos(t2 + t3 - t5 - t6))/16000000 + (817*d4*sin(t2 + t3 + t4 + t5 - t6))/16000000 + (817*d4*sin(t2 + t3 + t4 - t5 + t6))/16000000 - (817*d5*sin(t2 + t3 + t4 + t5 - t6))/16000000 + (817*d5*sin(t2 + t3 + t4 - t5 + t6))/16000000 - (817*d6*sin(t2 + t3 + t4 + t5 - t6))/16000000 + (817*d6*sin(t2 + t3 + t4 - t5 + t6))/16000000 + (817*d6*sin(t2 + t3 + t4 - 2*t5 + t6))/16000000 + (817*d6*sin(t2 + t3 + t4 + 2*t5 + t6))/16000000 + (817*a2*cos(t2 + t5 - t6))/16000000 - (817*a2*cos(t2 - t5 + t6))/16000000 - (817*a2*cos(t5 - t2 + t6))/16000000 + (817*a3*cos(t2 + t3 + t5 + t6))/16000000 + (817*d4*sin(t2 + t3 + t4 + t6))/8000000 + (817*d4*sin(t2 + t3 + t4 - t5 - t6))/16000000 + (817*d5*sin(t2 + t3 + t4 - t5 - t6))/16000000 - (817*d6*sin(t2 + t3 + t4 - t5 - t6))/16000000 + (817*d6*sin(t2 + t3 + t4 - 2*t5 - t6))/16000000 + (817*d6*sin(t2 + t3 + t4 + 2*t5 - t6))/16000000 + (817*a3*cos(t2 + t3 + t5 - t6))/16000000 - (817*a3*cos(t2 + t3 - t5 + t6))/16000000 - (817*d4*sin(t2 + t3 + t4 - t6))/8000000 + (817*d4*sin(t2 + t3 + t4 + t5 + t6))/16000000 - (817*d5*sin(t2 + t3 + t4 + t5 + t6))/16000000 + (817*d6*sin(t2 + t3 + t4 + t5 + t6))/16000000 + (817*a2*cos(t2 + t5 + t6))/16000000 + (817*a2*cos(t6)*sin(t2)*sin(t5))/4000000 - (16015523*cos(t2)*cos(t3)*cos(t4)*sin(t5))/80000000000 - (713241*cos(t2)*cos(t3)*cos(t6)*sin(t4))/200000000000 - (713241*cos(t2)*cos(t4)*cos(t6)*sin(t3))/200000000000 - (713241*cos(t3)*cos(t4)*cos(t6)*sin(t2))/200000000000 + (16015523*cos(t2)*sin(t3)*sin(t4)*sin(t5))/80000000000 + (16015523*cos(t3)*sin(t2)*sin(t4)*sin(t5))/80000000000 + (16015523*cos(t4)*sin(t2)*sin(t3)*sin(t5))/80000000000 + (713241*cos(t6)*sin(t2)*sin(t3)*sin(t4))/200000000000 + (817*d4*cos(t2)*cos(t3)*cos(t4)*sin(t6))/4000000 + (817*d6*cos(t2)*cos(t3)*cos(t6)*sin(t4))/4000000 + (817*d6*cos(t2)*cos(t4)*cos(t6)*sin(t3))/4000000 + (817*d6*cos(t3)*cos(t4)*cos(t6)*sin(t2))/4000000 + (817*a3*cos(t2)*cos(t6)*sin(t3)*sin(t5))/4000000 + (817*a3*cos(t3)*cos(t6)*sin(t2)*sin(t5))/4000000 - (817*d4*cos(t2)*sin(t3)*sin(t4)*sin(t6))/4000000 - (817*d4*cos(t3)*sin(t2)*sin(t4)*sin(t6))/4000000 - (817*d4*cos(t4)*sin(t2)*sin(t3)*sin(t6))/4000000 - (817*d6*cos(t6)*sin(t2)*sin(t3)*sin(t4))/4000000 - (713241*cos(t2)*cos(t3)*cos(t4)*cos(t5)*sin(t6))/200000000000 + (713241*cos(t2)*cos(t5)*sin(t3)*sin(t4)*sin(t6))/200000000000 + (713241*cos(t3)*cos(t5)*sin(t2)*sin(t4)*sin(t6))/200000000000 + (713241*cos(t4)*cos(t5)*sin(t2)*sin(t3)*sin(t6))/200000000000 + (817*d4*cos(t2)*cos(t3)*cos(t5)*cos(t6)*sin(t4))/4000000 + (817*d4*cos(t2)*cos(t4)*cos(t5)*cos(t6)*sin(t3))/4000000 + (817*d4*cos(t3)*cos(t4)*cos(t5)*cos(t6)*sin(t2))/4000000 + (817*d5*cos(t2)*cos(t3)*cos(t4)*cos(t6)*sin(t5))/4000000 + (817*d6*cos(t2)*cos(t3)*cos(t4)*cos(t5)*sin(t6))/4000000 - (817*d4*cos(t5)*cos(t6)*sin(t2)*sin(t3)*sin(t4))/4000000 - (817*d5*cos(t2)*cos(t6)*sin(t3)*sin(t4)*sin(t5))/4000000 - (817*d5*cos(t3)*cos(t6)*sin(t2)*sin(t4)*sin(t5))/4000000 - (817*d5*cos(t4)*cos(t6)*sin(t2)*sin(t3)*sin(t5))/4000000 - (817*d6*cos(t2)*cos(t5)*sin(t3)*sin(t4)*sin(t6))/4000000 - (817*d6*cos(t3)*cos(t5)*sin(t2)*sin(t4)*sin(t6))/4000000 - (817*d6*cos(t4)*cos(t5)*sin(t2)*sin(t3)*sin(t6))/4000000);

c21=td1*((49450651*sin(2*t2 + 2*t3 + 2*t4 - t5))/250000000000 - (1966511423*sin(2*t2 + 2*t3 + 2*t4 - 2*t5))/20000000000000 - (1966511423*sin(2*t2 + 2*t3 + 2*t4 + 2*t5))/20000000000000 + (53*sin(2*t2))/40 - (3534581023*sin(2*t2 + 2*t3 + 2*t4))/10000000000000 + (42783*sin(2*t2 + 2*t3))/62500 - (49450651*sin(2*t2 + 2*t3 + 2*t4 + t5))/250000000000 + (37373*d5*sin(2*t2 + 2*t3 + 2*t4))/2500000 + (957929*a2*cos(2*t2 + t3 + t4 - t5))/100000000 - (957929*a3*cos(2*t2 + 2*t3 + t4 + t5))/100000000 + (((43*a3*sin(t2 + t3)*cos(t1))/100 - (37539*sin(t2 + t3 + t4)*cos(t1)*sin(t5))/5000000 - (817*cos(t2 + t3 + t4)*cos(t1)*cos(t6))/2000000 + (43*a2*cos(t1)*sin(t2))/100 + (43*d5*cos(t2 + t3 + t4)*cos(t1))/100 + (817*sin(t2 + t3 + t4)*cos(t1)*cos(t5)*sin(t6))/2000000 + (43*d6*sin(t2 + t3 + t4)*cos(t1)*sin(t5))/100)*(d6*(cos(t5)*sin(t1) + cos(t2 + t3 + t4)*cos(t1)*sin(t5)) - (873*cos(t5)*sin(t1))/50000 - (19*sin(t6)*(sin(t1)*sin(t5) - cos(t2 + t3 + t4)*cos(t1)*cos(t5)))/20000 + d4*sin(t1) - (873*cos(t2 + t3 + t4)*cos(t1)*sin(t5))/50000 + (19*sin(t2 + t3 + t4)*cos(t1)*cos(t6))/20000 + a3*cos(t2 + t3)*cos(t1) + a2*cos(t1)*cos(t2) - d5*sin(t2 + t3 + t4)*cos(t1)))/2 + ((a3*sin(t2 + t3)*cos(t1) - (873*sin(t2 + t3 + t4)*cos(t1)*sin(t5))/50000 - (19*cos(t2 + t3 + t4)*cos(t1)*cos(t6))/20000 + a2*cos(t1)*sin(t2) + d5*cos(t2 + t3 + t4)*cos(t1) + (19*sin(t2 + t3 + t4)*cos(t1)*cos(t5)*sin(t6))/20000 + d6*sin(t2 + t3 + t4)*cos(t1)*sin(t5))*((43*d6*(cos(t5)*sin(t1) + cos(t2 + t3 + t4)*cos(t1)*sin(t5)))/100 - (37539*cos(t5)*sin(t1))/5000000 - (817*sin(t6)*(sin(t1)*sin(t5) - cos(t2 + t3 + t4)*cos(t1)*cos(t5)))/2000000 + (43*d4*sin(t1))/100 - (37539*cos(t2 + t3 + t4)*cos(t1)*sin(t5))/5000000 + (817*sin(t2 + t3 + t4)*cos(t1)*cos(t6))/2000000 + (43*a3*cos(t2 + t3)*cos(t1))/100 + (43*a2*cos(t1)*cos(t2))/100 - (43*d5*sin(t2 + t3 + t4)*cos(t1))/100))/2 + (210469*a2*cos(2*t2 + t3 + t4))/50000000 + ((sin(t2 + t3 + t4)*cos(t6) + cos(t2 + t3 + t4)*cos(t5)*sin(t6))*((3*cos(t2 + t3 + t4)*cos(t6))/12500 - (3*sin(t2 + t3 + t4)*cos(t5)*sin(t6))/12500))/2 + ((cos(t2 + t3 + t4)*cos(t6) - sin(t2 + t3 + t4)*cos(t5)*sin(t6))*((3*sin(t2 + t3 + t4)*cos(t6))/12500 + (3*cos(t2 + t3 + t4)*cos(t5)*sin(t6))/12500))/2 + ((cos(t2 + t3 + t4)*sin(t6) + sin(t2 + t3 + t4)*cos(t5)*cos(t6))*((11*sin(t2 + t3 + t4)*sin(t6))/50000 - (11*cos(t2 + t3 + t4)*cos(t5)*cos(t6))/50000))/2 + ((sin(t2 + t3 + t4)*sin(t6) - cos(t2 + t3 + t4)*cos(t5)*cos(t6))*((11*cos(t2 + t3 + t4)*sin(t6))/50000 + (11*sin(t2 + t3 + t4)*cos(t5)*cos(t6))/50000))/2 + (8247*a2^2*sin(2*t2))/1000 - (1967*d5^2*sin(2*t2 + 2*t3 + 2*t4))/2000 + (957929*a3*cos(2*t2 + 2*t3 + t4 - t5))/100000000 + (957929*d5*sin(2*t2 + 2*t3 + 2*t4 + t5))/100000000 + (1967*a3^2*sin(2*t2 + 2*t3))/1000 + (210469*a3*cos(2*t2 + 2*t3 + t4))/50000000 - (957929*a2*cos(2*t2 + t3 + t4 + t5))/100000000 + (((43*a3*sin(t2 + t3)*sin(t1))/100 - (37539*sin(t2 + t3 + t4)*sin(t1)*sin(t5))/5000000 - (817*cos(t2 + t3 + t4)*cos(t6)*sin(t1))/2000000 + (43*a2*sin(t1)*sin(t2))/100 + (43*d5*cos(t2 + t3 + t4)*sin(t1))/100 + (817*sin(t2 + t3 + t4)*cos(t5)*sin(t1)*sin(t6))/2000000 + (43*d6*sin(t2 + t3 + t4)*sin(t1)*sin(t5))/100)*((19*sin(t6)*(cos(t1)*sin(t5) + cos(t2 + t3 + t4)*cos(t5)*sin(t1)))/20000 + (873*cos(t1)*cos(t5))/50000 - d6*(cos(t1)*cos(t5) - cos(t2 + t3 + t4)*sin(t1)*sin(t5)) - d4*cos(t1) - (873*cos(t2 + t3 + t4)*sin(t1)*sin(t5))/50000 + (19*sin(t2 + t3 + t4)*cos(t6)*sin(t1))/20000 + a3*cos(t2 + t3)*sin(t1) + a2*cos(t2)*sin(t1) - d5*sin(t2 + t3 + t4)*sin(t1)))/2 + ((a3*sin(t2 + t3)*sin(t1) - (873*sin(t2 + t3 + t4)*sin(t1)*sin(t5))/50000 - (19*cos(t2 + t3 + t4)*cos(t6)*sin(t1))/20000 + a2*sin(t1)*sin(t2) + d5*cos(t2 + t3 + t4)*sin(t1) + (19*sin(t2 + t3 + t4)*cos(t5)*sin(t1)*sin(t6))/20000 + d6*sin(t2 + t3 + t4)*sin(t1)*sin(t5))*((817*sin(t6)*(cos(t1)*sin(t5) + cos(t2 + t3 + t4)*cos(t5)*sin(t1)))/2000000 + (37539*cos(t1)*cos(t5))/5000000 - (43*d6*(cos(t1)*cos(t5) - cos(t2 + t3 + t4)*sin(t1)*sin(t5)))/100 - (43*d4*cos(t1))/100 - (37539*cos(t2 + t3 + t4)*sin(t1)*sin(t5))/5000000 + (817*sin(t2 + t3 + t4)*cos(t6)*sin(t1))/2000000 + (43*a3*cos(t2 + t3)*sin(t1))/100 + (43*a2*cos(t2)*sin(t1))/100 - (43*d5*sin(t2 + t3 + t4)*sin(t1))/100))/2 + (2041*a2*sin(2*t2 + t3))/625 - (957929*d5*sin(2*t2 + 2*t3 + 2*t4 - t5))/100000000 + (1967*a3*d5*cos(2*t2 + 2*t3 + t4))/1000 + (1967*a2*a3*sin(2*t2 + t3))/500 + (1967*a2*d5*cos(2*t2 + t3 + t4))/1000 - (cos(t2 + t3 + t4)*sin(t2 + t3 + t4)*sin(t5)^2)/2500) + td5*((49450651*sin(t2 + t3 + t4 - t5))/250000000000 - (7474967197*sin(t2 + t3 + t4 - 2*t5))/40000000000000 - (7474967197*sin(t2 + t3 + t4 + 2*t5))/40000000000000 + (784477*sin(t2 + t3 + t4 - 2*t6))/320000000000 + (784477*sin(t2 + t3 + t4 + 2*t6))/320000000000 + (713241*sin(t2 + t3 + t4 + t5 + t6))/400000000000 + (33478847947*sin(t2 + t3 + t4))/20000000000000 + (713241*sin(t2 + t3 + t4 + t5 - t6))/400000000000 - (713241*sin(t2 + t3 + t4 - t5 + t6))/400000000000 - (784477*sin(t2 + t3 + t4 + t5 - 2*t6))/320000000000 + (784477*sin(t2 + t3 + t4 + t5 + 2*t6))/320000000000 - (713241*sin(t2 + t3 + t4 - 2*t5 + t6))/400000000000 + (713241*sin(t2 + t3 + t4 + 2*t5 + t6))/400000000000 - (49450651*sin(t2 + t3 + t4 + t5))/250000000000 - (713241*sin(t2 + t3 + t4 - t5 - t6))/400000000000 - (784477*sin(t2 + t3 + t4 - t5 - 2*t6))/320000000000 + (784477*sin(t2 + t3 + t4 - t5 + 2*t6))/320000000000 + (713241*sin(t2 + t3 + t4 - 2*t5 - t6))/400000000000 - (713241*sin(t2 + t3 + t4 + 2*t5 - t6))/400000000000 + (784477*sin(t2 + t3 + t4 - 2*t5 - 2*t6))/640000000000 + (784477*sin(t2 + t3 + t4 - 2*t5 + 2*t6))/640000000000 + (784477*sin(t2 + t3 + t4 + 2*t5 - 2*t6))/640000000000 + (784477*sin(t2 + t3 + t4 + 2*t5 + 2*t6))/640000000000 + (817*a3*cos(t2 + t3 - t5 - t6))/8000000 - (43*d6^2*sin(t2 + t3 + t4 - 2*t5))/400 - (43*d6^2*sin(t2 + t3 + t4 + 2*t5))/400 - (817*d5*sin(t2 + t3 + t4 + t5 - t6))/8000000 + (817*d5*sin(t2 + t3 + t4 - t5 + t6))/8000000 - (817*d6*sin(t2 + t3 + t4 + t5 - t6))/8000000 + (817*d6*sin(t2 + t3 + t4 - t5 + t6))/8000000 + (817*d6*sin(t2 + t3 + t4 - 2*t5 + t6))/8000000 - (817*d6*sin(t2 + t3 + t4 + 2*t5 + t6))/8000000 + (582539*a3*cos(t2 + t3 - t5))/100000000 + (817*a2*cos(t2 + t5 - t6))/8000000 - (817*a2*cos(t2 - t5 + t6))/8000000 + (817*a2*cos(t5 - t2 + t6))/8000000 + (43*d6^2*sin(t2 + t3 + t4))/200 - (817*a3*cos(t2 + t3 + t5 + t6))/8000000 + (582539*d5*sin(t2 + t3 + t4 + t5))/100000000 - (582539*a2*cos(t2 + t5))/100000000 - (817*d5*sin(t2 + t3 + t4 - t5 - t6))/8000000 + (817*d6*sin(t2 + t3 + t4 - t5 - t6))/8000000 - (817*d6*sin(t2 + t3 + t4 - 2*t5 - t6))/8000000 + (817*d6*sin(t2 + t3 + t4 + 2*t5 - t6))/8000000 + (817*a3*cos(t2 + t3 + t5 - t6))/8000000 - (817*a3*cos(t2 + t3 - t5 + t6))/8000000 - (582539*d5*sin(t2 + t3 + t4 - t5))/100000000 + (37539*d6*sin(t2 + t3 + t4 - 2*t5))/10000000 + (37539*d6*sin(t2 + t3 + t4 + 2*t5))/10000000 + (582539*a2*cos(t2 - t5))/100000000 + (817*d5*sin(t2 + t3 + t4 + t5 + t6))/8000000 - (817*d6*sin(t2 + t3 + t4 + t5 + t6))/8000000 - (582539*a3*cos(t2 + t3 + t5))/100000000 - (817*a2*cos(t2 + t5 + t6))/8000000 - (37539*d6*sin(t2 + t3 + t4))/5000000 - (43*d5*d6*sin(t2 + t3 + t4 - t5))/200 + (43*a2*d6*cos(t2 - t5))/200 - (43*a3*d6*cos(t2 + t3 + t5))/200 + (43*a3*d6*cos(t2 + t3 - t5))/200 + (43*d5*d6*sin(t2 + t3 + t4 + t5))/200 - (43*a2*d6*cos(t2 + t5))/200) - td6*((713241*sin(t2 + t3 + t4 + t5 - t6))/800000000000 - (713241*sin(t2 + t3 + t4 + t5 + t6))/800000000000 - (713241*sin(t2 + t3 + t4 - t5 + t6))/800000000000 - (784477*sin(t2 + t3 + t4 + t5 - 2*t6))/320000000000 - (784477*sin(t2 + t3 + t4 + t5 + 2*t6))/320000000000 - (713241*sin(t2 + t3 + t4 - 2*t5 + t6))/800000000000 - (713241*sin(t2 + t3 + t4 + 2*t5 + t6))/800000000000 + (713241*sin(t2 + t3 + t4 - t5 - t6))/800000000000 + (784477*sin(t2 + t3 + t4 - t5 - 2*t6))/320000000000 + (784477*sin(t2 + t3 + t4 - t5 + 2*t6))/320000000000 - (713241*sin(t2 + t3 + t4 - 2*t5 - t6))/800000000000 - (713241*sin(t2 + t3 + t4 + 2*t5 - t6))/800000000000 - (784477*sin(t2 + t3 + t4 - 2*t5 - 2*t6))/640000000000 + (784477*sin(t2 + t3 + t4 - 2*t5 + 2*t6))/640000000000 + (784477*sin(t2 + t3 + t4 + 2*t5 - 2*t6))/640000000000 - (784477*sin(t2 + t3 + t4 + 2*t5 + 2*t6))/640000000000 - (817*a3*cos(t2 + t3 - t5 - t6))/16000000 + (817*d4*sin(t2 + t3 + t4 + t5 - t6))/16000000 + (817*d4*sin(t2 + t3 + t4 - t5 + t6))/16000000 - (817*d5*sin(t2 + t3 + t4 + t5 - t6))/16000000 + (817*d5*sin(t2 + t3 + t4 - t5 + t6))/16000000 - (817*d6*sin(t2 + t3 + t4 + t5 - t6))/16000000 + (817*d6*sin(t2 + t3 + t4 - t5 + t6))/16000000 + (817*d6*sin(t2 + t3 + t4 - 2*t5 + t6))/16000000 + (817*d6*sin(t2 + t3 + t4 + 2*t5 + t6))/16000000 + (817*a2*cos(t2 + t5 - t6))/16000000 - (817*a2*cos(t2 - t5 + t6))/16000000 - (817*a2*cos(t5 - t2 + t6))/16000000 + (817*a3*cos(t2 + t3 + t5 + t6))/16000000 + (817*d4*sin(t2 + t3 + t4 + t6))/8000000 + (817*d4*sin(t2 + t3 + t4 - t5 - t6))/16000000 + (817*d5*sin(t2 + t3 + t4 - t5 - t6))/16000000 - (817*d6*sin(t2 + t3 + t4 - t5 - t6))/16000000 + (817*d6*sin(t2 + t3 + t4 - 2*t5 - t6))/16000000 + (817*d6*sin(t2 + t3 + t4 + 2*t5 - t6))/16000000 + (817*a3*cos(t2 + t3 + t5 - t6))/16000000 - (817*a3*cos(t2 + t3 - t5 + t6))/16000000 - (817*d4*sin(t2 + t3 + t4 - t6))/8000000 + (817*d4*sin(t2 + t3 + t4 + t5 + t6))/16000000 - (817*d5*sin(t2 + t3 + t4 + t5 + t6))/16000000 + (817*d6*sin(t2 + t3 + t4 + t5 + t6))/16000000 + (817*a2*cos(t2 + t5 + t6))/16000000 - (817*a2*cos(t6)*sin(t2)*sin(t5))/4000000 + (16015523*cos(t2)*cos(t3)*cos(t4)*sin(t5))/80000000000 + (713241*cos(t2)*cos(t3)*cos(t6)*sin(t4))/200000000000 + (713241*cos(t2)*cos(t4)*cos(t6)*sin(t3))/200000000000 + (713241*cos(t3)*cos(t4)*cos(t6)*sin(t2))/200000000000 - (16015523*cos(t2)*sin(t3)*sin(t4)*sin(t5))/80000000000 - (16015523*cos(t3)*sin(t2)*sin(t4)*sin(t5))/80000000000 - (16015523*cos(t4)*sin(t2)*sin(t3)*sin(t5))/80000000000 - (713241*cos(t6)*sin(t2)*sin(t3)*sin(t4))/200000000000 - (817*d4*cos(t2)*cos(t3)*cos(t4)*sin(t6))/4000000 - (817*d6*cos(t2)*cos(t3)*cos(t6)*sin(t4))/4000000 - (817*d6*cos(t2)*cos(t4)*cos(t6)*sin(t3))/4000000 - (817*d6*cos(t3)*cos(t4)*cos(t6)*sin(t2))/4000000 - (817*a3*cos(t2)*cos(t6)*sin(t3)*sin(t5))/4000000 - (817*a3*cos(t3)*cos(t6)*sin(t2)*sin(t5))/4000000 + (817*d4*cos(t2)*sin(t3)*sin(t4)*sin(t6))/4000000 + (817*d4*cos(t3)*sin(t2)*sin(t4)*sin(t6))/4000000 + (817*d4*cos(t4)*sin(t2)*sin(t3)*sin(t6))/4000000 + (817*d6*cos(t6)*sin(t2)*sin(t3)*sin(t4))/4000000 + (713241*cos(t2)*cos(t3)*cos(t4)*cos(t5)*sin(t6))/200000000000 - (713241*cos(t2)*cos(t5)*sin(t3)*sin(t4)*sin(t6))/200000000000 - (713241*cos(t3)*cos(t5)*sin(t2)*sin(t4)*sin(t6))/200000000000 - (713241*cos(t4)*cos(t5)*sin(t2)*sin(t3)*sin(t6))/200000000000 - (817*d4*cos(t2)*cos(t3)*cos(t5)*cos(t6)*sin(t4))/4000000 - (817*d4*cos(t2)*cos(t4)*cos(t5)*cos(t6)*sin(t3))/4000000 - (817*d4*cos(t3)*cos(t4)*cos(t5)*cos(t6)*sin(t2))/4000000 - (817*d5*cos(t2)*cos(t3)*cos(t4)*cos(t6)*sin(t5))/4000000 - (817*d6*cos(t2)*cos(t3)*cos(t4)*cos(t5)*sin(t6))/4000000 + (817*d4*cos(t5)*cos(t6)*sin(t2)*sin(t3)*sin(t4))/4000000 + (817*d5*cos(t2)*cos(t6)*sin(t3)*sin(t4)*sin(t5))/4000000 + (817*d5*cos(t3)*cos(t6)*sin(t2)*sin(t4)*sin(t5))/4000000 + (817*d5*cos(t4)*cos(t6)*sin(t2)*sin(t3)*sin(t5))/4000000 + (817*d6*cos(t2)*cos(t5)*sin(t3)*sin(t4)*sin(t6))/4000000 + (817*d6*cos(t3)*cos(t5)*sin(t2)*sin(t4)*sin(t6))/4000000 + (817*d6*cos(t4)*cos(t5)*sin(t2)*sin(t3)*sin(t6))/4000000);

c22=td5*((3786513411*cos(t5)*sin(t5))/5000000000000 - (713241*cos(t5)^2*sin(t6))/100000000000 + (713241*sin(t5)^2*sin(t6))/100000000000 - (784477*cos(t5)*cos(t6)^2*sin(t5))/40000000000 + (582539*a3*cos(t4)*cos(t5))/50000000 - (37539*d6*cos(t5)*sin(t5))/2500000 + (43*d6^2*cos(t5)*sin(t5))/100 + (817*d6*cos(t5)^2*sin(t6))/2000000 - (817*d6*sin(t5)^2*sin(t6))/2000000 + (582539*a2*cos(t3)*cos(t4)*cos(t5))/50000000 - (582539*a2*cos(t5)*sin(t3)*sin(t4))/50000000 - (817*a3*cos(t4)*sin(t5)*sin(t6))/2000000 + (43*a3*d6*cos(t4)*cos(t5))/100 - (817*a2*cos(t3)*cos(t4)*sin(t5)*sin(t6))/2000000 + (817*a2*sin(t3)*sin(t4)*sin(t5)*sin(t6))/2000000 + (43*a2*d6*cos(t3)*cos(t4)*cos(t5))/100 - (43*a2*d6*cos(t5)*sin(t3)*sin(t4))/100) - td3*((2041*a2*sin(t3))/625 + (1091*a2*a3*sin(t3))/250 + (210469*a2*cos(t3)*cos(t4))/50000000 - (210469*a2*sin(t3)*sin(t4))/50000000 - (817*a2*cos(t3)*cos(t4)*cos(t6))/2000000 + (582539*a2*cos(t3)*sin(t4)*sin(t5))/50000000 + (582539*a2*cos(t4)*sin(t3)*sin(t5))/50000000 + (817*a2*cos(t6)*sin(t3)*sin(t4))/2000000 + (2397*a2*d5*cos(t3)*cos(t4))/1000 - (2397*a2*d5*sin(t3)*sin(t4))/1000 + (817*a2*cos(t3)*cos(t5)*sin(t4)*sin(t6))/2000000 + (817*a2*cos(t4)*cos(t5)*sin(t3)*sin(t6))/2000000 + (43*a2*d6*cos(t3)*sin(t4)*sin(t5))/100 + (43*a2*d6*cos(t4)*sin(t3)*sin(t5))/100) - td4*((210469*a3*cos(t4))/50000000 + (210469*a2*cos(t3)*cos(t4))/50000000 - (817*a3*cos(t4)*cos(t6))/2000000 - (210469*a2*sin(t3)*sin(t4))/50000000 + (582539*a3*sin(t4)*sin(t5))/50000000 + (2397*a3*d5*cos(t4))/1000 - (817*a2*cos(t3)*cos(t4)*cos(t6))/2000000 + (582539*a2*cos(t3)*sin(t4)*sin(t5))/50000000 + (582539*a2*cos(t4)*sin(t3)*sin(t5))/50000000 + (817*a2*cos(t6)*sin(t3)*sin(t4))/2000000 + (817*a3*cos(t5)*sin(t4)*sin(t6))/2000000 + (2397*a2*d5*cos(t3)*cos(t4))/1000 - (2397*a2*d5*sin(t3)*sin(t4))/1000 + (43*a3*d6*sin(t4)*sin(t5))/100 + (817*a2*cos(t3)*cos(t5)*sin(t4)*sin(t6))/2000000 + (817*a2*cos(t4)*cos(t5)*sin(t3)*sin(t6))/2000000 + (43*a2*d6*cos(t3)*sin(t4)*sin(t5))/100 + (43*a2*d6*cos(t4)*sin(t3)*sin(t5))/100) - td6*((784477*cos(t5)^2*cos(t6)*sin(t6))/40000000000 - (817*d5*sin(t6))/2000000 - (784477*cos(t6)*sin(t6))/40000000000 + (817*a3*sin(t4)*sin(t6))/2000000 + (713241*cos(t5)*cos(t6)*sin(t5))/100000000000 - (817*a3*cos(t4)*cos(t5)*cos(t6))/2000000 - (817*d6*cos(t5)*cos(t6)*sin(t5))/2000000 + (817*a2*cos(t3)*sin(t4)*sin(t6))/2000000 + (817*a2*cos(t4)*sin(t3)*sin(t6))/2000000 - (817*a2*cos(t3)*cos(t4)*cos(t5)*cos(t6))/2000000 + (817*a2*cos(t5)*cos(t6)*sin(t3)*sin(t4))/2000000);

c23=td5*((3786513411*cos(t5)*sin(t5))/5000000000000 - (713241*cos(t5)^2*sin(t6))/100000000000 + (713241*sin(t5)^2*sin(t6))/100000000000 - (784477*cos(t5)*cos(t6)^2*sin(t5))/40000000000 + (582539*a3*cos(t4)*cos(t5))/50000000 - (37539*d6*cos(t5)*sin(t5))/2500000 + (43*d6^2*cos(t5)*sin(t5))/100 + (817*d6*cos(t5)^2*sin(t6))/2000000 - (817*d6*sin(t5)^2*sin(t6))/2000000 + (582539*a2*cos(t3)*cos(t4)*cos(t5))/50000000 - (582539*a2*cos(t5)*sin(t3)*sin(t4))/50000000 - (817*a3*cos(t4)*sin(t5)*sin(t6))/2000000 + (43*a3*d6*cos(t4)*cos(t5))/100 - (817*a2*cos(t3)*cos(t4)*sin(t5)*sin(t6))/2000000 + (817*a2*sin(t3)*sin(t4)*sin(t5)*sin(t6))/2000000 + (43*a2*d6*cos(t3)*cos(t4)*cos(t5))/100 - (43*a2*d6*cos(t5)*sin(t3)*sin(t4))/100) - td3*((2041*a2*sin(t3))/625 + (1091*a2*a3*sin(t3))/250 + (210469*a2*cos(t3)*cos(t4))/50000000 - (210469*a2*sin(t3)*sin(t4))/50000000 - (817*a2*cos(t3)*cos(t4)*cos(t6))/2000000 + (582539*a2*cos(t3)*sin(t4)*sin(t5))/50000000 + (582539*a2*cos(t4)*sin(t3)*sin(t5))/50000000 + (817*a2*cos(t6)*sin(t3)*sin(t4))/2000000 + (2397*a2*d5*cos(t3)*cos(t4))/1000 - (2397*a2*d5*sin(t3)*sin(t4))/1000 + (817*a2*cos(t3)*cos(t5)*sin(t4)*sin(t6))/2000000 + (817*a2*cos(t4)*cos(t5)*sin(t3)*sin(t6))/2000000 + (43*a2*d6*cos(t3)*sin(t4)*sin(t5))/100 + (43*a2*d6*cos(t4)*sin(t3)*sin(t5))/100) - td2*((2041*a2*sin(t3))/625 + (1091*a2*a3*sin(t3))/250 + (210469*a2*cos(t3)*cos(t4))/50000000 - (210469*a2*sin(t3)*sin(t4))/50000000 - (817*a2*cos(t3)*cos(t4)*cos(t6))/2000000 + (582539*a2*cos(t3)*sin(t4)*sin(t5))/50000000 + (582539*a2*cos(t4)*sin(t3)*sin(t5))/50000000 + (817*a2*cos(t6)*sin(t3)*sin(t4))/2000000 + (2397*a2*d5*cos(t3)*cos(t4))/1000 - (2397*a2*d5*sin(t3)*sin(t4))/1000 + (817*a2*cos(t3)*cos(t5)*sin(t4)*sin(t6))/2000000 + (817*a2*cos(t4)*cos(t5)*sin(t3)*sin(t6))/2000000 + (43*a2*d6*cos(t3)*sin(t4)*sin(t5))/100 + (43*a2*d6*cos(t4)*sin(t3)*sin(t5))/100) - td4*((210469*a3*cos(t4))/50000000 + (210469*a2*cos(t3)*cos(t4))/50000000 - (817*a3*cos(t4)*cos(t6))/2000000 - (210469*a2*sin(t3)*sin(t4))/50000000 + (582539*a3*sin(t4)*sin(t5))/50000000 + (2397*a3*d5*cos(t4))/1000 - (817*a2*cos(t3)*cos(t4)*cos(t6))/2000000 + (582539*a2*cos(t3)*sin(t4)*sin(t5))/50000000 + (582539*a2*cos(t4)*sin(t3)*sin(t5))/50000000 + (817*a2*cos(t6)*sin(t3)*sin(t4))/2000000 + (817*a3*cos(t5)*sin(t4)*sin(t6))/2000000 + (2397*a2*d5*cos(t3)*cos(t4))/1000 - (2397*a2*d5*sin(t3)*sin(t4))/1000 + (43*a3*d6*sin(t4)*sin(t5))/100 + (817*a2*cos(t3)*cos(t5)*sin(t4)*sin(t6))/2000000 + (817*a2*cos(t4)*cos(t5)*sin(t3)*sin(t6))/2000000 + (43*a2*d6*cos(t3)*sin(t4)*sin(t5))/100 + (43*a2*d6*cos(t4)*sin(t3)*sin(t5))/100) - td6*((784477*cos(t5)^2*cos(t6)*sin(t6))/40000000000 - (817*d5*sin(t6))/2000000 - (784477*cos(t6)*sin(t6))/40000000000 + (817*a3*sin(t4)*sin(t6))/2000000 + (713241*cos(t5)*cos(t6)*sin(t5))/100000000000 - (817*a3*cos(t4)*cos(t5)*cos(t6))/2000000 - (817*d6*cos(t5)*cos(t6)*sin(t5))/2000000 + (817*a2*cos(t3)*sin(t4)*sin(t6))/2000000 + (817*a2*cos(t4)*sin(t3)*sin(t6))/2000000 - (817*a2*cos(t3)*cos(t4)*cos(t5)*cos(t6))/2000000 + (817*a2*cos(t5)*cos(t6)*sin(t3)*sin(t4))/2000000);

c24=td5*((3786513411*cos(t5)*sin(t5))/5000000000000 - (713241*cos(t5)^2*sin(t6))/100000000000 + (713241*sin(t5)^2*sin(t6))/100000000000 - (784477*cos(t5)*cos(t6)^2*sin(t5))/40000000000 + (582539*a3*cos(t4)*cos(t5))/50000000 - (37539*d6*cos(t5)*sin(t5))/2500000 + (43*d6^2*cos(t5)*sin(t5))/100 + (817*d6*cos(t5)^2*sin(t6))/2000000 - (817*d6*sin(t5)^2*sin(t6))/2000000 + (582539*a2*cos(t3)*cos(t4)*cos(t5))/50000000 - (582539*a2*cos(t5)*sin(t3)*sin(t4))/50000000 - (817*a3*cos(t4)*sin(t5)*sin(t6))/2000000 + (43*a3*d6*cos(t4)*cos(t5))/100 - (817*a2*cos(t3)*cos(t4)*sin(t5)*sin(t6))/2000000 + (817*a2*sin(t3)*sin(t4)*sin(t5)*sin(t6))/2000000 + (43*a2*d6*cos(t3)*cos(t4)*cos(t5))/100 - (43*a2*d6*cos(t5)*sin(t3)*sin(t4))/100) - td2*((210469*a3*cos(t4))/50000000 + (210469*a2*cos(t3)*cos(t4))/50000000 - (817*a3*cos(t4)*cos(t6))/2000000 - (210469*a2*sin(t3)*sin(t4))/50000000 + (582539*a3*sin(t4)*sin(t5))/50000000 + (2397*a3*d5*cos(t4))/1000 - (817*a2*cos(t3)*cos(t4)*cos(t6))/2000000 + (582539*a2*cos(t3)*sin(t4)*sin(t5))/50000000 + (582539*a2*cos(t4)*sin(t3)*sin(t5))/50000000 + (817*a2*cos(t6)*sin(t3)*sin(t4))/2000000 + (817*a3*cos(t5)*sin(t4)*sin(t6))/2000000 + (2397*a2*d5*cos(t3)*cos(t4))/1000 - (2397*a2*d5*sin(t3)*sin(t4))/1000 + (43*a3*d6*sin(t4)*sin(t5))/100 + (817*a2*cos(t3)*cos(t5)*sin(t4)*sin(t6))/2000000 + (817*a2*cos(t4)*cos(t5)*sin(t3)*sin(t6))/2000000 + (43*a2*d6*cos(t3)*sin(t4)*sin(t5))/100 + (43*a2*d6*cos(t4)*sin(t3)*sin(t5))/100) - td3*((210469*a3*cos(t4))/50000000 + (210469*a2*cos(t3)*cos(t4))/50000000 - (817*a3*cos(t4)*cos(t6))/2000000 - (210469*a2*sin(t3)*sin(t4))/50000000 + (582539*a3*sin(t4)*sin(t5))/50000000 + (2397*a3*d5*cos(t4))/1000 - (817*a2*cos(t3)*cos(t4)*cos(t6))/2000000 + (582539*a2*cos(t3)*sin(t4)*sin(t5))/50000000 + (582539*a2*cos(t4)*sin(t3)*sin(t5))/50000000 + (817*a2*cos(t6)*sin(t3)*sin(t4))/2000000 + (817*a3*cos(t5)*sin(t4)*sin(t6))/2000000 + (2397*a2*d5*cos(t3)*cos(t4))/1000 - (2397*a2*d5*sin(t3)*sin(t4))/1000 + (43*a3*d6*sin(t4)*sin(t5))/100 + (817*a2*cos(t3)*cos(t5)*sin(t4)*sin(t6))/2000000 + (817*a2*cos(t4)*cos(t5)*sin(t3)*sin(t6))/2000000 + (43*a2*d6*cos(t3)*sin(t4)*sin(t5))/100 + (43*a2*d6*cos(t4)*sin(t3)*sin(t5))/100) - td4*((210469*a3*cos(t4))/50000000 + (210469*a2*cos(t3)*cos(t4))/50000000 - (817*a3*cos(t4)*cos(t6))/2000000 - (210469*a2*sin(t3)*sin(t4))/50000000 + (582539*a3*sin(t4)*sin(t5))/50000000 + (2397*a3*d5*cos(t4))/1000 - (817*a2*cos(t3)*cos(t4)*cos(t6))/2000000 + (582539*a2*cos(t3)*sin(t4)*sin(t5))/50000000 + (582539*a2*cos(t4)*sin(t3)*sin(t5))/50000000 + (817*a2*cos(t6)*sin(t3)*sin(t4))/2000000 + (817*a3*cos(t5)*sin(t4)*sin(t6))/2000000 + (2397*a2*d5*cos(t3)*cos(t4))/1000 - (2397*a2*d5*sin(t3)*sin(t4))/1000 + (43*a3*d6*sin(t4)*sin(t5))/100 + (817*a2*cos(t3)*cos(t5)*sin(t4)*sin(t6))/2000000 + (817*a2*cos(t4)*cos(t5)*sin(t3)*sin(t6))/2000000 + (43*a2*d6*cos(t3)*sin(t4)*sin(t5))/100 + (43*a2*d6*cos(t4)*sin(t3)*sin(t5))/100) - td6*((784477*cos(t5)^2*cos(t6)*sin(t6))/40000000000 - (817*d5*sin(t6))/2000000 - (784477*cos(t6)*sin(t6))/40000000000 + (817*a3*sin(t4)*sin(t6))/2000000 + (713241*cos(t5)*cos(t6)*sin(t5))/100000000000 - (817*a3*cos(t4)*cos(t5)*cos(t6))/2000000 - (817*d6*cos(t5)*cos(t6)*sin(t5))/2000000 + (817*a2*cos(t3)*sin(t4)*sin(t6))/2000000 + (817*a2*cos(t4)*sin(t3)*sin(t6))/2000000 - (817*a2*cos(t3)*cos(t4)*cos(t5)*cos(t6))/2000000 + (817*a2*cos(t5)*cos(t6)*sin(t3)*sin(t4))/2000000);

c25=td2*((3786513411*cos(t5)*sin(t5))/5000000000000 - (713241*cos(t5)^2*sin(t6))/100000000000 + (713241*sin(t5)^2*sin(t6))/100000000000 - (784477*cos(t5)*cos(t6)^2*sin(t5))/40000000000 + (582539*a3*cos(t4)*cos(t5))/50000000 - (37539*d6*cos(t5)*sin(t5))/2500000 + (43*d6^2*cos(t5)*sin(t5))/100 + (817*d6*cos(t5)^2*sin(t6))/2000000 - (817*d6*sin(t5)^2*sin(t6))/2000000 + (582539*a2*cos(t3)*cos(t4)*cos(t5))/50000000 - (582539*a2*cos(t5)*sin(t3)*sin(t4))/50000000 - (817*a3*cos(t4)*sin(t5)*sin(t6))/2000000 + (43*a3*d6*cos(t4)*cos(t5))/100 - (817*a2*cos(t3)*cos(t4)*sin(t5)*sin(t6))/2000000 + (817*a2*sin(t3)*sin(t4)*sin(t5)*sin(t6))/2000000 + (43*a2*d6*cos(t3)*cos(t4)*cos(t5))/100 - (43*a2*d6*cos(t5)*sin(t3)*sin(t4))/100) + td3*((3786513411*cos(t5)*sin(t5))/5000000000000 - (713241*cos(t5)^2*sin(t6))/100000000000 + (713241*sin(t5)^2*sin(t6))/100000000000 - (784477*cos(t5)*cos(t6)^2*sin(t5))/40000000000 + (582539*a3*cos(t4)*cos(t5))/50000000 - (37539*d6*cos(t5)*sin(t5))/2500000 + (43*d6^2*cos(t5)*sin(t5))/100 + (817*d6*cos(t5)^2*sin(t6))/2000000 - (817*d6*sin(t5)^2*sin(t6))/2000000 + (582539*a2*cos(t3)*cos(t4)*cos(t5))/50000000 - (582539*a2*cos(t5)*sin(t3)*sin(t4))/50000000 - (817*a3*cos(t4)*sin(t5)*sin(t6))/2000000 + (43*a3*d6*cos(t4)*cos(t5))/100 - (817*a2*cos(t3)*cos(t4)*sin(t5)*sin(t6))/2000000 + (817*a2*sin(t3)*sin(t4)*sin(t5)*sin(t6))/2000000 + (43*a2*d6*cos(t3)*cos(t4)*cos(t5))/100 - (43*a2*d6*cos(t5)*sin(t3)*sin(t4))/100) + td4*((3786513411*cos(t5)*sin(t5))/5000000000000 - (713241*cos(t5)^2*sin(t6))/100000000000 + (713241*sin(t5)^2*sin(t6))/100000000000 - (784477*cos(t5)*cos(t6)^2*sin(t5))/40000000000 + (582539*a3*cos(t4)*cos(t5))/50000000 - (37539*d6*cos(t5)*sin(t5))/2500000 + (43*d6^2*cos(t5)*sin(t5))/100 + (817*d6*cos(t5)^2*sin(t6))/2000000 - (817*d6*sin(t5)^2*sin(t6))/2000000 + (582539*a2*cos(t3)*cos(t4)*cos(t5))/50000000 - (582539*a2*cos(t5)*sin(t3)*sin(t4))/50000000 - (817*a3*cos(t4)*sin(t5)*sin(t6))/2000000 + (43*a3*d6*cos(t4)*cos(t5))/100 - (817*a2*cos(t3)*cos(t4)*sin(t5)*sin(t6))/2000000 + (817*a2*sin(t3)*sin(t4)*sin(t5)*sin(t6))/2000000 + (43*a2*d6*cos(t3)*cos(t4)*cos(t5))/100 - (43*a2*d6*cos(t5)*sin(t3)*sin(t4))/100) + td1*((49450651*sin(t2 + t3 + t4 - t5))/250000000000 - (7474967197*sin(t2 + t3 + t4 - 2*t5))/40000000000000 - (7474967197*sin(t2 + t3 + t4 + 2*t5))/40000000000000 + (784477*sin(t2 + t3 + t4 - 2*t6))/320000000000 + (784477*sin(t2 + t3 + t4 + 2*t6))/320000000000 + (713241*sin(t2 + t3 + t4 + t5 + t6))/400000000000 + (33478847947*sin(t2 + t3 + t4))/20000000000000 + (713241*sin(t2 + t3 + t4 + t5 - t6))/400000000000 - (713241*sin(t2 + t3 + t4 - t5 + t6))/400000000000 - (784477*sin(t2 + t3 + t4 + t5 - 2*t6))/320000000000 + (784477*sin(t2 + t3 + t4 + t5 + 2*t6))/320000000000 - (713241*sin(t2 + t3 + t4 - 2*t5 + t6))/400000000000 + (713241*sin(t2 + t3 + t4 + 2*t5 + t6))/400000000000 - (49450651*sin(t2 + t3 + t4 + t5))/250000000000 - (713241*sin(t2 + t3 + t4 - t5 - t6))/400000000000 - (784477*sin(t2 + t3 + t4 - t5 - 2*t6))/320000000000 + (784477*sin(t2 + t3 + t4 - t5 + 2*t6))/320000000000 + (713241*sin(t2 + t3 + t4 - 2*t5 - t6))/400000000000 - (713241*sin(t2 + t3 + t4 + 2*t5 - t6))/400000000000 + (784477*sin(t2 + t3 + t4 - 2*t5 - 2*t6))/640000000000 + (784477*sin(t2 + t3 + t4 - 2*t5 + 2*t6))/640000000000 + (784477*sin(t2 + t3 + t4 + 2*t5 - 2*t6))/640000000000 + (784477*sin(t2 + t3 + t4 + 2*t5 + 2*t6))/640000000000 + (817*a3*cos(t2 + t3 - t5 - t6))/8000000 - (43*d6^2*sin(t2 + t3 + t4 - 2*t5))/400 - (43*d6^2*sin(t2 + t3 + t4 + 2*t5))/400 - (817*d5*sin(t2 + t3 + t4 + t5 - t6))/8000000 + (817*d5*sin(t2 + t3 + t4 - t5 + t6))/8000000 - (817*d6*sin(t2 + t3 + t4 + t5 - t6))/8000000 + (817*d6*sin(t2 + t3 + t4 - t5 + t6))/8000000 + (817*d6*sin(t2 + t3 + t4 - 2*t5 + t6))/8000000 - (817*d6*sin(t2 + t3 + t4 + 2*t5 + t6))/8000000 + (582539*a3*cos(t2 + t3 - t5))/100000000 + (817*a2*cos(t2 + t5 - t6))/8000000 - (817*a2*cos(t2 - t5 + t6))/8000000 + (817*a2*cos(t5 - t2 + t6))/8000000 + (43*d6^2*sin(t2 + t3 + t4))/200 - (817*a3*cos(t2 + t3 + t5 + t6))/8000000 + (582539*d5*sin(t2 + t3 + t4 + t5))/100000000 - (582539*a2*cos(t2 + t5))/100000000 - (817*d5*sin(t2 + t3 + t4 - t5 - t6))/8000000 + (817*d6*sin(t2 + t3 + t4 - t5 - t6))/8000000 - (817*d6*sin(t2 + t3 + t4 - 2*t5 - t6))/8000000 + (817*d6*sin(t2 + t3 + t4 + 2*t5 - t6))/8000000 + (817*a3*cos(t2 + t3 + t5 - t6))/8000000 - (817*a3*cos(t2 + t3 - t5 + t6))/8000000 - (582539*d5*sin(t2 + t3 + t4 - t5))/100000000 + (37539*d6*sin(t2 + t3 + t4 - 2*t5))/10000000 + (37539*d6*sin(t2 + t3 + t4 + 2*t5))/10000000 + (582539*a2*cos(t2 - t5))/100000000 + (817*d5*sin(t2 + t3 + t4 + t5 + t6))/8000000 - (817*d6*sin(t2 + t3 + t4 + t5 + t6))/8000000 - (582539*a3*cos(t2 + t3 + t5))/100000000 - (817*a2*cos(t2 + t5 + t6))/8000000 - (37539*d6*sin(t2 + t3 + t4))/5000000 - (43*d5*d6*sin(t2 + t3 + t4 - t5))/200 + (43*a2*d6*cos(t2 - t5))/200 - (43*a3*d6*cos(t2 + t3 + t5))/200 + (43*a3*d6*cos(t2 + t3 - t5))/200 + (43*d5*d6*sin(t2 + t3 + t4 + t5))/200 - (43*a2*d6*cos(t2 + t5))/200) - td6*((16015523*sin(t5))/80000000000 - (784477*cos(t6)^2*sin(t5))/80000000000 + (784477*sin(t5)*sin(t6)^2)/80000000000 - (817*d5*cos(t6)*sin(t5))/2000000 + (817*a3*cos(t6)*sin(t4)*sin(t5))/2000000 + (817*a2*cos(t3)*cos(t6)*sin(t4)*sin(t5))/2000000 + (817*a2*cos(t4)*cos(t6)*sin(t3)*sin(t5))/2000000) - td5*((49450651*sin(t5))/125000000000 - (713241*cos(t6)*sin(t5))/100000000000 - (582539*d5*sin(t5))/50000000 - (43*d5*d6*sin(t5))/100 - (817*d5*cos(t5)*sin(t6))/2000000 + (817*d6*cos(t6)*sin(t5))/2000000 + (582539*a3*sin(t4)*sin(t5))/50000000 - (784477*cos(t5)*cos(t6)*sin(t6))/40000000000 + (582539*a2*cos(t3)*sin(t4)*sin(t5))/50000000 + (582539*a2*cos(t4)*sin(t3)*sin(t5))/50000000 + (817*a3*cos(t5)*sin(t4)*sin(t6))/2000000 + (43*a3*d6*sin(t4)*sin(t5))/100 + (817*a2*cos(t3)*cos(t5)*sin(t4)*sin(t6))/2000000 + (817*a2*cos(t4)*cos(t5)*sin(t3)*sin(t6))/2000000 + (43*a2*d6*cos(t3)*sin(t4)*sin(t5))/100 + (43*a2*d6*cos(t4)*sin(t3)*sin(t5))/100);

c26=- td2*((784477*cos(t5)^2*cos(t6)*sin(t6))/40000000000 - (817*d5*sin(t6))/2000000 - (784477*cos(t6)*sin(t6))/40000000000 + (817*a3*sin(t4)*sin(t6))/2000000 + (713241*cos(t5)*cos(t6)*sin(t5))/100000000000 - (817*a3*cos(t4)*cos(t5)*cos(t6))/2000000 - (817*d6*cos(t5)*cos(t6)*sin(t5))/2000000 + (817*a2*cos(t3)*sin(t4)*sin(t6))/2000000 + (817*a2*cos(t4)*sin(t3)*sin(t6))/2000000 - (817*a2*cos(t3)*cos(t4)*cos(t5)*cos(t6))/2000000 + (817*a2*cos(t5)*cos(t6)*sin(t3)*sin(t4))/2000000) - td3*((784477*cos(t5)^2*cos(t6)*sin(t6))/40000000000 - (817*d5*sin(t6))/2000000 - (784477*cos(t6)*sin(t6))/40000000000 + (817*a3*sin(t4)*sin(t6))/2000000 + (713241*cos(t5)*cos(t6)*sin(t5))/100000000000 - (817*a3*cos(t4)*cos(t5)*cos(t6))/2000000 - (817*d6*cos(t5)*cos(t6)*sin(t5))/2000000 + (817*a2*cos(t3)*sin(t4)*sin(t6))/2000000 + (817*a2*cos(t4)*sin(t3)*sin(t6))/2000000 - (817*a2*cos(t3)*cos(t4)*cos(t5)*cos(t6))/2000000 + (817*a2*cos(t5)*cos(t6)*sin(t3)*sin(t4))/2000000) - td4*((784477*cos(t5)^2*cos(t6)*sin(t6))/40000000000 - (817*d5*sin(t6))/2000000 - (784477*cos(t6)*sin(t6))/40000000000 + (817*a3*sin(t4)*sin(t6))/2000000 + (713241*cos(t5)*cos(t6)*sin(t5))/100000000000 - (817*a3*cos(t4)*cos(t5)*cos(t6))/2000000 - (817*d6*cos(t5)*cos(t6)*sin(t5))/2000000 + (817*a2*cos(t3)*sin(t4)*sin(t6))/2000000 + (817*a2*cos(t4)*sin(t3)*sin(t6))/2000000 - (817*a2*cos(t3)*cos(t4)*cos(t5)*cos(t6))/2000000 + (817*a2*cos(t5)*cos(t6)*sin(t3)*sin(t4))/2000000) - td6*((713241*cos(t6)*sin(t5))/100000000000 - (817*a3*cos(t4)*cos(t6))/2000000 - (817*d5*cos(t5)*sin(t6))/2000000 - (817*d6*cos(t6)*sin(t5))/2000000 - (817*a2*cos(t3)*cos(t4)*cos(t6))/2000000 + (817*a2*cos(t6)*sin(t3)*sin(t4))/2000000 + (817*a3*cos(t5)*sin(t4)*sin(t6))/2000000 + (817*a2*cos(t3)*cos(t5)*sin(t4)*sin(t6))/2000000 + (817*a2*cos(t4)*cos(t5)*sin(t3)*sin(t6))/2000000) - td5*((16015523*sin(t5))/80000000000 - (784477*cos(t6)^2*sin(t5))/80000000000 + (784477*sin(t5)*sin(t6)^2)/80000000000 - (817*d5*cos(t6)*sin(t5))/2000000 + (817*a3*cos(t6)*sin(t4)*sin(t5))/2000000 + (817*a2*cos(t3)*cos(t6)*sin(t4)*sin(t5))/2000000 + (817*a2*cos(t4)*cos(t6)*sin(t3)*sin(t5))/2000000) - td1*((713241*sin(t2 + t3 + t4 + t5 - t6))/800000000000 - (713241*sin(t2 + t3 + t4 + t5 + t6))/800000000000 - (713241*sin(t2 + t3 + t4 - t5 + t6))/800000000000 - (784477*sin(t2 + t3 + t4 + t5 - 2*t6))/320000000000 - (784477*sin(t2 + t3 + t4 + t5 + 2*t6))/320000000000 - (713241*sin(t2 + t3 + t4 - 2*t5 + t6))/800000000000 - (713241*sin(t2 + t3 + t4 + 2*t5 + t6))/800000000000 + (713241*sin(t2 + t3 + t4 - t5 - t6))/800000000000 + (784477*sin(t2 + t3 + t4 - t5 - 2*t6))/320000000000 + (784477*sin(t2 + t3 + t4 - t5 + 2*t6))/320000000000 - (713241*sin(t2 + t3 + t4 - 2*t5 - t6))/800000000000 - (713241*sin(t2 + t3 + t4 + 2*t5 - t6))/800000000000 - (784477*sin(t2 + t3 + t4 - 2*t5 - 2*t6))/640000000000 + (784477*sin(t2 + t3 + t4 - 2*t5 + 2*t6))/640000000000 + (784477*sin(t2 + t3 + t4 + 2*t5 - 2*t6))/640000000000 - (784477*sin(t2 + t3 + t4 + 2*t5 + 2*t6))/640000000000 - (817*a3*cos(t2 + t3 - t5 - t6))/16000000 + (817*d4*sin(t2 + t3 + t4 + t5 - t6))/16000000 + (817*d4*sin(t2 + t3 + t4 - t5 + t6))/16000000 - (817*d5*sin(t2 + t3 + t4 + t5 - t6))/16000000 + (817*d5*sin(t2 + t3 + t4 - t5 + t6))/16000000 - (817*d6*sin(t2 + t3 + t4 + t5 - t6))/16000000 + (817*d6*sin(t2 + t3 + t4 - t5 + t6))/16000000 + (817*d6*sin(t2 + t3 + t4 - 2*t5 + t6))/16000000 + (817*d6*sin(t2 + t3 + t4 + 2*t5 + t6))/16000000 + (817*a2*cos(t2 + t5 - t6))/16000000 - (817*a2*cos(t2 - t5 + t6))/16000000 - (817*a2*cos(t5 - t2 + t6))/16000000 + (817*a3*cos(t2 + t3 + t5 + t6))/16000000 + (817*d4*sin(t2 + t3 + t4 + t6))/8000000 + (817*d4*sin(t2 + t3 + t4 - t5 - t6))/16000000 + (817*d5*sin(t2 + t3 + t4 - t5 - t6))/16000000 - (817*d6*sin(t2 + t3 + t4 - t5 - t6))/16000000 + (817*d6*sin(t2 + t3 + t4 - 2*t5 - t6))/16000000 + (817*d6*sin(t2 + t3 + t4 + 2*t5 - t6))/16000000 + (817*a3*cos(t2 + t3 + t5 - t6))/16000000 - (817*a3*cos(t2 + t3 - t5 + t6))/16000000 - (817*d4*sin(t2 + t3 + t4 - t6))/8000000 + (817*d4*sin(t2 + t3 + t4 + t5 + t6))/16000000 - (817*d5*sin(t2 + t3 + t4 + t5 + t6))/16000000 + (817*d6*sin(t2 + t3 + t4 + t5 + t6))/16000000 + (817*a2*cos(t2 + t5 + t6))/16000000 - (817*a2*cos(t6)*sin(t2)*sin(t5))/4000000 + (16015523*cos(t2)*cos(t3)*cos(t4)*sin(t5))/80000000000 + (713241*cos(t2)*cos(t3)*cos(t6)*sin(t4))/200000000000 + (713241*cos(t2)*cos(t4)*cos(t6)*sin(t3))/200000000000 + (713241*cos(t3)*cos(t4)*cos(t6)*sin(t2))/200000000000 - (16015523*cos(t2)*sin(t3)*sin(t4)*sin(t5))/80000000000 - (16015523*cos(t3)*sin(t2)*sin(t4)*sin(t5))/80000000000 - (16015523*cos(t4)*sin(t2)*sin(t3)*sin(t5))/80000000000 - (713241*cos(t6)*sin(t2)*sin(t3)*sin(t4))/200000000000 - (817*d4*cos(t2)*cos(t3)*cos(t4)*sin(t6))/4000000 - (817*d6*cos(t2)*cos(t3)*cos(t6)*sin(t4))/4000000 - (817*d6*cos(t2)*cos(t4)*cos(t6)*sin(t3))/4000000 - (817*d6*cos(t3)*cos(t4)*cos(t6)*sin(t2))/4000000 - (817*a3*cos(t2)*cos(t6)*sin(t3)*sin(t5))/4000000 - (817*a3*cos(t3)*cos(t6)*sin(t2)*sin(t5))/4000000 + (817*d4*cos(t2)*sin(t3)*sin(t4)*sin(t6))/4000000 + (817*d4*cos(t3)*sin(t2)*sin(t4)*sin(t6))/4000000 + (817*d4*cos(t4)*sin(t2)*sin(t3)*sin(t6))/4000000 + (817*d6*cos(t6)*sin(t2)*sin(t3)*sin(t4))/4000000 + (713241*cos(t2)*cos(t3)*cos(t4)*cos(t5)*sin(t6))/200000000000 - (713241*cos(t2)*cos(t5)*sin(t3)*sin(t4)*sin(t6))/200000000000 - (713241*cos(t3)*cos(t5)*sin(t2)*sin(t4)*sin(t6))/200000000000 - (713241*cos(t4)*cos(t5)*sin(t2)*sin(t3)*sin(t6))/200000000000 - (817*d4*cos(t2)*cos(t3)*cos(t5)*cos(t6)*sin(t4))/4000000 - (817*d4*cos(t2)*cos(t4)*cos(t5)*cos(t6)*sin(t3))/4000000 - (817*d4*cos(t3)*cos(t4)*cos(t5)*cos(t6)*sin(t2))/4000000 - (817*d5*cos(t2)*cos(t3)*cos(t4)*cos(t6)*sin(t5))/4000000 - (817*d6*cos(t2)*cos(t3)*cos(t4)*cos(t5)*sin(t6))/4000000 + (817*d4*cos(t5)*cos(t6)*sin(t2)*sin(t3)*sin(t4))/4000000 + (817*d5*cos(t2)*cos(t6)*sin(t3)*sin(t4)*sin(t5))/4000000 + (817*d5*cos(t3)*cos(t6)*sin(t2)*sin(t4)*sin(t5))/4000000 + (817*d5*cos(t4)*cos(t6)*sin(t2)*sin(t3)*sin(t5))/4000000 + (817*d6*cos(t2)*cos(t5)*sin(t3)*sin(t4)*sin(t6))/4000000 + (817*d6*cos(t3)*cos(t5)*sin(t2)*sin(t4)*sin(t6))/4000000 + (817*d6*cos(t4)*cos(t5)*sin(t2)*sin(t3)*sin(t6))/4000000);

